simulink model "simulator_prototype_remade_v1"  (R2021b)
(part 6 of 14)

C_dq = ft_8({dq1,dq2,dq3,dq4,dq5,dq6,t1004,t1006,t1008,t1009,t101,t1010,t1012,t1013,t1016,t102,t1023,t1024,t1025,t1026,t1027,t1028,t1030,t1032,t1033,t1034,t1038,t1039,t1040,t1041,t1042,t1043,t1044,t1045,t1046,t1047,t1048,t1049,t1050,t1051,t1054,t1055,t1056,t1057,t1059,t1061,t1064,t1065,t1066,t1068,t1069,t1070,t1071,t1073,t1076,t1081,t1083,t1084,t1085,t1091,t1092,t1093,t1094,t1095,t1097,t1098,t1099,t110,t1101,t1102,t1105,t1106,t1107,t1108,t1109,t111,t1113,t1115,t1116,t1119,t112,t1120,t1122,t1123,t1125,t1126,t1127,t1128,t113,t1130,t1131,t1132,t1133,t1134,t1138,t1139,t114,t1140,t1141,t1144,t1146,t1148,t115,t1150,t1151,t1152,t1153,t1155,t1158,t1159,t116,t1161,t1162,t1163,t1166,t1167,t1169,t1170,t1171,t1173,t1174,t1175,t1176,t1177,t1178,t1179,t1180,t1181,t1182,t1183,t1184,t1185,t1186,t1187,t1188,t1189,t1190,t1191,t1192,t1193,t1195,t1196,t1197,t1198,t1199,t120,t1203,t1204,t1205,t1206,t1207,t1208,t121,t1210,t1215,t1219,t1221,t1222,t1223,t1224,t1225,t1226,t1227,t1228,t1229,t1230,t1232,t1233,t1236,t124,t1240,t1242,t1244,t1245,t125,t1250,t1251,t1253,t1254,t1256,t1257,t1258,t1259,t126,t1260,t1261,t1262,t1263,t1264,t1265,t1266,t1267,t1268,t1269,t1271,t1272,t1273,t1274,t1276,t1277,t1278,t1279,t128,t1280,t1282,t1285,t1286,t1287,t1288,t129,t1290,t1293,t1294,t1295,t1296,t1297,t1298,t130,t1300,t1301,t1302,t1306,t1307,t1308,t1309,t131,t1312,t1313,t1315,t1316,t1319,t132,t1320,t1321,t1322,t1323,t1324,t1325,t1326,t1328,t1329,t133,t1330,t1331,t1332,t1333,t1334,t1337,t1338,t1339,t134,t1340,t1341,t1342,t1343,t1344,t1345,t1346,t1347,t1348,t1351,t1352,t1353,t1354,t1355,t1356,t1358,t136,t1360,t1362,t1365,t1366,t1367,t1368,t1369,t1370,t1371,t1372,t1373,t1374,t1375,t1377,t1378,t1379,t1380,t1383,t1384,t1385,t1386,t1387,t1388,t1389,t139,t1391,t1392,t1393,t1394,t1397,t1398,t140,t1401,t1402,t1403,t1404,t1405,t1406,t1407,t1408,t1409,t141,t1410,t1411,t1413,t1414,t1415,t1416,t1417,t1418,t1419,t142,t1421,t1422,t1423,t1424,t1426,t1427,t1428,t1429,t143,t1430,t1431,t1432,t1433,t1434,t1436,t1439,t144,t1440,t1442,t1443,t1444,t1445,t1447,t1448,t1449,t145,t1451,t1452,t1453,t1454,t1455,t1456,t1457,t1458,t1459,t1460,t1463,t1464,t1467,t1468,t1469,t147,t1470,t1471,t1474,t1476,t1478,t1479,t148,t1480,t1481,t1482,t1483,t1485,t1486,t1487,t1488,t1489,t1492,t1494,t1496,t1498,t1499,t15,t150,t1501,t1503,t1505,t1506,t1508,t151,t1511,t1513,t1515,t1517,t1520,t1521,t1522,t1523,t1524,t1527,t1529,t153,t1530,t1531,t1532,t1533,t1534,t1535,t1536,t1537,t1538,t1539,t154,t1541,t1542,t1548,t1549,t1550,t1551,t1553,t1557,t1558,t156,t1560,t1561,t1562,t1566,t1567,t1568,t157,t1570,t1571,t1572,t1574,t1575,t1578,t158,t1580,t1581,t1587,t1589,t1590,t1591,t1592,t1593,t1594,t1595,t1596,t1597,t1598,t1599,t16,t1605,t1606,t1607,t1609,t161,t1610,t1611,t1612,t1613,t1614,t1615,t1617,t1618,t1619,t1620,t1621,t1622,t1624,t1625,t1627,t163,t1630,t1631,t1632,t1633,t1635,t1636,t1637,t1638,t1639,t1641,t1642,t1643,t1644,t1645,t1646,t1649,t165,t1651,t1652,t1653,t1657,t1658,t1659,t166,t1660,t1661,t1662,t1663,t1665,t1666,t1669,t1670,t1671,t1672,t1673,t1674,t1676,t1681,t1682,t1683,t1687,t1689,t1692,t1695,t1696,t1697,t1698,t17,t170,t1702,t1703,t1704,t1705,t1706,t1709,t171,t1711,t1712,t1713,t1716,t1719,t1720,t1722,t1724,t1726,t1728,t1729,t173,t1731,t1733,t1734,t1735,t1736,t1737,t1738,t1739,t1740,t1743,t1744,t1745,t1746,t1748,t1749,t175,t1752,t1755,t1756,t1757,t1758,t1759,t1760,t1761,t1763,t1764,t1767,t1769,t177,t1770,t1771,t1772,t1773,t1774,t1775,t1776,t1779,t1780,t1782,t1783,t1784,t1785,t1786,t1787,t1788,t1789,t1791,t1792,t1793,t1795,t1797,t1798,t1799,t18,t1800,t1801,t1802,t1804,t1806,t1807,t1808,t1809,t1810,t1811,t1812,t1813,t1814,t1816,t1817,t1820,t1822,t1823,t1824,t1825,t1826,t1827,t1828,t1829,t183,t1830,t1831,t1832,t1833,t1834,t1835,t1836,t1837,t1838,t1839,t1844,t1847,t1849,t185,t1850,t1851,t1854,t1855,t1857,t1858,t1859,t186,t1862,t1864,t1865,t1866,t1867,t1871,t1872,t1873,t1877,t1879,t1880,t1881,t1882,t1884,t1887,t1889,t1892,t1893,t1896,t19,t190,t1903,t1904,t1906,t1907,t1908,t1909,t191,t1910,t1911,t1912,t1913,t1914,t1915,t1916,t1919,t1920,t1921,t1925,t1926,t193,t1930,t1935,t1936,t1937,t1938,t1939,t1943,t1944,t1946,t1950,t1955,t196,t1961,t1966,t1967,t1968,t1969,t197,t1970,t1971,t1973,t1976,t1977,t1978,t1979,t1980,t1981,t1984,t1988,t199,t1992,t1993,t1994,t1995,t1996,t1997,t1998,t1999,t2,t20,t200,t2000,t2001,t2002,t2003,t2004,t2005,t2006,t2008,t201,t2014,t2016,t2017,t2019,t202,t2020,t2021,t2023,t2024,t2028,t2029,t2033,t2036,t2037,t2038,t204,t2040,t2041,t2042,t2044,t2047,t205,t2051,t2052,t2053,t2054,t2055,t2056,t2057,t2058,t2059,t206,t2060,t2061,t2062,t2065,t2066,t2067,t2068,t2069,t207,t2070,t2071,t2072,t2073,t2074,t2076,t2077,t2078,t2079,t2080,t2081,t2082,t2083,t2084,t2085,t2086,t2087,t2088,t2089,t2091,t2092,t2093,t2094,t2095,t2096,t2097,t2098,t2099,t21,t2100,t2101,t2103,t2104,t2105,t2106,t2107,t2108,t2109,t2110,t2111,t2113,t2114,t2115,t2116,t2117,t2118,t2119,t2121,t2125,t2128,t2129,t2130,t2131,t2132,t2133,t2135,t2136,t2139,t2140,t2141,t2142,t2144,t2147,t2148,t2149,t215,t2150,t2151,t2154,t2155,t2156,t2157,t2158,t2159,t2162,t2163,t2166,t2167,t2168,t2169,t2170,t2171,t2172,t2174,t2175,t2176,t2177,t2178,t2179,t2180,t2182,t2184,t2185,t2186,t2187,t2189,t2190,t2191,t2192,t2194,t2195,t2196,t22,t2200,t2201,t2203,t2204,t2208,t2209,t2210,t2212,t2214,t2217,t2218,t2219,t2220,t2221,t2223,t2225,t2227,t2228,t2229,t2231,t2232,t2236,t2237,t2239,t224,t2240,t2243,t2246,t2249,t225,t2250,t2251,t2252,t2254,t2255,t2256,t2257,t2264,t2265,t2266,t2267,t2269,t227,t2270,t2271,t2272,t2273,t2274,t2276,t2277,t2278,t2279,t228,t2280,t2281,t2282,t2283,t2284,t2285,t2286,t2287,t2291,t2292,t2294,t2295,t23,t230,t2302,t2304,t2305,t2306,t2307,t2308,t2309,t231,t2310,t2311,t2312,t2314,t2316,t2317,t2318,t2321,t2322,t2323,t2324,t233,t2331,t2333,t2334,t2335,t2336,t2337,t2338,t2339,t234,t2340,t2341,t2342,t2344,t2347,t2348,t235,t2350,t2351,t2355,t2357,t2358,t2359,t236,t2361,t2362,t2363,t2364,t2365,t2366,t2368,t2369,t2370,t2371,t2372,t2373,t2374,t2375,t2376,t2377,t2378,t2379,t2381,t2382,t2384,t2385,t2387,t2388,t2389,t239,t2390,t2391,t2392,t2394,t2395,t2396,t2397,t24,t240,t2400,t2401,t2402,t2403,t2405,t2406,t2407,t2410,t2417,t2421,t2422,t2423,t2425,t2427,t2428,t2429,t243,t2430,t2431,t2434,t2435,t2437,t2438,t2439,t244,t2440,t2441,t2442,t2443,t2444,t2445,t2446,t2449,t2450,t2452,t2453,t2454,t2455,t2456,t2457,t2458,t2459,t2460,t2461,t2463,t2464,t2466,t2467,t2469,t2470,t2471,t2472,t2474,t2477,t2478,t2480,t2481,t2482,t2483,t2484,t2485,t2486,t2487,t2489,t249,t2495,t2497,t25,t2500,t2502,t2503,t2505,t2506,t2507,t2508,t2509,t2510,t2511,t2512,t2513,t2517,t2518,t2519,t2520,t2521,t2522,t2523,t2524,t2525,t2526,t2527,t2530,t2531,t2532,t2533,t2535,t2536,t2537,t2539,t2540,t2541,t2543,t2544,t2545,t2546,t2548,t2549,t2550,t2552,t2553,t2554,t2555,t2556,t2560,t2562,t2563,t2564,t2565,t2566,t2567,t2568,t2569,t257,t2570,t2571,t2574,t2575,t2576,t2577,t2578,t2579,t258,t2580,t2581,t2582,t2585,t2586,t2587,t2588,t2589,t2590,t2595,t2597,t2598,t2599,t26,t2600,t2601,t2602,t2603,t2604,t2606,t2607,t2608,t2611,t2612,t2615,t2616,t2617,t2627,t263,t2633,t2634,t2636,t2639,t2640,t2641,t2654,t2655,t2656,t2659,t266,t2666,t2668,t2669,t2671,t2673,t2675,t2676,t2677,t2678,t2680,t2681,t2682,t2684,t2685,t2686,t2688,t2692,t2693,t2694,t2695,t2699,t270,t2702,t2703,t2705,t2706,t2707,t2708,t2719,t2720,t2721,t2722,t2723,t2724,t2725,t2726,t273,t2733,t2734,t2739,t274,t2741,t2742,t2743,t2744,t2748,t2749,t275,t2752,t2759,t276,t2760,t2761,t2762,t2764,t2768,t2769,t277,t2770,t2771,t2773,t2774,t2775,t2776,t278,t2781,t2782,t2783,t2784,t2786,t2787,t2788,t2789,t2791,t2792,t280,t2806,t2808,t2815,t2820,t2821,t2829,t2830,t2831,t284,t2840,t2842,t2844,t2845,t2847,t2848,t2849,t2853,t2854,t2861,t2862,t2863,t2864,t2866,t2868,t2869,t287,t2879,t2884,t2886,t2888,t2892,t2898,t2899,t29,t290,t2900,t2901,t2902,t2903,t2908,t291,t292,t2920,t2923,t2925,t2926,t2928,t2929,t2930,t2937,t294,t2940,t2943,t2945,t2948,t2949,t2950,t2951,t2952,t2960,t2961,t2962,t2963,t2964,t2966,t2967,t2968,t2969,t297,t2970,t2971,t2975,t2976,t2980,t2982,t2983,t2984,t2985,t2986,t2988,t2989,t299,t2991,t2992,t2993,t2996,t2997,t3,t30,t300,t3003,t3004,t3007,t3010,t3011,t3013,t3014,t3019,t302,t3020,t3021,t3023,t3024,t3025,t3027,t3028,t3029,t303,t3030,t3031,t3032,t3033,t3034,t3035,t3036,t3038,t3039,t304,t3043,t3045,t3046,t3047,t305,t3051,t3052,t3053,t3055,t3056,t3057,t306,t3060,t3061,t3062,t3063,t3065,t3066,t3069,t3070,t3071,t3072,t3073,t3075,t3077,t3078,t3079,t3080,t3082,t3083,t3085,t3087,t309,t3090,t3091,t3092,t3093,t3094,t3095,t3098,t3099,t310,t3103,t3104,t3105,t3108,t3109,t311,t3112,t3113,t3119,t3120,t3123,t3124,t3126,t3127,t313,t3130,t3131,t3132,t3133,t3139,t314,t3140,t3142,t3143,t3145,t3146,t3148,t3149,t315,t3150,t3151,t3152,t3156,t3157,t3158,t316,t3160,t3163,t3165,t3167,t3170,t3171,t3172,t3173,t3174,t3177,t3178,t318,t3180,t3182,t3183,t3184,t3186,t3187,t319,t3190,t3191,t3194,t3197,t3199,t320,t3206,t3207,t3208,t3218,t3219,t322,t3228,t3230,t3231,t3234,t3236,t324,t3240,t3241,t3242,t3243,t3244,t3245,t325,t3250,t3251,t3252,t3253,t3254,t3256,t3257,t3260,t3265,t3272,t3273,t3274,t3275,t3276,t3277,t3278,t3279,t328,t3280,t3282,t3283,t3284,t3285,t3286,t3287,t3288,t3289,t3290,t3291,t3292,t3293,t3295,t3296,t3297,t3298,t3299,t3301,t3302,t3303,t3304,t3306,t3307,t3308,t3309,t3310,t3312,t3313,t3314,t3315,t3317,t3318,t3320,t3321,t3324,t3325,t3326,t3327,t3328,t3329,t333,t3331,t3333,t3334,t3335,t3338,t3339,t3342,t3343,t3346,t3347,t3350,t336,t3362,t3363,t3364,t3365,t3366,t3367,t3368,t3369,t337,t3371,t3372,t3373,t3374,t3375,t3376,t3377,t3378,t3380,t3381,t3382,t3383,t3384,t3387,t3390,t3391,t3392,t3393,t3394,t3395,t3396,t3397,t3398,t3399,t34,t340,t3400,t3402,t3403,t3404,t3405,t3406,t3407,t3408,t3409,t3410,t3411,t3412,t3413,t3416,t3417,t3418,t3420,t3421,t3422,t3423,t3424,t3425,t3426,t3427,t3430,t3431,t3432,t3433,t3434,t3435,t3436,t3437,t3439,t344,t3440,t3441,t3442,t3443,t3444,t3445,t3446,t3447,t3449,t3450,t3453,t3454,t3455,t3456,t3457,t3458,t346,t3462,t3463,t3464,t3465,t3466,t3467,t3468,t3469,t347,t3470,t3471,t3472,t3473,t3474,t3475,t3476,t3479,t348,t3480,t3481,t3483,t3485,t3487,t3488,t3489,t349,t3490,t3491,t3492,t3493,t3494,t3496,t3497,t3498,t3499,t350,t3500,t3501,t3502,t3503,t3504,t3505,t3506,t3507,t3509,t3510,t3511,t3513,t3514,t3515,t3516,t3517,t3518,t352,t3521,t3522,t3523,t3527,t3528,t3529,t353,t3530,t3531,t3532,t3533,t3535,t3536,t3538,t3539,t3542,t3543,t3544,t3545,t3546,t3547,t3549,t3550,t3551,t3552,t3554,t3556,t3557,t3559,t356,t3560,t3562,t3563,t3564,t3567,t3568,t3569,t357,t3571,t3572,t3573,t3574,t3577,t3578,t358,t3582,t3583,t3584,t3585,t3586,t3587,t3589,t359,t3590,t3592,t3593,t3596,t3597,t3599,t3602,t3603,t3604,t3605,t3606,t3607,t3608,t3609,t361,t3610,t3611,t3612,t3614,t3615,t3616,t3617,t3618,t3619,t362,t3620,t3625,t3630,t3631,t3633,t3634,t3635,t3636,t3637,t3638,t3642,t3644,t3648,t365,t3652,t3653,t3654,t3655,t3656,t3657,t3658,t3659,t3660,t3662,t3663,t3666,t3667,t3668,t3676,t368,t3681,t3682,t3687,t3688,t369,t3690,t3691,t3693,t3694,t3695,t3696,t3697,t3699,t3700,t3701,t3702,t3704,t3705,t3706,t3707,t3708,t3709,t371,t3713,t3715,t3716,t3717,t372,t3720,t3721,t3723,t3724,t3725,t3726,t3728,t3729,t373,t3730,t3732,t3733,t3734,t3735,t3736,t3737,t3738,t374,t3743,t3744,t3745,t3746,t3747,t3750,t3752,t3756,t3757,t3758,t3766,t3768,t3769,t377,t3774,t3776,t3778,t378,t3780,t3783,t3784,t3785,t3786,t3787,t3789,t379,t3792,t3795,t3798,t380,t3800,t3803,t3804,t3805,t3806,t3810,t3811,t3813,t3814,t3815,t3816,t3817,t3819,t382,t3820,t3821,t3822,t3823,t3824,t3825,t3826,t3827,t3831,t3834,t3835,t3839,t384,t3843,t3849,t3850,t3851,t3852,t3853,t3855,t3857,t3858,t386,t3866,t3867,t3869,t387,t3870,t3877,t388,t3885,t3889,t3890,t3891,t3892,t3899,t391,t3912,t3913,t3915,t3917,t392,t3929,t3930,t3941,t3946,t3949,t395,t3950,t3951,t3952,t3953,t3958,t3959,t396,t3966,t3970,t3980,t3981,t3982,t3984,t3990,t4,t400,t4004,t4005,t4006,t401,t4010,t4011,t4014,t4015,t4016,t4017,t4018,t4019,t402,t4020,t4021,t4022,t4023,t4024,t4025,t4026,t4027,t4028,t4029,t403,t4036,t4039,t4040,t4041,t4042,t4045,t4046,t4047,t4048,t4051,t4053,t4054,t406,t4062,t4063,t4064,t4065,t4068,t4069,t4070,t4071,t4073,t4074,t4075,t4089,t4099,t410,t4103,t4105,t411,t4113,t4114,t4116,t4118,t4119,t412,t4123,t4124,t4125,t413,t4132,t414,t4140,t4142,t4143,t4144,t4145,t415,t4150,t4152,t4153,t416,t4162,t4164,t4165,t4166,t4169,t417,t4171,t4173,t4174,t4177,t4178,t4179,t418,t4180,t4181,t4183,t4184,t4185,t4186,t4188,t4190,t4195,t4196,t4197,t420,t4201,t4202,t4205,t4206,t4207,t4208,t4209,t4210,t4211,t4215,t4217,t4218,t4219,t422,t4220,t4221,t4223,t4224,t4225,t4226,t4228,t4229,t423,t4230,t4231,t4232,t4233,t4234,t4235,t424,t4241,t4242,t4243,t4244,t4245,t4246,t4247,t4248,t4249,t425,t4250,t4251,t4253,t4254,t4255,t4256,t4257,t4258,t4259,t4260,t4261,t4262,t4263,t427,t4273,t4274,t4275,t4276,t4278,t4279,t428,t4280,t4281,t4282,t4283,t4284,t4285,t4286,t4287,t4289,t429,t4290,t4291,t4292,t4293,t4295,t4296,t4297,t4298,t4299,t4300,t4301,t4302,t4303,t4304,t4305,t4306,t4308,t431,t4310,t4315,t4316,t4317,t4318,t432,t4321,t4323,t4324,t4325,t4326,t4327,t4328,t4329,t433,t4330,t4331,t4332,t4333,t4334,t4335,t4336,t4337,t4338,t4339,t434,t4340,t4342,t4344,t4345,t4346,t4347,t4348,t4349,t435,t4350,t4354,t4356,t4357,t436,t4362,t4363,t4365,t4366,t4368,t4369,t437,t4370,t4371,t4372,t4373,t4374,t4375,t4376,t4377,t4379,t438,t4380,t4382,t4383,t4384,t4385,t4386,t4387,t4388,t4389,t439,t4391,t4392,t4394,t4395,t4396,t4397,t4398,t4399,t44,t440,t4400,t4401,t4402,t4403,t4404,t4405,t4406,t4407,t4408,t4409,t441,t4410,t4411,t4412,t4413,t4414,t4415,t4416,t4417,t4418,t4419,t442,t4420,t4421,t4422,t4423,t4424,t4425,t4426,t4427,t4428,t4429,t4430,t4431,t4432,t4433,t4434,t4435,t4436,t4437,t4438,t4439,t444,t4440,t4442,t4443,t4444,t4445,t4446,t4447,t4448,t4449,t445,t4450,t4451,t4452,t4453,t4454,t4455,t4457,t4459,t4460,t4461,t4462,t4463,t4464,t4465,t4466,t4467,t4468,t4469,t4470,t4471,t4473,t4474,t4475,t4476,t4477,t4478,t4479,t448,t4480,t4481,t4482,t4483,t4484,t4485,t4486,t4487,t4488,t4489,t449,t4490,t4491,t4492,t4493,t4495,t4498,t45,t450,t4501,t4502,t4504,t4506,t4508,t4509,t4513,t4516,t4517,t4519,t452,t4520,t4522,t4524,t4525,t453,t4530,t4532,t4533,t454,t4540,t4542,t4543,t4547,t4548,t4549,t4551,t4554,t4555,t4557,t4558,t4559,t4561,t4562,t4563,t4566,t4567,t4568,t4569,t457,t4570,t4571,t4572,t4574,t4575,t4577,t4579,t458,t4581,t4582,t4583,t4584,t4588,t4589,t459,t4590,t4591,t4595,t4596,t46,t460,t4600,t4601,t4605,t4606,t4607,t461,t4611,t4614,t4616,t4617,t462,t4621,t4622,t4625,t4626,t4628,t4629,t463,t4630,t4632,t4633,t4634,t4636,t4637,t4638,t4639,t464,t4640,t4641,t4642,t4643,t4644,t4645,t4646,t4647,t4649,t465,t4650,t4651,t4652,t4653,t4656,t4657,t4658,t466,t4660,t4661,t4662,t4663,t4666,t4667,t4669,t4672,t4673,t4674,t4675,t468,t4688,t469,t4691,t4692,t4693,t4694,t4695,t4696,t4697,t47,t470,t4707,t4708,t4709,t471,t4711,t4713,t4716,t472,t4722,t4723,t4724,t4725,t4726,t4727,t4728,t4731,t4732,t4733,t4734,t4737,t4740,t4741,t4742,t4745,t4747,t4748,t4749,t475,t4752,t4753,t4754,t4755,t4756,t4758,t4759,t4760,t4761,t4763,t4766,t4769,t477,t4770,t4777,t4778,t4782,t4783,t4785,t4786,t4788,t4789,t479,t4790,t4794,t4795,t4796,t4797,t4798,t4799,t480,t4800,t4801,t4803,t4804,t4805,t4807,t4808,t481,t4811,t4813,t4814,t4815,t4818,t482,t4820,t4824,t4825,t4827,t4828,t483,t4830,t4832,t4833,t4834,t4835,t4837,t4839,t484,t4841,t4842,t4845,t4846,t4849,t485,t4852,t486,t4861,t4862,t4864,t4865,t4866,t4867,t4871,t4872,t4873,t4876,t4877,t4878,t4879,t488,t4882,t4883,t4884,t4886,t4887,t489,t4895,t4897,t4899,t4900,t4908,t4909,t491,t4910,t4911,t4913,t4915,t4916,t4919,t492,t4920,t4923,t4924,t4925,t4927,t4928,t493,t4930,t4933,t4934,t4937,t4938,t494,t4941,t4942,t4943,t4944,t4945,t4946,t4948,t4951,t4955,t4956,t4957,t496,t4962,t4964,t4969,t497,t4970,t4973,t4974,t4976,t498,t4980,t4981,t4982,t4983,t4986,t4987,t4988,t499,t4991,t4993,t4996,t4998,t4999,t5,t50,t500,t5000,t5001,t5004,t5006,t5008,t501,t5019,t502,t5021,t5022,t5023,t5026,t5027,t5029,t503,t5034,t5035,t5036,t5038,t504,t5045,t5046,t505,t5051,t5052,t5053,t506,t5060,t5062,t5063,t5064,t5065,t5066,t5069,t507,t5071,t5072,t5073,t5078,t508,t5080,t5082,t5083,t5084,t5085,t509,t5091,t5093,t5095,t5096,t5097,t5098,t5099,t510,t5100,t5102,t5107,t511,t5111,t5112,t5113,t5114,t5116,t5119,t512,t5120,t5122,t5127,t513,t5130,t5139,t514,t5142,t5147,t5149,t5150,t5151,t5154,t5158,t516,t5165,t517,t5171,t5172,t5176,t5179,t518,t5180,t5181,t5183,t5184,t5185,t5186,t5187,t5192,t5193,t5199,t520,t5200,t5203,t5204,t5205,t5208,t521,t5215,t5216,t5217,t522,t5222,t5223,t5224,t5227,t523,t5236,t5237,t5238,t5239,t524,t5240,t5244,t5245,t525,t5250,t5252,t5258,t526,t5267,t527,t5270,t5271,t5279,t528,t5280,t5281,t5285,t529,t5293,t5294,t53,t530,t5305,t531,t5318,t5319,t532,t5321,t5324,t5325,t5327,t5328,t533,t5331,t5332,t534,t535,t5353,t5355,t5356,t5358,t536,t5361,t5362,t5364,t5368,t537,t5372,t5373,t5376,t5378,t538,t5387,t5389,t539,t5390,t5391,t5392,t5393,t5394,t540,t5402,t5404,t5409,t5416,t5420,t5424,t5429,t543,t5430,t5434,t5435,t5436,t5439,t544,t5440,t5441,t5445,t5449,t545,t5450,t5451,t5452,t5453,t5455,t5456,t5457,t546,t5467,t5468,t5469,t547,t5470,t5471,t5472,t5473,t5474,t5475,t5476,t5477,t5478,t548,t5489,t549,t5490,t5493,t5494,t5497,t5499,t5501,t5508,t551,t5510,t5512,t5516,t5517,t552,t5521,t553,t5532,t5535,t554,t5540,t5547,t555,t5557,t5558,t556,t557,t5574,t5578,t5579,t558,t5582,t5586,t559,t5590,t5593,t5596,t560,t5604,t5607,t561,t5612,t562,t5629,t563,t5634,t5635,t564,t567,t568,t5688,t569,t57,t570,t571,t572,t573,t574,t5741,t5743,t576,t577,t5777,t5779,t578,t5780,t5782,t579,t58,t580,t581,t582,t5826,t583,t584,t586,t587,t5886,t5887,t589,t5894,t59,t590,t591,t592,t593,t594,t595,t596,t597,t6,t60,t600,t602,t603,t604,t605,t609,t610,t611,t612,t613,t614,t615,t616,t618,t619,t622,t623,t624,t625,t626,t627,t628,t629,t63,t630,t631,t633,t634,t635,t636,t637,t638,t639,t640,t641,t642,t643,t648,t649,t650,t653,t654,t655,t656,t657,t658,t660,t662,t663,t664,t665,t667,t668,t673,t674,t675,t676,t678,t679,t681,t682,t683,t684,t685,t686,t687,t688,t689,t693,t694,t695,t696,t697,t698,t7,t700,t702,t703,t704,t705,t706,t71,t710,t711,t712,t713,t715,t716,t72,t724,t728,t73,t731,t733,t734,t735,t736,t74,t741,t742,t743,t744,t746,t747,t748,t749,t75,t750,t751,t752,t754,t755,t756,t757,t758,t759,t76,t760,t762,t763,t764,t765,t766,t767,t768,t769,t77,t772,t773,t774,t775,t776,t777,t778,t779,t780,t781,t782,t784,t785,t786,t790,t792,t794,t795,t796,t798,t8,t80,t801,t804,t805,t806,t808,t81,t814,t815,t817,t82,t820,t822,t825,t827,t83,t831,t832,t833,t834,t835,t836,t837,t838,t84,t840,t841,t842,t843,t846,t86,t863,t868,t869,t870,t874,t878,t880,t881,t882,t884,t885,t888,t889,t891,t892,t895,t899,t9,t90,t900,t903,t906,t91,t911,t921,t922,t923,t925,t926,t927,t929,t934,t935,t936,t937,t940,t941,t942,t946,t949,t95,t950,t954,t955,t957,t958,t961,t962,t964,t965,t968,t97,t970,t971,t972,t973,t975,t977,t982,t983,t984,t986,t987,t988,t989,t99,t993,t994,t995,t999});
end
function C_dq = ft_8(ct)
dq1 = ct{1};
dq2 = ct{2};
dq3 = ct{3};
dq4 = ct{4};
dq5 = ct{5};
dq6 = ct{6};
t1004 = ct{7};
t1006 = ct{8};
t1008 = ct{9};
t1009 = ct{10};
t101 = ct{11};
t1010 = ct{12};
t1012 = ct{13};
t1013 = ct{14};
t1016 = ct{15};
t102 = ct{16};
t1023 = ct{17};
t1024 = ct{18};
t1025 = ct{19};
t1026 = ct{20};
t1027 = ct{21};
t1028 = ct{22};
t1030 = ct{23};
t1032 = ct{24};
t1033 = ct{25};
t1034 = ct{26};
t1038 = ct{27};
t1039 = ct{28};
t1040 = ct{29};
t1041 = ct{30};
t1042 = ct{31};
t1043 = ct{32};
t1044 = ct{33};
t1045 = ct{34};
t1046 = ct{35};
t1047 = ct{36};
t1048 = ct{37};
t1049 = ct{38};
t1050 = ct{39};
t1051 = ct{40};
t1054 = ct{41};
t1055 = ct{42};
t1056 = ct{43};
t1057 = ct{44};
t1059 = ct{45};
t1061 = ct{46};
t1064 = ct{47};
t1065 = ct{48};
t1066 = ct{49};
t1068 = ct{50};
t1069 = ct{51};
t1070 = ct{52};
t1071 = ct{53};
t1073 = ct{54};
t1076 = ct{55};
t1081 = ct{56};
t1083 = ct{57};
t1084 = ct{58};
t1085 = ct{59};
t1091 = ct{60};
t1092 = ct{61};
t1093 = ct{62};
t1094 = ct{63};
t1095 = ct{64};
t1097 = ct{65};
t1098 = ct{66};
t1099 = ct{67};
t110 = ct{68};
t1101 = ct{69};
t1102 = ct{70};
t1105 = ct{71};
t1106 = ct{72};
t1107 = ct{73};
t1108 = ct{74};
t1109 = ct{75};
t111 = ct{76};
t1113 = ct{77};
t1115 = ct{78};
t1116 = ct{79};
t1119 = ct{80};
t112 = ct{81};
t1120 = ct{82};
t1122 = ct{83};
t1123 = ct{84};
t1125 = ct{85};
t1126 = ct{86};
t1127 = ct{87};
t1128 = ct{88};
t113 = ct{89};
t1130 = ct{90};
t1131 = ct{91};
t1132 = ct{92};
t1133 = ct{93};
t1134 = ct{94};
t1138 = ct{95};
t1139 = ct{96};
t114 = ct{97};
t1140 = ct{98};
t1141 = ct{99};
t1144 = ct{100};
t1146 = ct{101};
t1148 = ct{102};
t115 = ct{103};
t1150 = ct{104};
t1151 = ct{105};
t1152 = ct{106};
t1153 = ct{107};
t1155 = ct{108};
t1158 = ct{109};
t1159 = ct{110};
t116 = ct{111};
t1161 = ct{112};
t1162 = ct{113};
t1163 = ct{114};
t1166 = ct{115};
t1167 = ct{116};
t1169 = ct{117};
t1170 = ct{118};
t1171 = ct{119};
t1173 = ct{120};
t1174 = ct{121};
t1175 = ct{122};
t1176 = ct{123};
t1177 = ct{124};
t1178 = ct{125};
t1179 = ct{126};
t1180 = ct{127};
t1181 = ct{128};
t1182 = ct{129};
t1183 = ct{130};
t1184 = ct{131};
t1185 = ct{132};
t1186 = ct{133};
t1187 = ct{134};
t1188 = ct{135};
t1189 = ct{136};
t1190 = ct{137};
t1191 = ct{138};
t1192 = ct{139};
t1193 = ct{140};
t1195 = ct{141};
t1196 = ct{142};
t1197 = ct{143};
t1198 = ct{144};
t1199 = ct{145};
t120 = ct{146};
t1203 = ct{147};
t1204 = ct{148};
t1205 = ct{149};
t1206 = ct{150};
t1207 = ct{151};
t1208 = ct{152};
t121 = ct{153};
t1210 = ct{154};
t1215 = ct{155};
t1219 = ct{156};
t1221 = ct{157};
t1222 = ct{158};
t1223 = ct{159};
t1224 = ct{160};
t1225 = ct{161};
t1226 = ct{162};
t1227 = ct{163};
t1228 = ct{164};
t1229 = ct{165};
t1230 = ct{166};
t1232 = ct{167};
t1233 = ct{168};
t1236 = ct{169};
t124 = ct{170};
t1240 = ct{171};
t1242 = ct{172};
t1244 = ct{173};
t1245 = ct{174};
t125 = ct{175};
t1250 = ct{176};
t1251 = ct{177};
t1253 = ct{178};
t1254 = ct{179};
t1256 = ct{180};
t1257 = ct{181};
t1258 = ct{182};
t1259 = ct{183};
t126 = ct{184};
t1260 = ct{185};
t1261 = ct{186};
t1262 = ct{187};
t1263 = ct{188};
t1264 = ct{189};
t1265 = ct{190};
t1266 = ct{191};
t1267 = ct{192};
t1268 = ct{193};
t1269 = ct{194};
t1271 = ct{195};
t1272 = ct{196};
t1273 = ct{197};
t1274 = ct{198};
t1276 = ct{199};
t1277 = ct{200};
t1278 = ct{201};
t1279 = ct{202};
t128 = ct{203};
t1280 = ct{204};
t1282 = ct{205};
t1285 = ct{206};
t1286 = ct{207};
t1287 = ct{208};
t1288 = ct{209};
t129 = ct{210};
t1290 = ct{211};
t1293 = ct{212};
t1294 = ct{213};
t1295 = ct{214};
t1296 = ct{215};
t1297 = ct{216};
t1298 = ct{217};
t130 = ct{218};
t1300 = ct{219};
t1301 = ct{220};
t1302 = ct{221};
t1306 = ct{222};
t1307 = ct{223};
t1308 = ct{224};
t1309 = ct{225};
t131 = ct{226};
t1312 = ct{227};
t1313 = ct{228};
t1315 = ct{229};
t1316 = ct{230};
t1319 = ct{231};
t132 = ct{232};
t1320 = ct{233};
t1321 = ct{234};
t1322 = ct{235};
t1323 = ct{236};
t1324 = ct{237};
t1325 = ct{238};
t1326 = ct{239};
t1328 = ct{240};
t1329 = ct{241};
t133 = ct{242};
t1330 = ct{243};
t1331 = ct{244};
t1332 = ct{245};
t1333 = ct{246};
t1334 = ct{247};
t1337 = ct{248};
t1338 = ct{249};
t1339 = ct{250};
t134 = ct{251};
t1340 = ct{252};
t1341 = ct{253};
t1342 = ct{254};
t1343 = ct{255};
t1344 = ct{256};
t1345 = ct{257};
t1346 = ct{258};
t1347 = ct{259};
t1348 = ct{260};
t1351 = ct{261};
t1352 = ct{262};
t1353 = ct{263};
t1354 = ct{264};
t1355 = ct{265};
t1356 = ct{266};
t1358 = ct{267};
t136 = ct{268};
t1360 = ct{269};
t1362 = ct{270};
t1365 = ct{271};
t1366 = ct{272};
t1367 = ct{273};
t1368 = ct{274};
t1369 = ct{275};
t1370 = ct{276};
t1371 = ct{277};
t1372 = ct{278};
t1373 = ct{279};
t1374 = ct{280};
t1375 = ct{281};
t1377 = ct{282};
t1378 = ct{283};
t1379 = ct{284};
t1380 = ct{285};
t1383 = ct{286};
t1384 = ct{287};
t1385 = ct{288};
t1386 = ct{289};
t1387 = ct{290};
t1388 = ct{291};
t1389 = ct{292};
t139 = ct{293};
t1391 = ct{294};
t1392 = ct{295};
t1393 = ct{296};
t1394 = ct{297};
t1397 = ct{298};
t1398 = ct{299};
t140 = ct{300};
t1401 = ct{301};
t1402 = ct{302};
t1403 = ct{303};
t1404 = ct{304};
t1405 = ct{305};
t1406 = ct{306};
t1407 = ct{307};
t1408 = ct{308};
t1409 = ct{309};
t141 = ct{310};
t1410 = ct{311};
t1411 = ct{312};
t1413 = ct{313};
t1414 = ct{314};
t1415 = ct{315};
t1416 = ct{316};
t1417 = ct{317};
t1418 = ct{318};
t1419 = ct{319};
t142 = ct{320};
t1421 = ct{321};
t1422 = ct{322};
t1423 = ct{323};
t1424 = ct{324};
t1426 = ct{325};
t1427 = ct{326};
t1428 = ct{327};
t1429 = ct{328};
t143 = ct{329};
t1430 = ct{330};
t1431 = ct{331};
t1432 = ct{332};
t1433 = ct{333};
t1434 = ct{334};
t1436 = ct{335};
t1439 = ct{336};
t144 = ct{337};
t1440 = ct{338};
t1442 = ct{339};
t1443 = ct{340};
t1444 = ct{341};
t1445 = ct{342};
t1447 = ct{343};
t1448 = ct{344};
t1449 = ct{345};
t145 = ct{346};
t1451 = ct{347};
t1452 = ct{348};
t1453 = ct{349};
t1454 = ct{350};
t1455 = ct{351};
t1456 = ct{352};
t1457 = ct{353};
t1458 = ct{354};
t1459 = ct{355};
t1460 = ct{356};
t1463 = ct{357};
t1464 = ct{358};
t1467 = ct{359};
t1468 = ct{360};
t1469 = ct{361};
t147 = ct{362};
t1470 = ct{363};
t1471 = ct{364};
t1474 = ct{365};
t1476 = ct{366};
t1478 = ct{367};
t1479 = ct{368};
t148 = ct{369};
t1480 = ct{370};
t1481 = ct{371};
t1482 = ct{372};
t1483 = ct{373};
t1485 = ct{374};
t1486 = ct{375};
t1487 = ct{376};
t1488 = ct{377};
t1489 = ct{378};
t1492 = ct{379};
t1494 = ct{380};
t1496 = ct{381};
t1498 = ct{382};
t1499 = ct{383};
t15 = ct{384};
t150 = ct{385};
t1501 = ct{386};
t1503 = ct{387};
t1505 = ct{388};
t1506 = ct{389};
t1508 = ct{390};
t151 = ct{391};
t1511 = ct{392};
t1513 = ct{393};
t1515 = ct{394};
t1517 = ct{395};
t1520 = ct{396};
t1521 = ct{397};
t1522 = ct{398};
t1523 = ct{399};
t1524 = ct{400};
t1527 = ct{401};
t1529 = ct{402};
t153 = ct{403};
t1530 = ct{404};
t1531 = ct{405};
t1532 = ct{406};
t1533 = ct{407};
t1534 = ct{408};
t1535 = ct{409};
t1536 = ct{410};
t1537 = ct{411};
t1538 = ct{412};
t1539 = ct{413};
t154 = ct{414};
t1541 = ct{415};
t1542 = ct{416};
t1548 = ct{417};
t1549 = ct{418};
t1550 = ct{419};
t1551 = ct{420};
t1553 = ct{421};
t1557 = ct{422};
t1558 = ct{423};
t156 = ct{424};
t1560 = ct{425};
t1561 = ct{426};
t1562 = ct{427};
t1566 = ct{428};
t1567 = ct{429};
t1568 = ct{430};
t157 = ct{431};
t1570 = ct{432};
t1571 = ct{433};
t1572 = ct{434};
t1574 = ct{435};
t1575 = ct{436};
t1578 = ct{437};
t158 = ct{438};
t1580 = ct{439};
t1581 = ct{440};
t1587 = ct{441};
t1589 = ct{442};
t1590 = ct{443};
t1591 = ct{444};
t1592 = ct{445};
t1593 = ct{446};
t1594 = ct{447};
t1595 = ct{448};
t1596 = ct{449};
t1597 = ct{450};
t1598 = ct{451};
t1599 = ct{452};
t16 = ct{453};
t1605 = ct{454};
t1606 = ct{455};
t1607 = ct{456};
t1609 = ct{457};
t161 = ct{458};
t1610 = ct{459};
t1611 = ct{460};
t1612 = ct{461};
t1613 = ct{462};
t1614 = ct{463};
t1615 = ct{464};
t1617 = ct{465};
t1618 = ct{466};
t1619 = ct{467};
t1620 = ct{468};
t1621 = ct{469};
t1622 = ct{470};
t1624 = ct{471};
t1625 = ct{472};
t1627 = ct{473};
t163 = ct{474};
t1630 = ct{475};
t1631 = ct{476};
t1632 = ct{477};
t1633 = ct{478};
t1635 = ct{479};
t1636 = ct{480};
t1637 = ct{481};
t1638 = ct{482};
t1639 = ct{483};
t1641 = ct{484};
t1642 = ct{485};
t1643 = ct{486};
t1644 = ct{487};
t1645 = ct{488};
t1646 = ct{489};
t1649 = ct{490};
t165 = ct{491};
t1651 = ct{492};
t1652 = ct{493};
t1653 = ct{494};
t1657 = ct{495};
t1658 = ct{496};
t1659 = ct{497};
t166 = ct{498};
t1660 = ct{499};
t1661 = ct{500};
t1662 = ct{501};
t1663 = ct{502};
t1665 = ct{503};
t1666 = ct{504};
t1669 = ct{505};
t1670 = ct{506};
t1671 = ct{507};
t1672 = ct{508};
t1673 = ct{509};
t1674 = ct{510};
t1676 = ct{511};
t1681 = ct{512};
t1682 = ct{513};
t1683 = ct{514};
t1687 = ct{515};
t1689 = ct{516};
t1692 = ct{517};
t1695 = ct{518};
t1696 = ct{519};
t1697 = ct{520};
t1698 = ct{521};
t17 = ct{522};
t170 = ct{523};
t1702 = ct{524};
t1703 = ct{525};
t1704 = ct{526};
t1705 = ct{527};
t1706 = ct{528};
t1709 = ct{529};
t171 = ct{530};
t1711 = ct{531};
t1712 = ct{532};
t1713 = ct{533};
t1716 = ct{534};
t1719 = ct{535};
t1720 = ct{536};
t1722 = ct{537};
t1724 = ct{538};
t1726 = ct{539};
t1728 = ct{540};
t1729 = ct{541};
t173 = ct{542};
t1731 = ct{543};
t1733 = ct{544};
t1734 = ct{545};
t1735 = ct{546};
t1736 = ct{547};
t1737 = ct{548};
t1738 = ct{549};
t1739 = ct{550};
t1740 = ct{551};
t1743 = ct{552};
t1744 = ct{553};
t1745 = ct{554};
t1746 = ct{555};
t1748 = ct{556};
t1749 = ct{557};
t175 = ct{558};
t1752 = ct{559};
t1755 = ct{560};
t1756 = ct{561};
t1757 = ct{562};
t1758 = ct{563};
t1759 = ct{564};
t1760 = ct{565};
t1761 = ct{566};
t1763 = ct{567};
t1764 = ct{568};
t1767 = ct{569};
t1769 = ct{570};
t177 = ct{571};
t1770 = ct{572};
t1771 = ct{573};
t1772 = ct{574};
t1773 = ct{575};
t1774 = ct{576};
t1775 = ct{577};
t1776 = ct{578};
t1779 = ct{579};
t1780 = ct{580};
t1782 = ct{581};
t1783 = ct{582};
t1784 = ct{583};
t1785 = ct{584};
t1786 = ct{585};
t1787 = ct{586};
t1788 = ct{587};
t1789 = ct{588};
t1791 = ct{589};
t1792 = ct{590};
t1793 = ct{591};
t1795 = ct{592};
t1797 = ct{593};
t1798 = ct{594};
t1799 = ct{595};
t18 = ct{596};
t1800 = ct{597};
t1801 = ct{598};
t1802 = ct{599};
t1804 = ct{600};
t1806 = ct{601};
t1807 = ct{602};
t1808 = ct{603};
t1809 = ct{604};
t1810 = ct{605};
t1811 = ct{606};
t1812 = ct{607};
t1813 = ct{608};
t1814 = ct{609};
t1816 = ct{610};
t1817 = ct{611};
t1820 = ct{612};
t1822 = ct{613};
t1823 = ct{614};
t1824 = ct{615};
t1825 = ct{616};
t1826 = ct{617};
t1827 = ct{618};
t1828 = ct{619};
t1829 = ct{620};
t183 = ct{621};
t1830 = ct{622};
t1831 = ct{623};
t1832 = ct{624};
t1833 = ct{625};
t1834 = ct{626};
t1835 = ct{627};
t1836 = ct{628};
t1837 = ct{629};
t1838 = ct{630};
t1839 = ct{631};
t1844 = ct{632};
t1847 = ct{633};
t1849 = ct{634};
t185 = ct{635};
t1850 = ct{636};
t1851 = ct{637};
t1854 = ct{638};
t1855 = ct{639};
t1857 = ct{640};
t1858 = ct{641};
t1859 = ct{642};
t186 = ct{643};
t1862 = ct{644};
t1864 = ct{645};
t1865 = ct{646};
t1866 = ct{647};
t1867 = ct{648};
t1871 = ct{649};
t1872 = ct{650};
t1873 = ct{651};
t1877 = ct{652};
t1879 = ct{653};
t1880 = ct{654};
t1881 = ct{655};
t1882 = ct{656};
t1884 = ct{657};
t1887 = ct{658};
t1889 = ct{659};
t1892 = ct{660};
t1893 = ct{661};
t1896 = ct{662};
t19 = ct{663};
t190 = ct{664};
t1903 = ct{665};
t1904 = ct{666};
t1906 = ct{667};
t1907 = ct{668};
t1908 = ct{669};
t1909 = ct{670};
t191 = ct{671};
t1910 = ct{672};
t1911 = ct{673};
t1912 = ct{674};
t1913 = ct{675};
t1914 = ct{676};
t1915 = ct{677};
t1916 = ct{678};
t1919 = ct{679};
t1920 = ct{680};
t1921 = ct{681};
t1925 = ct{682};
t1926 = ct{683};
t193 = ct{684};
t1930 = ct{685};
t1935 = ct{686};
t1936 = ct{687};
t1937 = ct{688};
t1938 = ct{689};
t1939 = ct{690};
t1943 = ct{691};
t1944 = ct{692};
t1946 = ct{693};
t1950 = ct{694};
t1955 = ct{695};
t196 = ct{696};
t1961 = ct{697};
t1966 = ct{698};
t1967 = ct{699};
t1968 = ct{700};
t1969 = ct{701};
t197 = ct{702};
t1970 = ct{703};
t1971 = ct{704};
t1973 = ct{705};
t1976 = ct{706};
t1977 = ct{707};
t1978 = ct{708};
t1979 = ct{709};
t1980 = ct{710};
t1981 = ct{711};
t1984 = ct{712};
t1988 = ct{713};
t199 = ct{714};
t1992 = ct{715};
t1993 = ct{716};
t1994 = ct{717};
t1995 = ct{718};
t1996 = ct{719};
t1997 = ct{720};
t1998 = ct{721};
t1999 = ct{722};
t2 = ct{723};
t20 = ct{724};
t200 = ct{725};
t2000 = ct{726};
t2001 = ct{727};
t2002 = ct{728};
t2003 = ct{729};
t2004 = ct{730};
t2005 = ct{731};
t2006 = ct{732};
t2008 = ct{733};
t201 = ct{734};
t2014 = ct{735};
t2016 = ct{736};
t2017 = ct{737};
t2019 = ct{738};
t202 = ct{739};
t2020 = ct{740};
t2021 = ct{741};
t2023 = ct{742};
t2024 = ct{743};
t2028 = ct{744};
t2029 = ct{745};
t2033 = ct{746};
t2036 = ct{747};
t2037 = ct{748};
t2038 = ct{749};
t204 = ct{750};
t2040 = ct{751};
t2041 = ct{752};
t2042 = ct{753};
t2044 = ct{754};
t2047 = ct{755};
t205 = ct{756};
t2051 = ct{757};
t2052 = ct{758};
t2053 = ct{759};
t2054 = ct{760};
t2055 = ct{761};
t2056 = ct{762};
t2057 = ct{763};
t2058 = ct{764};
t2059 = ct{765};
t206 = ct{766};
t2060 = ct{767};
t2061 = ct{768};
t2062 = ct{769};
t2065 = ct{770};
t2066 = ct{771};
t2067 = ct{772};
t2068 = ct{773};
t2069 = ct{774};
t207 = ct{775};
t2070 = ct{776};
t2071 = ct{777};
t2072 = ct{778};
t2073 = ct{779};
t2074 = ct{780};
t2076 = ct{781};
t2077 = ct{782};
t2078 = ct{783};
t2079 = ct{784};
t2080 = ct{785};
t2081 = ct{786};
t2082 = ct{787};
t2083 = ct{788};
t2084 = ct{789};
t2085 = ct{790};
t2086 = ct{791};
t2087 = ct{792};
t2088 = ct{793};
t2089 = ct{794};
t2091 = ct{795};
t2092 = ct{796};
t2093 = ct{797};
t2094 = ct{798};
t2095 = ct{799};
t2096 = ct{800};
t2097 = ct{801};
t2098 = ct{802};
t2099 = ct{803};
t21 = ct{804};
t2100 = ct{805};
t2101 = ct{806};
t2103 = ct{807};
t2104 = ct{808};
t2105 = ct{809};
t2106 = ct{810};
t2107 = ct{811};
t2108 = ct{812};
t2109 = ct{813};
t2110 = ct{814};
t2111 = ct{815};
t2113 = ct{816};
t2114 = ct{817};
t2115 = ct{818};
t2116 = ct{819};
t2117 = ct{820};
t2118 = ct{821};
t2119 = ct{822};
t2121 = ct{823};
t2125 = ct{824};
t2128 = ct{825};
t2129 = ct{826};
t2130 = ct{827};
t2131 = ct{828};
t2132 = ct{829};
t2133 = ct{830};
t2135 = ct{831};
t2136 = ct{832};
t2139 = ct{833};
t2140 = ct{834};
t2141 = ct{835};
t2142 = ct{836};
t2144 = ct{837};
t2147 = ct{838};
t2148 = ct{839};
t2149 = ct{840};
t215 = ct{841};
t2150 = ct{842};
t2151 = ct{843};
t2154 = ct{844};
t2155 = ct{845};
t2156 = ct{846};
t2157 = ct{847};
t2158 = ct{848};
t2159 = ct{849};
t2162 = ct{850};
t2163 = ct{851};
t2166 = ct{852};
t2167 = ct{853};
t2168 = ct{854};
t2169 = ct{855};
t2170 = ct{856};
t2171 = ct{857};
t2172 = ct{858};
t2174 = ct{859};
t2175 = ct{860};
t2176 = ct{861};
t2177 = ct{862};
t2178 = ct{863};
t2179 = ct{864};
t2180 = ct{865};
t2182 = ct{866};
t2184 = ct{867};
t2185 = ct{868};
t2186 = ct{869};
t2187 = ct{870};
t2189 = ct{871};
t2190 = ct{872};
t2191 = ct{873};
t2192 = ct{874};
t2194 = ct{875};
t2195 = ct{876};
t2196 = ct{877};
t22 = ct{878};
t2200 = ct{879};
t2201 = ct{880};
t2203 = ct{881};
t2204 = ct{882};
t2208 = ct{883};
t2209 = ct{884};
t2210 = ct{885};
t2212 = ct{886};
t2214 = ct{887};
t2217 = ct{888};
t2218 = ct{889};
t2219 = ct{890};
t2220 = ct{891};
t2221 = ct{892};
t2223 = ct{893};
t2225 = ct{894};
t2227 = ct{895};
t2228 = ct{896};
t2229 = ct{897};
t2231 = ct{898};
t2232 = ct{899};
t2236 = ct{900};
t2237 = ct{901};
t2239 = ct{902};
t224 = ct{903};
t2240 = ct{904};
t2243 = ct{905};
t2246 = ct{906};
t2249 = ct{907};
t225 = ct{908};
t2250 = ct{909};
t2251 = ct{910};
t2252 = ct{911};
t2254 = ct{912};
t2255 = ct{913};
t2256 = ct{914};
t2257 = ct{915};
t2264 = ct{916};
t2265 = ct{917};
t2266 = ct{918};
t2267 = ct{919};
t2269 = ct{920};
t227 = ct{921};
t2270 = ct{922};
t2271 = ct{923};
t2272 = ct{924};
t2273 = ct{925};
t2274 = ct{926};
t2276 = ct{927};
t2277 = ct{928};
t2278 = ct{929};
t2279 = ct{930};
t228 = ct{931};
t2280 = ct{932};
t2281 = ct{933};
t2282 = ct{934};
t2283 = ct{935};
t2284 = ct{936};
t2285 = ct{937};
t2286 = ct{938};
t2287 = ct{939};
t2291 = ct{940};
t2292 = ct{941};
t2294 = ct{942};
t2295 = ct{943};
t23 = ct{944};
t230 = ct{945};
t2302 = ct{946};
t2304 = ct{947};
t2305 = ct{948};
t2306 = ct{949};
t2307 = ct{950};
t2308 = ct{951};
t2309 = ct{952};
t231 = ct{953};
t2310 = ct{954};
t2311 = ct{955};
t2312 = ct{956};
t2314 = ct{957};
t2316 = ct{958};
t2317 = ct{959};
t2318 = ct{960};
t2321 = ct{961};
t2322 = ct{962};
t2323 = ct{963};
t2324 = ct{964};
t233 = ct{965};
t2331 = ct{966};
t2333 = ct{967};
t2334 = ct{968};
t2335 = ct{969};
t2336 = ct{970};
t2337 = ct{971};
t2338 = ct{972};
t2339 = ct{973};
t234 = ct{974};
t2340 = ct{975};
t2341 = ct{976};
t2342 = ct{977};
t2344 = ct{978};
t2347 = ct{979};
t2348 = ct{980};
t235 = ct{981};
t2350 = ct{982};
t2351 = ct{983};
t2355 = ct{984};
t2357 = ct{985};
t2358 = ct{986};
t2359 = ct{987};
t236 = ct{988};
t2361 = ct{989};
t2362 = ct{990};
t2363 = ct{991};
t2364 = ct{992};
t2365 = ct{993};
t2366 = ct{994};
t2368 = ct{995};
t2369 = ct{996};
t2370 = ct{997};
t2371 = ct{998};
t2372 = ct{999};
t2373 = ct{1000};
t2374 = ct{1001};
t2375 = ct{1002};
t2376 = ct{1003};
t2377 = ct{1004};
t2378 = ct{1005};
t2379 = ct{1006};
t2381 = ct{1007};
t2382 = ct{1008};
t2384 = ct{1009};
t2385 = ct{1010};
t2387 = ct{1011};
t2388 = ct{1012};
t2389 = ct{1013};
t239 = ct{1014};
t2390 = ct{1015};
t2391 = ct{1016};
t2392 = ct{1017};
t2394 = ct{1018};
t2395 = ct{1019};
t2396 = ct{1020};
t2397 = ct{1021};
t24 = ct{1022};
t240 = ct{1023};
t2400 = ct{1024};
t2401 = ct{1025};
t2402 = ct{1026};
t2403 = ct{1027};
t2405 = ct{1028};
t2406 = ct{1029};
t2407 = ct{1030};
t2410 = ct{1031};
t2417 = ct{1032};
t2421 = ct{1033};
t2422 = ct{1034};
t2423 = ct{1035};
t2425 = ct{1036};
t2427 = ct{1037};
t2428 = ct{1038};
t2429 = ct{1039};
t243 = ct{1040};
t2430 = ct{1041};
t2431 = ct{1042};
t2434 = ct{1043};
t2435 = ct{1044};
t2437 = ct{1045};
t2438 = ct{1046};
t2439 = ct{1047};
t244 = ct{1048};
t2440 = ct{1049};
t2441 = ct{1050};
t2442 = ct{1051};
t2443 = ct{1052};
t2444 = ct{1053};
t2445 = ct{1054};
t2446 = ct{1055};
t2449 = ct{1056};
t2450 = ct{1057};
t2452 = ct{1058};
t2453 = ct{1059};
t2454 = ct{1060};
t2455 = ct{1061};
t2456 = ct{1062};
t2457 = ct{1063};
t2458 = ct{1064};
t2459 = ct{1065};
t2460 = ct{1066};
t2461 = ct{1067};
t2463 = ct{1068};
t2464 = ct{1069};
t2466 = ct{1070};
t2467 = ct{1071};
t2469 = ct{1072};
t2470 = ct{1073};
t2471 = ct{1074};
t2472 = ct{1075};
t2474 = ct{1076};
t2477 = ct{1077};
t2478 = ct{1078};
t2480 = ct{1079};
t2481 = ct{1080};
t2482 = ct{1081};
t2483 = ct{1082};
t2484 = ct{1083};
t2485 = ct{1084};
t2486 = ct{1085};
t2487 = ct{1086};
t2489 = ct{1087};
t249 = ct{1088};
t2495 = ct{1089};
t2497 = ct{1090};
t25 = ct{1091};
t2500 = ct{1092};
t2502 = ct{1093};
t2503 = ct{1094};
t2505 = ct{1095};
t2506 = ct{1096};
t2507 = ct{1097};
t2508 = ct{1098};
t2509 = ct{1099};
t2510 = ct{1100};
t2511 = ct{1101};
t2512 = ct{1102};
t2513 = ct{1103};
t2517 = ct{1104};
t2518 = ct{1105};
t2519 = ct{1106};
t2520 = ct{1107};
t2521 = ct{1108};
t2522 = ct{1109};
t2523 = ct{1110};
t2524 = ct{1111};
t2525 = ct{1112};
t2526 = ct{1113};
t2527 = ct{1114};
t2530 = ct{1115};
t2531 = ct{1116};
t2532 = ct{1117};
t2533 = ct{1118};
t2535 = ct{1119};
t2536 = ct{1120};
t2537 = ct{1121};
t2539 = ct{1122};
t2540 = ct{1123};
t2541 = ct{1124};
t2543 = ct{1125};
t2544 = ct{1126};
t2545 = ct{1127};
t2546 = ct{1128};
t2548 = ct{1129};
t2549 = ct{1130};
t2550 = ct{1131};
t2552 = ct{1132};
t2553 = ct{1133};
t2554 = ct{1134};
t2555 = ct{1135};
t2556 = ct{1136};
t2560 = ct{1137};
t2562 = ct{1138};
t2563 = ct{1139};
t2564 = ct{1140};
t2565 = ct{1141};
t2566 = ct{1142};
t2567 = ct{1143};
t2568 = ct{1144};
t2569 = ct{1145};
t257 = ct{1146};
t2570 = ct{1147};
t2571 = ct{1148};
t2574 = ct{1149};
t2575 = ct{1150};
t2576 = ct{1151};
t2577 = ct{1152};
t2578 = ct{1153};
t2579 = ct{1154};
t258 = ct{1155};
t2580 = ct{1156};
t2581 = ct{1157};
t2582 = ct{1158};
t2585 = ct{1159};
t2586 = ct{1160};
t2587 = ct{1161};
t2588 = ct{1162};
t2589 = ct{1163};
t2590 = ct{1164};
t2595 = ct{1165};
t2597 = ct{1166};
t2598 = ct{1167};
t2599 = ct{1168};
t26 = ct{1169};
t2600 = ct{1170};
t2601 = ct{1171};
t2602 = ct{1172};
t2603 = ct{1173};
t2604 = ct{1174};
t2606 = ct{1175};
t2607 = ct{1176};
t2608 = ct{1177};
t2611 = ct{1178};
t2612 = ct{1179};
t2615 = ct{1180};
t2616 = ct{1181};
t2617 = ct{1182};
t2627 = ct{1183};
t263 = ct{1184};
t2633 = ct{1185};
t2634 = ct{1186};
t2636 = ct{1187};
t2639 = ct{1188};
t2640 = ct{1189};
t2641 = ct{1190};
t2654 = ct{1191};
t2655 = ct{1192};
t2656 = ct{1193};
t2659 = ct{1194};
t266 = ct{1195};
t2666 = ct{1196};
t2668 = ct{1197};
t2669 = ct{1198};
t2671 = ct{1199};
t2673 = ct{1200};
t2675 = ct{1201};
t2676 = ct{1202};
t2677 = ct{1203};
t2678 = ct{1204};
t2680 = ct{1205};
t2681 = ct{1206};
t2682 = ct{1207};
t2684 = ct{1208};
t2685 = ct{1209};
t2686 = ct{1210};
t2688 = ct{1211};
t2692 = ct{1212};
t2693 = ct{1213};
t2694 = ct{1214};
t2695 = ct{1215};
t2699 = ct{1216};
t270 = ct{1217};
t2702 = ct{1218};
t2703 = ct{1219};
t2705 = ct{1220};
t2706 = ct{1221};
t2707 = ct{1222};
t2708 = ct{1223};
t2719 = ct{1224};
t2720 = ct{1225};
t2721 = ct{1226};
t2722 = ct{1227};
t2723 = ct{1228};
t2724 = ct{1229};
t2725 = ct{1230};
t2726 = ct{1231};
t273 = ct{1232};
t2733 = ct{1233};
t2734 = ct{1234};
t2739 = ct{1235};
t274 = ct{1236};
t2741 = ct{1237};
t2742 = ct{1238};
t2743 = ct{1239};
t2744 = ct{1240};
t2748 = ct{1241};
t2749 = ct{1242};
t275 = ct{1243};
t2752 = ct{1244};
t2759 = ct{1245};
t276 = ct{1246};
t2760 = ct{1247};
t2761 = ct{1248};
t2762 = ct{1249};
t2764 = ct{1250};
t2768 = ct{1251};
t2769 = ct{1252};
t277 = ct{1253};
t2770 = ct{1254};
t2771 = ct{1255};
t2773 = ct{1256};
t2774 = ct{1257};
t2775 = ct{1258};
t2776 = ct{1259};
t278 = ct{1260};
t2781 = ct{1261};
t2782 = ct{1262};
t2783 = ct{1263};
t2784 = ct{1264};
t2786 = ct{1265};
t2787 = ct{1266};
t2788 = ct{1267};
t2789 = ct{1268};
t2791 = ct{1269};
t2792 = ct{1270};
t280 = ct{1271};
t2806 = ct{1272};
t2808 = ct{1273};
t2815 = ct{1274};
t2820 = ct{1275};
t2821 = ct{1276};
t2829 = ct{1277};
t2830 = ct{1278};
t2831 = ct{1279};
t284 = ct{1280};
t2840 = ct{1281};
t2842 = ct{1282};
t2844 = ct{1283};
t2845 = ct{1284};
t2847 = ct{1285};
t2848 = ct{1286};
t2849 = ct{1287};
t2853 = ct{1288};
t2854 = ct{1289};
t2861 = ct{1290};
t2862 = ct{1291};
t2863 = ct{1292};
t2864 = ct{1293};
t2866 = ct{1294};
t2868 = ct{1295};
t2869 = ct{1296};
t287 = ct{1297};
t2879 = ct{1298};
t2884 = ct{1299};
t2886 = ct{1300};
t2888 = ct{1301};
t2892 = ct{1302};
t2898 = ct{1303};
t2899 = ct{1304};
t29 = ct{1305};
t290 = ct{1306};
t2900 = ct{1307};
t2901 = ct{1308};
t2902 = ct{1309};
t2903 = ct{1310};
t2908 = ct{1311};
t291 = ct{1312};
t292 = ct{1313};
t2920 = ct{1314};
t2923 = ct{1315};
t2925 = ct{1316};
t2926 = ct{1317};
t2928 = ct{1318};
t2929 = ct{1319};
t2930 = ct{1320};
t2937 = ct{1321};
t294 = ct{1322};
t2940 = ct{1323};
t2943 = ct{1324};
t2945 = ct{1325};
t2948 = ct{1326};
t2949 = ct{1327};
t2950 = ct{1328};
t2951 = ct{1329};
t2952 = ct{1330};
t2960 = ct{1331};
t2961 = ct{1332};
t2962 = ct{1333};
t2963 = ct{1334};
t2964 = ct{1335};
t2966 = ct{1336};
t2967 = ct{1337};
t2968 = ct{1338};
t2969 = ct{1339};
t297 = ct{1340};
t2970 = ct{1341};
t2971 = ct{1342};
t2975 = ct{1343};
t2976 = ct{1344};
t2980 = ct{1345};
t2982 = ct{1346};
t2983 = ct{1347};
t2984 = ct{1348};
t2985 = ct{1349};
t2986 = ct{1350};
t2988 = ct{1351};
t2989 = ct{1352};
t299 = ct{1353};
t2991 = ct{1354};
t2992 = ct{1355};
t2993 = ct{1356};
t2996 = ct{1357};
t2997 = ct{1358};
t3 = ct{1359};
t30 = ct{1360};
t300 = ct{1361};
t3003 = ct{1362};
t3004 = ct{1363};
t3007 = ct{1364};
t3010 = ct{1365};
t3011 = ct{1366};
t3013 = ct{1367};
t3014 = ct{1368};
t3019 = ct{1369};
t302 = ct{1370};
t3020 = ct{1371};
t3021 = ct{1372};
t3023 = ct{1373};
t3024 = ct{1374};
t3025 = ct{1375};
t3027 = ct{1376};
t3028 = ct{1377};
t3029 = ct{1378};
t303 = ct{1379};
t3030 = ct{1380};
t3031 = ct{1381};
t3032 = ct{1382};
t3033 = ct{1383};
t3034 = ct{1384};
t3035 = ct{1385};
t3036 = ct{1386};
t3038 = ct{1387};
t3039 = ct{1388};
t304 = ct{1389};
t3043 = ct{1390};
t3045 = ct{1391};
t3046 = ct{1392};
t3047 = ct{1393};
t305 = ct{1394};
t3051 = ct{1395};
t3052 = ct{1396};
t3053 = ct{1397};
t3055 = ct{1398};
t3056 = ct{1399};
t3057 = ct{1400};
t306 = ct{1401};
t3060 = ct{1402};
t3061 = ct{1403};
t3062 = ct{1404};
t3063 = ct{1405};
t3065 = ct{1406};
t3066 = ct{1407};
t3069 = ct{1408};
t3070 = ct{1409};
t3071 = ct{1410};
t3072 = ct{1411};
t3073 = ct{1412};
t3075 = ct{1413};
t3077 = ct{1414};
t3078 = ct{1415};
t3079 = ct{1416};
t3080 = ct{1417};
t3082 = ct{1418};
t3083 = ct{1419};
t3085 = ct{1420};
t3087 = ct{1421};
t309 = ct{1422};
t3090 = ct{1423};
t3091 = ct{1424};
t3092 = ct{1425};
t3093 = ct{1426};
t3094 = ct{1427};
t3095 = ct{1428};
t3098 = ct{1429};
t3099 = ct{1430};
t310 = ct{1431};
t3103 = ct{1432};
t3104 = ct{1433};
t3105 = ct{1434};
t3108 = ct{1435};
t3109 = ct{1436};
t311 = ct{1437};
t3112 = ct{1438};
t3113 = ct{1439};
t3119 = ct{1440};
t3120 = ct{1441};
t3123 = ct{1442};
t3124 = ct{1443};
t3126 = ct{1444};
t3127 = ct{1445};
t313 = ct{1446};
t3130 = ct{1447};
t3131 = ct{1448};
t3132 = ct{1449};
t3133 = ct{1450};
t3139 = ct{1451};
t314 = ct{1452};
t3140 = ct{1453};
t3142 = ct{1454};
t3143 = ct{1455};
t3145 = ct{1456};
t3146 = ct{1457};
t3148 = ct{1458};
t3149 = ct{1459};
t315 = ct{1460};
t3150 = ct{1461};
t3151 = ct{1462};
t3152 = ct{1463};
t3156 = ct{1464};
t3157 = ct{1465};
t3158 = ct{1466};
t316 = ct{1467};
t3160 = ct{1468};
t3163 = ct{1469};
t3165 = ct{1470};
t3167 = ct{1471};
t3170 = ct{1472};
t3171 = ct{1473};
t3172 = ct{1474};
t3173 = ct{1475};
t3174 = ct{1476};
t3177 = ct{1477};
t3178 = ct{1478};
t318 = ct{1479};
t3180 = ct{1480};
t3182 = ct{1481};
t3183 = ct{1482};
t3184 = ct{1483};
t3186 = ct{1484};
t3187 = ct{1485};
t319 = ct{1486};
t3190 = ct{1487};
t3191 = ct{1488};
t3194 = ct{1489};
t3197 = ct{1490};
t3199 = ct{1491};
t320 = ct{1492};
t3206 = ct{1493};
t3207 = ct{1494};
t3208 = ct{1495};
t3218 = ct{1496};
t3219 = ct{1497};
t322 = ct{1498};
t3228 = ct{1499};
t3230 = ct{1500};
t3231 = ct{1501};
t3234 = ct{1502};
t3236 = ct{1503};
t324 = ct{1504};
t3240 = ct{1505};
t3241 = ct{1506};
t3242 = ct{1507};
t3243 = ct{1508};
t3244 = ct{1509};
t3245 = ct{1510};
t325 = ct{1511};
t3250 = ct{1512};
t3251 = ct{1513};
t3252 = ct{1514};
t3253 = ct{1515};
t3254 = ct{1516};
t3256 = ct{1517};
t3257 = ct{1518};
t3260 = ct{1519};
t3265 = ct{1520};
t3272 = ct{1521};
t3273 = ct{1522};
t3274 = ct{1523};
t3275 = ct{1524};
t3276 = ct{1525};
t3277 = ct{1526};
t3278 = ct{1527};
t3279 = ct{1528};
t328 = ct{1529};
t3280 = ct{1530};
t3282 = ct{1531};
t3283 = ct{1532};
t3284 = ct{1533};
t3285 = ct{1534};
t3286 = ct{1535};
t3287 = ct{1536};
t3288 = ct{1537};
t3289 = ct{1538};
t3290 = ct{1539};
t3291 = ct{1540};
t3292 = ct{1541};
t3293 = ct{1542};
t3295 = ct{1543};
t3296 = ct{1544};
t3297 = ct{1545};
t3298 = ct{1546};
t3299 = ct{1547};
t3301 = ct{1548};
t3302 = ct{1549};
t3303 = ct{1550};
t3304 = ct{1551};
t3306 = ct{1552};
t3307 = ct{1553};
t3308 = ct{1554};
t3309 = ct{1555};
t3310 = ct{1556};
t3312 = ct{1557};
t3313 = ct{1558};
t3314 = ct{1559};
t3315 = ct{1560};
t3317 = ct{1561};
t3318 = ct{1562};
t3320 = ct{1563};
t3321 = ct{1564};
t3324 = ct{1565};
t3325 = ct{1566};
t3326 = ct{1567};
t3327 = ct{1568};
t3328 = ct{1569};
t3329 = ct{1570};
t333 = ct{1571};
t3331 = ct{1572};
t3333 = ct{1573};
t3334 = ct{1574};
t3335 = ct{1575};
t3338 = ct{1576};
t3339 = ct{1577};
t3342 = ct{1578};
t3343 = ct{1579};
t3346 = ct{1580};
t3347 = ct{1581};
t3350 = ct{1582};
t336 = ct{1583};
t3362 = ct{1584};
t3363 = ct{1585};
t3364 = ct{1586};
t3365 = ct{1587};
t3366 = ct{1588};
t3367 = ct{1589};
t3368 = ct{1590};
t3369 = ct{1591};
t337 = ct{1592};
t3371 = ct{1593};
t3372 = ct{1594};
t3373 = ct{1595};
t3374 = ct{1596};
t3375 = ct{1597};
t3376 = ct{1598};
t3377 = ct{1599};
t3378 = ct{1600};
t3380 = ct{1601};
t3381 = ct{1602};
t3382 = ct{1603};
t3383 = ct{1604};
t3384 = ct{1605};
t3387 = ct{1606};
t3390 = ct{1607};
t3391 = ct{1608};
t3392 = ct{1609};
t3393 = ct{1610};
t3394 = ct{1611};
t3395 = ct{1612};
t3396 = ct{1613};
t3397 = ct{1614};
t3398 = ct{1615};
t3399 = ct{1616};
t34 = ct{1617};
t340 = ct{1618};
t3400 = ct{1619};
t3402 = ct{1620};
t3403 = ct{1621};
t3404 = ct{1622};
t3405 = ct{1623};
t3406 = ct{1624};
t3407 = ct{1625};
t3408 = ct{1626};
t3409 = ct{1627};
t3410 = ct{1628};
t3411 = ct{1629};
t3412 = ct{1630};
t3413 = ct{1631};
t3416 = ct{1632};
t3417 = ct{1633};
t3418 = ct{1634};
t3420 = ct{1635};
t3421 = ct{1636};
t3422 = ct{1637};
t3423 = ct{1638};
t3424 = ct{1639};
t3425 = ct{1640};
t3426 = ct{1641};
t3427 = ct{1642};
t3430 = ct{1643};
t3431 = ct{1644};
t3432 = ct{1645};
t3433 = ct{1646};
t3434 = ct{1647};
t3435 = ct{1648};
t3436 = ct{1649};
t3437 = ct{1650};
t3439 = ct{1651};
t344 = ct{1652};
t3440 = ct{1653};
t3441 = ct{1654};
t3442 = ct{1655};
t3443 = ct{1656};
t3444 = ct{1657};
t3445 = ct{1658};
t3446 = ct{1659};
t3447 = ct{1660};
t3449 = ct{1661};
t3450 = ct{1662};
t3453 = ct{1663};
t3454 = ct{1664};
t3455 = ct{1665};
t3456 = ct{1666};
t3457 = ct{1667};
t3458 = ct{1668};
t346 = ct{1669};
t3462 = ct{1670};
t3463 = ct{1671};
t3464 = ct{1672};
t3465 = ct{1673};
t3466 = ct{1674};
t3467 = ct{1675};
t3468 = ct{1676};
t3469 = ct{1677};
t347 = ct{1678};
t3470 = ct{1679};
t3471 = ct{1680};
t3472 = ct{1681};
t3473 = ct{1682};
t3474 = ct{1683};
t3475 = ct{1684};
t3476 = ct{1685};
t3479 = ct{1686};
t348 = ct{1687};
t3480 = ct{1688};
t3481 = ct{1689};
t3483 = ct{1690};
t3485 = ct{1691};
t3487 = ct{1692};
t3488 = ct{1693};
t3489 = ct{1694};
t349 = ct{1695};
t3490 = ct{1696};
t3491 = ct{1697};
t3492 = ct{1698};
t3493 = ct{1699};
t3494 = ct{1700};
t3496 = ct{1701};
t3497 = ct{1702};
t3498 = ct{1703};
t3499 = ct{1704};
t350 = ct{1705};
t3500 = ct{1706};
t3501 = ct{1707};
t3502 = ct{1708};
t3503 = ct{1709};
t3504 = ct{1710};
t3505 = ct{1711};
t3506 = ct{1712};
t3507 = ct{1713};
t3509 = ct{1714};
t3510 = ct{1715};
t3511 = ct{1716};
t3513 = ct{1717};
t3514 = ct{1718};
t3515 = ct{1719};
t3516 = ct{1720};
t3517 = ct{1721};
t3518 = ct{1722};
t352 = ct{1723};
t3521 = ct{1724};
t3522 = ct{1725};
t3523 = ct{1726};
t3527 = ct{1727};
t3528 = ct{1728};
t3529 = ct{1729};
t353 = ct{1730};
t3530 = ct{1731};
t3531 = ct{1732};
t3532 = ct{1733};
t3533 = ct{1734};
t3535 = ct{1735};
t3536 = ct{1736};
t3538 = ct{1737};
t3539 = ct{1738};
t3542 = ct{1739};
t3543 = ct{1740};
t3544 = ct{1741};
t3545 = ct{1742};
t3546 = ct{1743};
t3547 = ct{1744};
t3549 = ct{1745};
t3550 = ct{1746};
t3551 = ct{1747};
t3552 = ct{1748};
t3554 = ct{1749};
t3556 = ct{1750};
t3557 = ct{1751};
t3559 = ct{1752};
t356 = ct{1753};
t3560 = ct{1754};
t3562 = ct{1755};
t3563 = ct{1756};
t3564 = ct{1757};
t3567 = ct{1758};
t3568 = ct{1759};
t3569 = ct{1760};
t357 = ct{1761};
t3571 = ct{1762};
t3572 = ct{1763};
t3573 = ct{1764};
t3574 = ct{1765};
t3577 = ct{1766};
t3578 = ct{1767};
t358 = ct{1768};
t3582 = ct{1769};
t3583 = ct{1770};
t3584 = ct{1771};
t3585 = ct{1772};
t3586 = ct{1773};
t3587 = ct{1774};
t3589 = ct{1775};
t359 = ct{1776};
t3590 = ct{1777};
t3592 = ct{1778};
t3593 = ct{1779};
t3596 = ct{1780};
t3597 = ct{1781};
t3599 = ct{1782};
t3602 = ct{1783};
t3603 = ct{1784};
t3604 = ct{1785};
t3605 = ct{1786};
t3606 = ct{1787};
t3607 = ct{1788};
t3608 = ct{1789};
t3609 = ct{1790};
t361 = ct{1791};
t3610 = ct{1792};
t3611 = ct{1793};
t3612 = ct{1794};
t3614 = ct{1795};
t3615 = ct{1796};
t3616 = ct{1797};
t3617 = ct{1798};
t3618 = ct{1799};
t3619 = ct{1800};
t362 = ct{1801};
t3620 = ct{1802};
t3625 = ct{1803};
t3630 = ct{1804};
t3631 = ct{1805};
t3633 = ct{1806};
t3634 = ct{1807};
t3635 = ct{1808};
t3636 = ct{1809};
t3637 = ct{1810};
t3638 = ct{1811};
t3642 = ct{1812};
t3644 = ct{1813};
t3648 = ct{1814};
t365 = ct{1815};
t3652 = ct{1816};
t3653 = ct{1817};
t3654 = ct{1818};
t3655 = ct{1819};
t3656 = ct{1820};
t3657 = ct{1821};
t3658 = ct{1822};
t3659 = ct{1823};
t3660 = ct{1824};
t3662 = ct{1825};
t3663 = ct{1826};
t3666 = ct{1827};
t3667 = ct{1828};
t3668 = ct{1829};
t3676 = ct{1830};
t368 = ct{1831};
t3681 = ct{1832};
t3682 = ct{1833};
t3687 = ct{1834};
t3688 = ct{1835};
t369 = ct{1836};
t3690 = ct{1837};
t3691 = ct{1838};
t3693 = ct{1839};
t3694 = ct{1840};
t3695 = ct{1841};
t3696 = ct{1842};
t3697 = ct{1843};
t3699 = ct{1844};
t3700 = ct{1845};
t3701 = ct{1846};
t3702 = ct{1847};
t3704 = ct{1848};
t3705 = ct{1849};
t3706 = ct{1850};
t3707 = ct{1851};
t3708 = ct{1852};
t3709 = ct{1853};
t371 = ct{1854};
t3713 = ct{1855};
t3715 = ct{1856};
t3716 = ct{1857};
t3717 = ct{1858};
t372 = ct{1859};
t3720 = ct{1860};
t3721 = ct{1861};
t3723 = ct{1862};
t3724 = ct{1863};
t3725 = ct{1864};
t3726 = ct{1865};
t3728 = ct{1866};
t3729 = ct{1867};
t373 = ct{1868};
t3730 = ct{1869};
t3732 = ct{1870};
t3733 = ct{1871};
t3734 = ct{1872};
t3735 = ct{1873};
t3736 = ct{1874};
t3737 = ct{1875};
t3738 = ct{1876};
t374 = ct{1877};
t3743 = ct{1878};
t3744 = ct{1879};
t3745 = ct{1880};
t3746 = ct{1881};
t3747 = ct{1882};
t3750 = ct{1883};
t3752 = ct{1884};
t3756 = ct{1885};
t3757 = ct{1886};
t3758 = ct{1887};
t3766 = ct{1888};
t3768 = ct{1889};
t3769 = ct{1890};
t377 = ct{1891};
t3774 = ct{1892};
t3776 = ct{1893};
t3778 = ct{1894};
t378 = ct{1895};
t3780 = ct{1896};
t3783 = ct{1897};
t3784 = ct{1898};
t3785 = ct{1899};
t3786 = ct{1900};
t3787 = ct{1901};
t3789 = ct{1902};
t379 = ct{1903};
t3792 = ct{1904};
t3795 = ct{1905};
t3798 = ct{1906};
t380 = ct{1907};
t3800 = ct{1908};
t3803 = ct{1909};
t3804 = ct{1910};
t3805 = ct{1911};
t3806 = ct{1912};
t3810 = ct{1913};
t3811 = ct{1914};
t3813 = ct{1915};
t3814 = ct{1916};
t3815 = ct{1917};
t3816 = ct{1918};
t3817 = ct{1919};
t3819 = ct{1920};
t382 = ct{1921};
t3820 = ct{1922};
t3821 = ct{1923};
t3822 = ct{1924};
t3823 = ct{1925};
t3824 = ct{1926};
t3825 = ct{1927};
t3826 = ct{1928};
t3827 = ct{1929};
t3831 = ct{1930};
t3834 = ct{1931};
t3835 = ct{1932};
t3839 = ct{1933};
t384 = ct{1934};
t3843 = ct{1935};
t3849 = ct{1936};
t3850 = ct{1937};
t3851 = ct{1938};
t3852 = ct{1939};
t3853 = ct{1940};
t3855 = ct{1941};
t3857 = ct{1942};
t3858 = ct{1943};
t386 = ct{1944};
t3866 = ct{1945};
t3867 = ct{1946};
t3869 = ct{1947};
t387 = ct{1948};
t3870 = ct{1949};
t3877 = ct{1950};
t388 = ct{1951};
t3885 = ct{1952};
t3889 = ct{1953};
t3890 = ct{1954};
t3891 = ct{1955};
t3892 = ct{1956};
t3899 = ct{1957};
t391 = ct{1958};
t3912 = ct{1959};
t3913 = ct{1960};
t3915 = ct{1961};
t3917 = ct{1962};
t392 = ct{1963};
t3929 = ct{1964};
t3930 = ct{1965};
t3941 = ct{1966};
t3946 = ct{1967};
t3949 = ct{1968};
t395 = ct{1969};
t3950 = ct{1970};
t3951 = ct{1971};
t3952 = ct{1972};
t3953 = ct{1973};
t3958 = ct{1974};
t3959 = ct{1975};
t396 = ct{1976};
t3966 = ct{1977};
t3970 = ct{1978};
t3980 = ct{1979};
t3981 = ct{1980};
t3982 = ct{1981};
t3984 = ct{1982};
t3990 = ct{1983};
t4 = ct{1984};
t400 = ct{1985};
t4004 = ct{1986};
t4005 = ct{1987};
t4006 = ct{1988};
t401 = ct{1989};
t4010 = ct{1990};
t4011 = ct{1991};
t4014 = ct{1992};
t4015 = ct{1993};
t4016 = ct{1994};
t4017 = ct{1995};
t4018 = ct{1996};
t4019 = ct{1997};
t402 = ct{1998};
t4020 = ct{1999};
t4021 = ct{2000};
t4022 = ct{2001};
t4023 = ct{2002};
t4024 = ct{2003};
t4025 = ct{2004};
t4026 = ct{2005};
t4027 = ct{2006};
t4028 = ct{2007};
t4029 = ct{2008};
t403 = ct{2009};
t4036 = ct{2010};
t4039 = ct{2011};
t4040 = ct{2012};
t4041 = ct{2013};
t4042 = ct{2014};
t4045 = ct{2015};
t4046 = ct{2016};
t4047 = ct{2017};
t4048 = ct{2018};
t4051 = ct{2019};
t4053 = ct{2020};
t4054 = ct{2021};
t406 = ct{2022};
t4062 = ct{2023};
t4063 = ct{2024};
t4064 = ct{2025};
t4065 = ct{2026};
t4068 = ct{2027};
t4069 = ct{2028};
t4070 = ct{2029};
t4071 = ct{2030};
t4073 = ct{2031};
t4074 = ct{2032};
t4075 = ct{2033};
t4089 = ct{2034};
t4099 = ct{2035};
t410 = ct{2036};
t4103 = ct{2037};
t4105 = ct{2038};
t411 = ct{2039};
t4113 = ct{2040};
t4114 = ct{2041};
t4116 = ct{2042};
t4118 = ct{2043};
t4119 = ct{2044};
t412 = ct{2045};
t4123 = ct{2046};
t4124 = ct{2047};
t4125 = ct{2048};
t413 = ct{2049};
t4132 = ct{2050};
t414 = ct{2051};
t4140 = ct{2052};
t4142 = ct{2053};
t4143 = ct{2054};
t4144 = ct{2055};
t4145 = ct{2056};
t415 = ct{2057};
t4150 = ct{2058};
t4152 = ct{2059};
t4153 = ct{2060};
t416 = ct{2061};
t4162 = ct{2062};
t4164 = ct{2063};
t4165 = ct{2064};
t4166 = ct{2065};
t4169 = ct{2066};
t417 = ct{2067};
t4171 = ct{2068};
t4173 = ct{2069};
t4174 = ct{2070};
t4177 = ct{2071};
t4178 = ct{2072};
t4179 = ct{2073};
t418 = ct{2074};
t4180 = ct{2075};
t4181 = ct{2076};
t4183 = ct{2077};
t4184 = ct{2078};
t4185 = ct{2079};
t4186 = ct{2080};
t4188 = ct{2081};
t4190 = ct{2082};
t4195 = ct{2083};
t4196 = ct{2084};
t4197 = ct{2085};
t420 = ct{2086};
t4201 = ct{2087};
t4202 = ct{2088};
t4205 = ct{2089};
t4206 = ct{2090};
t4207 = ct{2091};
t4208 = ct{2092};
t4209 = ct{2093};
t4210 = ct{2094};
t4211 = ct{2095};
t4215 = ct{2096};
t4217 = ct{2097};
t4218 = ct{2098};
t4219 = ct{2099};
t422 = ct{2100};
t4220 = ct{2101};
t4221 = ct{2102};
t4223 = ct{2103};
t4224 = ct{2104};
t4225 = ct{2105};
t4226 = ct{2106};
t4228 = ct{2107};
t4229 = ct{2108};
t423 = ct{2109};
t4230 = ct{2110};
t4231 = ct{2111};
t4232 = ct{2112};
t4233 = ct{2113};
t4234 = ct{2114};
t4235 = ct{2115};
t424 = ct{2116};
t4241 = ct{2117};
t4242 = ct{2118};
t4243 = ct{2119};
t4244 = ct{2120};
t4245 = ct{2121};
t4246 = ct{2122};
t4247 = ct{2123};
t4248 = ct{2124};
t4249 = ct{2125};
t425 = ct{2126};
t4250 = ct{2127};
t4251 = ct{2128};
t4253 = ct{2129};
t4254 = ct{2130};
t4255 = ct{2131};
t4256 = ct{2132};
t4257 = ct{2133};
t4258 = ct{2134};
t4259 = ct{2135};
t4260 = ct{2136};
t4261 = ct{2137};
t4262 = ct{2138};
t4263 = ct{2139};
t427 = ct{2140};
t4273 = ct{2141};
t4274 = ct{2142};
t4275 = ct{2143};
t4276 = ct{2144};
t4278 = ct{2145};
t4279 = ct{2146};
t428 = ct{2147};
t4280 = ct{2148};
t4281 = ct{2149};
t4282 = ct{2150};
t4283 = ct{2151};
t4284 = ct{2152};
t4285 = ct{2153};
t4286 = ct{2154};
t4287 = ct{2155};
t4289 = ct{2156};
t429 = ct{2157};
t4290 = ct{2158};
t4291 = ct{2159};
t4292 = ct{2160};
t4293 = ct{2161};
t4295 = ct{2162};
t4296 = ct{2163};
t4297 = ct{2164};
t4298 = ct{2165};
t4299 = ct{2166};
t4300 = ct{2167};
t4301 = ct{2168};
t4302 = ct{2169};
t4303 = ct{2170};
t4304 = ct{2171};
t4305 = ct{2172};
t4306 = ct{2173};
t4308 = ct{2174};
t431 = ct{2175};
t4310 = ct{2176};
t4315 = ct{2177};
t4316 = ct{2178};
t4317 = ct{2179};
t4318 = ct{2180};
t432 = ct{2181};
t4321 = ct{2182};
t4323 = ct{2183};
t4324 = ct{2184};
t4325 = ct{2185};
t4326 = ct{2186};
t4327 = ct{2187};
t4328 = ct{2188};
t4329 = ct{2189};
t433 = ct{2190};
t4330 = ct{2191};
t4331 = ct{2192};
t4332 = ct{2193};
t4333 = ct{2194};
t4334 = ct{2195};
t4335 = ct{2196};
t4336 = ct{2197};
t4337 = ct{2198};
t4338 = ct{2199};
t4339 = ct{2200};
t434 = ct{2201};
t4340 = ct{2202};
t4342 = ct{2203};
t4344 = ct{2204};
t4345 = ct{2205};
t4346 = ct{2206};
t4347 = ct{2207};
t4348 = ct{2208};
t4349 = ct{2209};
t435 = ct{2210};
t4350 = ct{2211};
t4354 = ct{2212};
t4356 = ct{2213};
t4357 = ct{2214};
t436 = ct{2215};
t4362 = ct{2216};
t4363 = ct{2217};
t4365 = ct{2218};
t4366 = ct{2219};
t4368 = ct{2220};
t4369 = ct{2221};
t437 = ct{2222};
t4370 = ct{2223};
t4371 = ct{2224};
t4372 = ct{2225};
t4373 = ct{2226};
t4374 = ct{2227};
t4375 = ct{2228};
t4376 = ct{2229};
t4377 = ct{2230};
t4379 = ct{2231};
t438 = ct{2232};
t4380 = ct{2233};
t4382 = ct{2234};
t4383 = ct{2235};
t4384 = ct{2236};
t4385 = ct{2237};
t4386 = ct{2238};
t4387 = ct{2239};
t4388 = ct{2240};
t4389 = ct{2241};
t439 = ct{2242};
t4391 = ct{2243};
t4392 = ct{2244};
t4394 = ct{2245};
t4395 = ct{2246};
t4396 = ct{2247};
t4397 = ct{2248};
t4398 = ct{2249};
t4399 = ct{2250};
t44 = ct{2251};
t440 = ct{2252};
t4400 = ct{2253};
t4401 = ct{2254};
t4402 = ct{2255};
t4403 = ct{2256};
t4404 = ct{2257};
t4405 = ct{2258};
t4406 = ct{2259};
t4407 = ct{2260};
t4408 = ct{2261};
t4409 = ct{2262};
t441 = ct{2263};
t4410 = ct{2264};
t4411 = ct{2265};
t4412 = ct{2266};
t4413 = ct{2267};
t4414 = ct{2268};
t4415 = ct{2269};
t4416 = ct{2270};
t4417 = ct{2271};
t4418 = ct{2272};
t4419 = ct{2273};
t442 = ct{2274};
t4420 = ct{2275};
t4421 = ct{2276};
t4422 = ct{2277};
t4423 = ct{2278};
t4424 = ct{2279};
t4425 = ct{2280};
t4426 = ct{2281};
t4427 = ct{2282};
t4428 = ct{2283};
t4429 = ct{2284};
t4430 = ct{2285};
t4431 = ct{2286};
t4432 = ct{2287};
t4433 = ct{2288};
t4434 = ct{2289};
t4435 = ct{2290};
t4436 = ct{2291};
t4437 = ct{2292};
t4438 = ct{2293};
t4439 = ct{2294};
t444 = ct{2295};
t4440 = ct{2296};
t4442 = ct{2297};
t4443 = ct{2298};
t4444 = ct{2299};
t4445 = ct{2300};
t4446 = ct{2301};
t4447 = ct{2302};
t4448 = ct{2303};
t4449 = ct{2304};
t445 = ct{2305};
t4450 = ct{2306};
t4451 = ct{2307};
t4452 = ct{2308};
t4453 = ct{2309};
t4454 = ct{2310};
t4455 = ct{2311};
t4457 = ct{2312};
t4459 = ct{2313};
t4460 = ct{2314};
t4461 = ct{2315};
t4462 = ct{2316};
t4463 = ct{2317};
t4464 = ct{2318};
t4465 = ct{2319};
t4466 = ct{2320};
t4467 = ct{2321};
t4468 = ct{2322};
t4469 = ct{2323};
t4470 = ct{2324};
t4471 = ct{2325};
t4473 = ct{2326};
t4474 = ct{2327};
t4475 = ct{2328};
t4476 = ct{2329};
t4477 = ct{2330};
t4478 = ct{2331};
t4479 = ct{2332};
t448 = ct{2333};
t4480 = ct{2334};
t4481 = ct{2335};
t4482 = ct{2336};
t4483 = ct{2337};
t4484 = ct{2338};
t4485 = ct{2339};
t4486 = ct{2340};
t4487 = ct{2341};
t4488 = ct{2342};
t4489 = ct{2343};
t449 = ct{2344};
t4490 = ct{2345};
t4491 = ct{2346};
t4492 = ct{2347};
t4493 = ct{2348};
t4495 = ct{2349};
t4498 = ct{2350};
t45 = ct{2351};
t450 = ct{2352};
t4501 = ct{2353};
t4502 = ct{2354};
t4504 = ct{2355};
t4506 = ct{2356};
t4508 = ct{2357};
t4509 = ct{2358};
t4513 = ct{2359};
t4516 = ct{2360};
t4517 = ct{2361};
t4519 = ct{2362};
t452 = ct{2363};
t4520 = ct{2364};
t4522 = ct{2365};
t4524 = ct{2366};
t4525 = ct{2367};
t453 = ct{2368};
t4530 = ct{2369};
t4532 = ct{2370};
t4533 = ct{2371};
t454 = ct{2372};
t4540 = ct{2373};
t4542 = ct{2374};
t4543 = ct{2375};
t4547 = ct{2376};
t4548 = ct{2377};
t4549 = ct{2378};
t4551 = ct{2379};
t4554 = ct{2380};
t4555 = ct{2381};
t4557 = ct{2382};
t4558 = ct{2383};
t4559 = ct{2384};
t4561 = ct{2385};
t4562 = ct{2386};
t4563 = ct{2387};
t4566 = ct{2388};
t4567 = ct{2389};
t4568 = ct{2390};
t4569 = ct{2391};
t457 = ct{2392};
t4570 = ct{2393};
t4571 = ct{2394};
t4572 = ct{2395};
t4574 = ct{2396};
t4575 = ct{2397};
t4577 = ct{2398};
t4579 = ct{2399};
t458 = ct{2400};
t4581 = ct{2401};
t4582 = ct{2402};
t4583 = ct{2403};
t4584 = ct{2404};
t4588 = ct{2405};
t4589 = ct{2406};
t459 = ct{2407};
t4590 = ct{2408};
t4591 = ct{2409};
t4595 = ct{2410};
t4596 = ct{2411};
t46 = ct{2412};
t460 = ct{2413};
t4600 = ct{2414};
t4601 = ct{2415};
t4605 = ct{2416};
t4606 = ct{2417};
t4607 = ct{2418};
t461 = ct{2419};
t4611 = ct{2420};
t4614 = ct{2421};
t4616 = ct{2422};
t4617 = ct{2423};
t462 = ct{2424};
t4621 = ct{2425};
t4622 = ct{2426};
t4625 = ct{2427};
t4626 = ct{2428};
t4628 = ct{2429};
t4629 = ct{2430};
t463 = ct{2431};
t4630 = ct{2432};
t4632 = ct{2433};
t4633 = ct{2434};
t4634 = ct{2435};
t4636 = ct{2436};
t4637 = ct{2437};
t4638 = ct{2438};
t4639 = ct{2439};
t464 = ct{2440};
t4640 = ct{2441};
t4641 = ct{2442};
t4642 = ct{2443};
t4643 = ct{2444};
t4644 = ct{2445};
t4645 = ct{2446};
t4646 = ct{2447};
t4647 = ct{2448};
t4649 = ct{2449};
t465 = ct{2450};
t4650 = ct{2451};
t4651 = ct{2452};
t4652 = ct{2453};
t4653 = ct{2454};
t4656 = ct{2455};
t4657 = ct{2456};
t4658 = ct{2457};
t466 = ct{2458};
t4660 = ct{2459};
t4661 = ct{2460};
t4662 = ct{2461};
t4663 = ct{2462};
t4666 = ct{2463};
t4667 = ct{2464};
t4669 = ct{2465};
t4672 = ct{2466};
t4673 = ct{2467};
t4674 = ct{2468};
t4675 = ct{2469};
t468 = ct{2470};
t4688 = ct{2471};
t469 = ct{2472};
t4691 = ct{2473};
t4692 = ct{2474};
t4693 = ct{2475};
t4694 = ct{2476};
t4695 = ct{2477};
t4696 = ct{2478};
t4697 = ct{2479};
t47 = ct{2480};
t470 = ct{2481};
t4707 = ct{2482};
t4708 = ct{2483};
t4709 = ct{2484};
t471 = ct{2485};
t4711 = ct{2486};
t4713 = ct{2487};
t4716 = ct{2488};
t472 = ct{2489};
t4722 = ct{2490};
t4723 = ct{2491};
t4724 = ct{2492};
t4725 = ct{2493};
t4726 = ct{2494};
t4727 = ct{2495};
t4728 = ct{2496};
t4731 = ct{2497};
t4732 = ct{2498};
t4733 = ct{2499};
t4734 = ct{2500};
t4737 = ct{2501};
t4740 = ct{2502};
t4741 = ct{2503};
t4742 = ct{2504};
t4745 = ct{2505};
t4747 = ct{2506};
t4748 = ct{2507};
t4749 = ct{2508};
t475 = ct{2509};
t4752 = ct{2510};
t4753 = ct{2511};
t4754 = ct{2512};
t4755 = ct{2513};
t4756 = ct{2514};
t4758 = ct{2515};
t4759 = ct{2516};
t4760 = ct{2517};
t4761 = ct{2518};
t4763 = ct{2519};
t4766 = ct{2520};
t4769 = ct{2521};
t477 = ct{2522};
t4770 = ct{2523};
t4777 = ct{2524};
t4778 = ct{2525};
t4782 = ct{2526};
t4783 = ct{2527};
t4785 = ct{2528};
t4786 = ct{2529};
t4788 = ct{2530};
t4789 = ct{2531};
t479 = ct{2532};
t4790 = ct{2533};
t4794 = ct{2534};
t4795 = ct{2535};
t4796 = ct{2536};
t4797 = ct{2537};
t4798 = ct{2538};
t4799 = ct{2539};
t480 = ct{2540};
t4800 = ct{2541};
t4801 = ct{2542};
t4803 = ct{2543};
t4804 = ct{2544};
t4805 = ct{2545};
t4807 = ct{2546};
t4808 = ct{2547};
t481 = ct{2548};
t4811 = ct{2549};
t4813 = ct{2550};
t4814 = ct{2551};
t4815 = ct{2552};
t4818 = ct{2553};
t482 = ct{2554};
t4820 = ct{2555};
t4824 = ct{2556};
t4825 = ct{2557};
t4827 = ct{2558};
t4828 = ct{2559};
t483 = ct{2560};
t4830 = ct{2561};
t4832 = ct{2562};
t4833 = ct{2563};
t4834 = ct{2564};
t4835 = ct{2565};
t4837 = ct{2566};
t4839 = ct{2567};
t484 = ct{2568};
t4841 = ct{2569};
t4842 = ct{2570};
t4845 = ct{2571};
t4846 = ct{2572};
t4849 = ct{2573};
t485 = ct{2574};
t4852 = ct{2575};
t486 = ct{2576};
t4861 = ct{2577};
t4862 = ct{2578};
t4864 = ct{2579};
t4865 = ct{2580};
t4866 = ct{2581};
t4867 = ct{2582};
t4871 = ct{2583};
t4872 = ct{2584};
t4873 = ct{2585};
t4876 = ct{2586};
t4877 = ct{2587};
t4878 = ct{2588};
t4879 = ct{2589};
t488 = ct{2590};
t4882 = ct{2591};
t4883 = ct{2592};
t4884 = ct{2593};
t4886 = ct{2594};
t4887 = ct{2595};
t489 = ct{2596};
t4895 = ct{2597};
t4897 = ct{2598};
t4899 = ct{2599};
t4900 = ct{2600};
t4908 = ct{2601};
t4909 = ct{2602};
t491 = ct{2603};
t4910 = ct{2604};
t4911 = ct{2605};
t4913 = ct{2606};
t4915 = ct{2607};
t4916 = ct{2608};
t4919 = ct{2609};
t492 = ct{2610};
t4920 = ct{2611};
t4923 = ct{2612};
t4924 = ct{2613};
t4925 = ct{2614};
t4927 = ct{2615};
t4928 = ct{2616};
t493 = ct{2617};
t4930 = ct{2618};
t4933 = ct{2619};
t4934 = ct{2620};
t4937 = ct{2621};
t4938 = ct{2622};
t494 = ct{2623};
t4941 = ct{2624};
t4942 = ct{2625};
t4943 = ct{2626};
t4944 = ct{2627};
t4945 = ct{2628};
t4946 = ct{2629};
t4948 = ct{2630};
t4951 = ct{2631};
t4955 = ct{2632};
t4956 = ct{2633};
t4957 = ct{2634};
t496 = ct{2635};
t4962 = ct{2636};
t4964 = ct{2637};
t4969 = ct{2638};
t497 = ct{2639};
t4970 = ct{2640};
t4973 = ct{2641};
t4974 = ct{2642};
t4976 = ct{2643};
t498 = ct{2644};
t4980 = ct{2645};
t4981 = ct{2646};
t4982 = ct{2647};
t4983 = ct{2648};
t4986 = ct{2649};
t4987 = ct{2650};
t4988 = ct{2651};
t499 = ct{2652};
t4991 = ct{2653};
t4993 = ct{2654};
t4996 = ct{2655};
t4998 = ct{2656};
t4999 = ct{2657};
t5 = ct{2658};
t50 = ct{2659};
t500 = ct{2660};
t5000 = ct{2661};
t5001 = ct{2662};
t5004 = ct{2663};
t5006 = ct{2664};
t5008 = ct{2665};
t501 = ct{2666};
t5019 = ct{2667};
t502 = ct{2668};
t5021 = ct{2669};
t5022 = ct{2670};
t5023 = ct{2671};
t5026 = ct{2672};
t5027 = ct{2673};
t5029 = ct{2674};
t503 = ct{2675};
t5034 = ct{2676};
t5035 = ct{2677};
t5036 = ct{2678};
t5038 = ct{2679};
t504 = ct{2680};
t5045 = ct{2681};
t5046 = ct{2682};
t505 = ct{2683};
t5051 = ct{2684};
t5052 = ct{2685};
t5053 = ct{2686};
t506 = ct{2687};
t5060 = ct{2688};
t5062 = ct{2689};
t5063 = ct{2690};
t5064 = ct{2691};
t5065 = ct{2692};
t5066 = ct{2693};
t5069 = ct{2694};
t507 = ct{2695};
t5071 = ct{2696};
t5072 = ct{2697};
t5073 = ct{2698};
t5078 = ct{2699};
t508 = ct{2700};
t5080 = ct{2701};
t5082 = ct{2702};
t5083 = ct{2703};
t5084 = ct{2704};
t5085 = ct{2705};
t509 = ct{2706};
t5091 = ct{2707};
t5093 = ct{2708};
t5095 = ct{2709};
t5096 = ct{2710};
t5097 = ct{2711};
t5098 = ct{2712};
t5099 = ct{2713};
t510 = ct{2714};
t5100 = ct{2715};
t5102 = ct{2716};
t5107 = ct{2717};
t511 = ct{2718};
t5111 = ct{2719};
t5112 = ct{2720};
t5113 = ct{2721};
t5114 = ct{2722};
t5116 = ct{2723};
t5119 = ct{2724};
t512 = ct{2725};
t5120 = ct{2726};
t5122 = ct{2727};
t5127 = ct{2728};
t513 = ct{2729};
t5130 = ct{2730};
t5139 = ct{2731};
t514 = ct{2732};
t5142 = ct{2733};
t5147 = ct{2734};
t5149 = ct{2735};
t5150 = ct{2736};
t5151 = ct{2737};
t5154 = ct{2738};
t5158 = ct{2739};
t516 = ct{2740};
t5165 = ct{2741};
t517 = ct{2742};
t5171 = ct{2743};
t5172 = ct{2744};
t5176 = ct{2745};
t5179 = ct{2746};
t518 = ct{2747};
t5180 = ct{2748};
t5181 = ct{2749};
t5183 = ct{2750};
t5184 = ct{2751};
t5185 = ct{2752};
t5186 = ct{2753};
t5187 = ct{2754};
t5192 = ct{2755};
t5193 = ct{2756};
t5199 = ct{2757};
t520 = ct{2758};
t5200 = ct{2759};
t5203 = ct{2760};
t5204 = ct{2761};
t5205 = ct{2762};
t5208 = ct{2763};
t521 = ct{2764};
t5215 = ct{2765};
t5216 = ct{2766};
t5217 = ct{2767};
t522 = ct{2768};
t5222 = ct{2769};
t5223 = ct{2770};
t5224 = ct{2771};
t5227 = ct{2772};
t523 = ct{2773};
t5236 = ct{2774};
t5237 = ct{2775};
t5238 = ct{2776};
t5239 = ct{2777};
t524 = ct{2778};
t5240 = ct{2779};
t5244 = ct{2780};
t5245 = ct{2781};
t525 = ct{2782};
t5250 = ct{2783};
t5252 = ct{2784};
t5258 = ct{2785};
t526 = ct{2786};
t5267 = ct{2787};
t527 = ct{2788};
t5270 = ct{2789};
t5271 = ct{2790};
t5279 = ct{2791};
t528 = ct{2792};
t5280 = ct{2793};
t5281 = ct{2794};
t5285 = ct{2795};
t529 = ct{2796};
t5293 = ct{2797};
t5294 = ct{2798};
t53 = ct{2799};
t530 = ct{2800};
t5305 = ct{2801};
t531 = ct{2802};
t5318 = ct{2803};
t5319 = ct{2804};
t532 = ct{2805};
t5321 = ct{2806};
t5324 = ct{2807};
t5325 = ct{2808};
t5327 = ct{2809};
t5328 = ct{2810};
t533 = ct{2811};
t5331 = ct{2812};
t5332 = ct{2813};
t534 = ct{2814};
t535 = ct{2815};
t5353 = ct{2816};
t5355 = ct{2817};
t5356 = ct{2818};
t5358 = ct{2819};
t536 = ct{2820};
t5361 = ct{2821};
t5362 = ct{2822};
t5364 = ct{2823};
t5368 = ct{2824};
t537 = ct{2825};
t5372 = ct{2826};
t5373 = ct{2827};
t5376 = ct{2828};
t5378 = ct{2829};
t538 = ct{2830};
t5387 = ct{2831};
t5389 = ct{2832};
t539 = ct{2833};
t5390 = ct{2834};
t5391 = ct{2835};
t5392 = ct{2836};
t5393 = ct{2837};
t5394 = ct{2838};
t540 = ct{2839};
t5402 = ct{2840};
t5404 = ct{2841};
t5409 = ct{2842};
t5416 = ct{2843};
t5420 = ct{2844};
t5424 = ct{2845};
t5429 = ct{2846};
t543 = ct{2847};
t5430 = ct{2848};
t5434 = ct{2849};
t5435 = ct{2850};
t5436 = ct{2851};
t5439 = ct{2852};
t544 = ct{2853};
t5440 = ct{2854};
t5441 = ct{2855};
t5445 = ct{2856};
t5449 = ct{2857};
t545 = ct{2858};
t5450 = ct{2859};
t5451 = ct{2860};
t5452 = ct{2861};
t5453 = ct{2862};
t5455 = ct{2863};
t5456 = ct{2864};
t5457 = ct{2865};
t546 = ct{2866};
t5467 = ct{2867};
t5468 = ct{2868};
t5469 = ct{2869};
t547 = ct{2870};
t5470 = ct{2871};
t5471 = ct{2872};
t5472 = ct{2873};
t5473 = ct{2874};
t5474 = ct{2875};
t5475 = ct{2876};
t5476 = ct{2877};
t5477 = ct{2878};
t5478 = ct{2879};
t548 = ct{2880};
t5489 = ct{2881};
t549 = ct{2882};
t5490 = ct{2883};
t5493 = ct{2884};
t5494 = ct{2885};
t5497 = ct{2886};
t5499 = ct{2887};
t5501 = ct{2888};
t5508 = ct{2889};
t551 = ct{2890};
t5510 = ct{2891};
t5512 = ct{2892};
t5516 = ct{2893};
t5517 = ct{2894};
t552 = ct{2895};
t5521 = ct{2896};
t553 = ct{2897};
t5532 = ct{2898};
t5535 = ct{2899};
t554 = ct{2900};
t5540 = ct{2901};
t5547 = ct{2902};
t555 = ct{2903};
t5557 = ct{2904};
t5558 = ct{2905};
t556 = ct{2906};
t557 = ct{2907};
t5574 = ct{2908};
t5578 = ct{2909};
t5579 = ct{2910};
t558 = ct{2911};
t5582 = ct{2912};
t5586 = ct{2913};
t559 = ct{2914};
t5590 = ct{2915};
t5593 = ct{2916};
t5596 = ct{2917};
t560 = ct{2918};
t5604 = ct{2919};
t5607 = ct{2920};
t561 = ct{2921};
t5612 = ct{2922};
t562 = ct{2923};
t5629 = ct{2924};
t563 = ct{2925};
t5634 = ct{2926};
t5635 = ct{2927};
t564 = ct{2928};
t567 = ct{2929};
t568 = ct{2930};
t5688 = ct{2931};
t569 = ct{2932};
t57 = ct{2933};
t570 = ct{2934};
t571 = ct{2935};
t572 = ct{2936};
t573 = ct{2937};
t574 = ct{2938};
t5741 = ct{2939};
t5743 = ct{2940};
t576 = ct{2941};
t577 = ct{2942};
t5777 = ct{2943};
t5779 = ct{2944};
t578 = ct{2945};
t5780 = ct{2946};
t5782 = ct{2947};
t579 = ct{2948};
t58 = ct{2949};
t580 = ct{2950};
t581 = ct{2951};
t582 = ct{2952};
t5826 = ct{2953};
t583 = ct{2954};
t584 = ct{2955};
t586 = ct{2956};
t587 = ct{2957};
t5886 = ct{2958};
t5887 = ct{2959};
t589 = ct{2960};
t5894 = ct{2961};
t59 = ct{2962};
t590 = ct{2963};
t591 = ct{2964};
t592 = ct{2965};
t593 = ct{2966};
t594 = ct{2967};
t595 = ct{2968};
t596 = ct{2969};
t597 = ct{2970};
t6 = ct{2971};
t60 = ct{2972};
t600 = ct{2973};
t602 = ct{2974};
t603 = ct{2975};
t604 = ct{2976};
t605 = ct{2977};
t609 = ct{2978};
t610 = ct{2979};
t611 = ct{2980};
t612 = ct{2981};
t613 = ct{2982};
t614 = ct{2983};
t615 = ct{2984};
t616 = ct{2985};
t618 = ct{2986};
t619 = ct{2987};
t622 = ct{2988};
t623 = ct{2989};
t624 = ct{2990};
t625 = ct{2991};
t626 = ct{2992};
t627 = ct{2993};
t628 = ct{2994};
t629 = ct{2995};
t63 = ct{2996};
t630 = ct{2997};
t631 = ct{2998};
t633 = ct{2999};
t634 = ct{3000};
t635 = ct{3001};
t636 = ct{3002};
t637 = ct{3003};
t638 = ct{3004};
t639 = ct{3005};
t640 = ct{3006};
t641 = ct{3007};
t642 = ct{3008};
t643 = ct{3009};
t648 = ct{3010};
t649 = ct{3011};
t650 = ct{3012};
t653 = ct{3013};
t654 = ct{3014};
t655 = ct{3015};
t656 = ct{3016};
t657 = ct{3017};
t658 = ct{3018};
t660 = ct{3019};
t662 = ct{3020};
t663 = ct{3021};
t664 = ct{3022};
t665 = ct{3023};
t667 = ct{3024};
t668 = ct{3025};
t673 = ct{3026};
t674 = ct{3027};
t675 = ct{3028};
t676 = ct{3029};
t678 = ct{3030};
t679 = ct{3031};
t681 = ct{3032};
t682 = ct{3033};
t683 = ct{3034};
t684 = ct{3035};
t685 = ct{3036};
t686 = ct{3037};
t687 = ct{3038};
t688 = ct{3039};
t689 = ct{3040};
t693 = ct{3041};
t694 = ct{3042};
t695 = ct{3043};
t696 = ct{3044};
t697 = ct{3045};
t698 = ct{3046};
t7 = ct{3047};
t700 = ct{3048};
t702 = ct{3049};
t703 = ct{3050};
t704 = ct{3051};
t705 = ct{3052};
t706 = ct{3053};
t71 = ct{3054};
t710 = ct{3055};
t711 = ct{3056};
t712 = ct{3057};
t713 = ct{3058};
t715 = ct{3059};
t716 = ct{3060};
t72 = ct{3061};
t724 = ct{3062};
t728 = ct{3063};
t73 = ct{3064};
t731 = ct{3065};
t733 = ct{3066};
t734 = ct{3067};
t735 = ct{3068};
t736 = ct{3069};
t74 = ct{3070};
t741 = ct{3071};
t742 = ct{3072};
t743 = ct{3073};
t744 = ct{3074};
t746 = ct{3075};
t747 = ct{3076};
t748 = ct{3077};
t749 = ct{3078};
t75 = ct{3079};
t750 = ct{3080};
t751 = ct{3081};
t752 = ct{3082};
t754 = ct{3083};
t755 = ct{3084};
t756 = ct{3085};
t757 = ct{3086};
t758 = ct{3087};
t759 = ct{3088};
t76 = ct{3089};
t760 = ct{3090};
t762 = ct{3091};
t763 = ct{3092};
t764 = ct{3093};
t765 = ct{3094};
t766 = ct{3095};
t767 = ct{3096};
t768 = ct{3097};
t769 = ct{3098};
t77 = ct{3099};
t772 = ct{3100};
t773 = ct{3101};
t774 = ct{3102};
t775 = ct{3103};
t776 = ct{3104};
t777 = ct{3105};
t778 = ct{3106};
t779 = ct{3107};
t780 = ct{3108};
t781 = ct{3109};
t782 = ct{3110};
t784 = ct{3111};
t785 = ct{3112};
t786 = ct{3113};
t790 = ct{3114};
t792 = ct{3115};
t794 = ct{3116};
t795 = ct{3117};
t796 = ct{3118};
t798 = ct{3119};
t8 = ct{3120};
t80 = ct{3121};
t801 = ct{3122};
t804 = ct{3123};
t805 = ct{3124};
t806 = ct{3125};
t808 = ct{3126};
t81 = ct{3127};
t814 = ct{3128};
t815 = ct{3129};
t817 = ct{3130};
t82 = ct{3131};
t820 = ct{3132};
t822 = ct{3133};
t825 = ct{3134};
t827 = ct{3135};
t83 = ct{3136};
t831 = ct{3137};
t832 = ct{3138};
t833 = ct{3139};
t834 = ct{3140};
t835 = ct{3141};
t836 = ct{3142};
t837 = ct{3143};
t838 = ct{3144};
t84 = ct{3145};
t840 = ct{3146};
t841 = ct{3147};
t842 = ct{3148};
t843 = ct{3149};
t846 = ct{3150};
t86 = ct{3151};
t863 = ct{3152};
t868 = ct{3153};
t869 = ct{3154};
t870 = ct{3155};
t874 = ct{3156};
t878 = ct{3157};
t880 = ct{3158};
t881 = ct{3159};
t882 = ct{3160};
t884 = ct{3161};
t885 = ct{3162};
t888 = ct{3163};
t889 = ct{3164};
t891 = ct{3165};
t892 = ct{3166};
t895 = ct{3167};
t899 = ct{3168};
t9 = ct{3169};
t90 = ct{3170};
t900 = ct{3171};
t903 = ct{3172};
t906 = ct{3173};
t91 = ct{3174};
t911 = ct{3175};
t921 = ct{3176};
t922 = ct{3177};
t923 = ct{3178};
t925 = ct{3179};
t926 = ct{3180};
t927 = ct{3181};
t929 = ct{3182};
t934 = ct{3183};
t935 = ct{3184};
t936 = ct{3185};
t937 = ct{3186};
t940 = ct{3187};
t941 = ct{3188};
t942 = ct{3189};
t946 = ct{3190};
t949 = ct{3191};
t95 = ct{3192};
t950 = ct{3193};
t954 = ct{3194};
t955 = ct{3195};
t957 = ct{3196};
t958 = ct{3197};
t961 = ct{3198};
t962 = ct{3199};
t964 = ct{3200};
t965 = ct{3201};
t968 = ct{3202};
t97 = ct{3203};
t970 = ct{3204};
t971 = ct{3205};
t972 = ct{3206};
t973 = ct{3207};
t975 = ct{3208};
t977 = ct{3209};
t982 = ct{3210};
t983 = ct{3211};
t984 = ct{3212};
t986 = ct{3213};
t987 = ct{3214};
t988 = ct{3215};
t989 = ct{3216};
t99 = ct{3217};
t993 = ct{3218};
t994 = ct{3219};
t995 = ct{3220};
t999 = ct{3221};
t4494 = -t4417;
t4496 = -t4425;
t4497 = -t4426;
t4499 = -t4428;
t4500 = -t4429;
t4503 = t5.*t4365;
t4505 = t17.*t4230;
t4507 = t5.*t4295;
t4510 = t9.*t4295;
t4511 = t9.*t4296;
t4512 = t8.*t4298;
t4514 = -t4443;
t4515 = -t4444;
t4518 = -t4446;
t4521 = -t4452;
t4523 = t8.*t17.*t4179;
t4526 = -t4457;
t4527 = -t4459;
t4529 = -t4462;
t4531 = t8.*t22.*t4179;
t4534 = -t4478;
t4535 = -t4480;
t4537 = t8.*t4419;
t4538 = -t4488;
t4539 = -t4491;
t4541 = t8.*t4425;
t4544 = -t4492;
t4545 = t3.*t4.*t7.*t4179;
t4546 = -t4501;
t4550 = t18.*t4278;
t4552 = -t4509;
t4553 = t8.*t4369;
t4556 = t8.*t4370;
t4560 = -t4517;
t4564 = t3.*t4.*t7.*t4230;
t4565 = -t4522;
t4573 = -t4533;
t4576 = -t4540;
t4578 = -t4542;
t4580 = -t4543;
t4586 = t8.*t22.*t4230;
t4587 = -t4548;
t4592 = -t4555;
t4593 = -t4557;
t4594 = -t4558;
t4597 = -t4561;
t4598 = -t4562;
t4599 = -t4563;
t4602 = -t4568;
t4603 = -t4571;
t4604 = -t4572;
t4608 = t17.*t18.*t4179;
t4609 = -t4574;
t4610 = -t4575;
t4612 = -t4579;
t4613 = t18.*t4405;
t4615 = -t4583;
t4618 = -t4588;
t4619 = t17.*t18.*t4185;
t4620 = -t4589;
t4623 = t17.*t18.*t4190;
t4624 = -t4596;
t4627 = -t4600;
t4631 = -t4611;
t4635 = -t4616;
t4654 = -t4625;
t4655 = -t4626;
t4659 = -t4628;
t4664 = -t4630;
t4665 = -t4636;
t4668 = -t4640;
t4670 = -t4641;
t4671 = -t4642;
t4676 = -t4651;
t4677 = -t4653;
t4678 = -t4656;
t4679 = -t4658;
t4680 = -t4662;
t4681 = -t4663;
t4682 = t8.*t4633;
t4683 = t4.*t4637;
t4684 = t4.*t4639;
t4685 = t8.*t4637;
t4686 = t8.*t4639;
t4687 = t8.*t4640;
t4689 = -t4666;
t4690 = t8.*t4641;
t4698 = -t4674;
t4699 = t4.*t4661;
t4700 = t8.*t4657;
t4701 = t8.*t4658;
t4702 = -t4675;
t4703 = t8.*t4661;
t4704 = t8.*t4662;
t4705 = t8.*t4663;
t4710 = -t4688;
t4712 = -t4691;
t4714 = t4.*t4650;
t4715 = -t4695;
t4717 = t4.*t4652;
t4718 = t8.*t4650;
t4719 = t4.*t4657;
t4720 = t8.*t4652;
t4721 = t8.*t4653;
t4729 = -t4707;
t4730 = -t4708;
t4736 = -t4728;
t4738 = -t4733;
t4739 = t8.*t4728;
t4746 = -t4737;
t4750 = -t4740;
t4751 = -t4741;
t4757 = -t4747;
t4762 = -t4749;
t4765 = -t4752;
t4768 = -t4756;
t4771 = -t4758;
t4772 = -t4759;
t4773 = -t4760;
t4774 = -t4761;
t4775 = -t4766;
t4776 = -t4769;
t4779 = -t4770;
t4780 = -t4777;
t4781 = -t4778;
t4784 = -t4782;
t4787 = -t4785;
t4791 = -t4788;
t4792 = -t4790;
t4793 = t7.*t9.*t34.*t191.*t196.*9.098517085411002e-23;
t4802 = -t4794;
t4806 = -t4796;
t4809 = -t4798;
t4810 = (t1427.*t1460)./2.0;
t4812 = -t4800;
t4819 = t7.*t24.*t34.*t191.*t196.*2.829693476925513e-22;
t4821 = t7.*t34.*t191.*t196.*3.841105500485731e-25;
t4826 = -t4804;
t4829 = -t4807;
t4831 = -t4808;
t4836 = t8.*t4798;
t4840 = t5.*t7.*t9.*t34.*t191.*t196.*3.719939515191737e-22;
t4847 = t5.*t7.*t34.*t191.*t196.*4.945250784909262e-23;
t4848 = -t4813;
t4851 = t7.*t19.*t34.*t191.*t196.*2.829693476925513e-22;
t4853 = -t4815;
t4856 = t8.*t4803;
t4857 = t5.*t4804;
t4860 = t8.*t4807;
t4863 = -t4827;
t4868 = -t4828;
t4869 = -t4830;
t4870 = -t4832;
t4874 = t5.*t18.*t34.*t191.*t196.*1.530369361342075e-22;
t4875 = -t4835;
t4880 = t5.*t23.*t34.*t191.*t196.*1.530369361342075e-22;
t4885 = t5.*t4811;
t4888 = -t4839;
t4893 = -t4845;
t4903 = -t4849;
t4904 = (t1429.*t1471)./2.0;
t4907 = -t4852;
t4912 = t5.*t4825;
t4914 = t8.*t4824;
t4918 = t8.*t4828;
t4921 = t8.*t4830;
t4922 = -t4861;
t4929 = -t4871;
t4931 = -t4873;
t4935 = -t4879;
t4936 = -t4878;
t4940 = t8.*t4839;
t4949 = -t4883;
t4950 = -t4882;
t4952 = -t4887;
t4953 = -t4886;
t4963 = t18.*t4798;
t4968 = t18.*t4799;
t4975 = -t4897;
t4978 = -t4899;
t4979 = -t4900;
t4989 = -t4910;
t4990 = -t4909;
t4992 = -t4913;
t4994 = -t4915;
t4995 = -t4916;
t4997 = t9.*t4862;
t5002 = t8.*t4866;
t5003 = t8.*t4867;
t5005 = t5.*t4871;
t5007 = -t4919;
t5009 = -t4923;
t5010 = t7.*t9.*t18.*t34.*t191.*t196.*(-9.098517085411002e-23);
t5011 = t8.*t4878;
t5012 = t8.*t4879;
t5014 = -t4928;
t5015 = -t4930;
t5016 = -t4937;
t5017 = -t4938;
t5018 = t5.*t34.*t191.*t196.*3.002769355787804e-29;
t5020 = -t4941;
t5024 = -t4945;
t5030 = t9.*t34.*t191.*t197.*3.002769355787804e-29;
t5031 = -t4956;
t5032 = -t4955;
t5039 = -t4962;
t5041 = t5.*t9.*t18.*t34.*t191.*t196.*2.379770328738529e-22;
t5048 = t5.*t9.*t23.*t34.*t191.*t196.*2.379770328738529e-22;
t5054 = t18.*t19.*t34.*t191.*t196.*1.564233326885588e-22;
t5055 = -t4976;
t5056 = -t4980;
t5058 = -t4983;
t5059 = t19.*t23.*t34.*t191.*t196.*1.564233326885588e-22;
t5061 = -t4986;
t5067 = t9.*t23.*t34.*t191.*t196.*8.317905230417136e-23;
t5074 = -t4999;
t5075 = -t4998;
t5076 = -t5004;
t5077 = t7.*t18.*t19.*t34.*t191.*t196.*1.414846738462756e-22;
t5081 = t7.*t18.*t24.*t34.*t191.*t196.*1.414846738462756e-22;
t5088 = t8.*t4942;
t5089 = t9.*t4941;
t5090 = t8.*t4943;
t5101 = t18.*t4828;
t5106 = t18.*t4833;
t5108 = t9.*t4964;
t5109 = -t5034;
t5110 = -t5038;
t5121 = t8.*t4973;
t5123 = -t5046;
t5125 = t5.*t7.*t9.*t18.*t34.*t191.*t196.*1.859969757595868e-22;
t5129 = t8.*t4986;
t5131 = -t5053;
t5132 = -t5052;
t5136 = -t5060;
t5138 = t9.*t18.*t34.*t191.*t196.*8.317905230417136e-23;
t5140 = -t5062;
t5143 = -t5069;
t5146 = -t5071;
t5148 = -t5072;
t5152 = t9.*t34.*t191.*t196.*3.937746659416635e-29;
t5153 = t5.*t34.*t191.*t197.*3.937746659416635e-29;
t5157 = -t5082;
t5164 = t8.*t5021;
t5166 = t8.*t5022;
t5174 = -t5095;
t5175 = -t5096;
t5189 = -t5111;
t5191 = -t5116;
t5195 = -t5122;
t5201 = -t5127;
t5202 = -t5130;
t5206 = t8.*t5063;
t5207 = t8.*t5064;
t5209 = t9.*t5062;
t5210 = t8.*t5065;
t5211 = t8.*t5066;
t5218 = -t5142;
t5219 = -t5149;
t5229 = -t5158;
t5233 = -t5165;
t5242 = -t5176;
t5247 = -t5179;
t5248 = -t5180;
t5249 = t8.*t5112;
t5251 = t8.*t5114;
t5255 = -t5186;
t5257 = t5.*t18.*t34.*t191.*t196.*6.005538711575609e-29;
t5261 = -t5193;
t5262 = -t5192;
t5265 = t9.*t18.*t34.*t191.*t197.*6.005538711575609e-29;
t5268 = t18.*t34.*t191.*t196.*5.632647031707275e-23;
t5269 = -t5208;
t5272 = t23.*t34.*t191.*t196.*5.632647031707275e-23;
t5288 = t7.*t9.*t18.*t34.*t191.*t196.*3.570477686932346e-29;
t5289 = t8.*t5179;
t5292 = t7.*t9.*t23.*t34.*t191.*t196.*3.570477686932346e-29;
t5295 = -t5245;
t5297 = -t5250;
t5302 = -t5267;
t5306 = -t5271;
t5320 = -t5281;
t5339 = -t5305;
t5344 = -t5319;
t5346 = t9.*t18.*t34.*t191.*t196.*7.875493318833269e-29;
t5347 = t5.*t18.*t34.*t191.*t197.*7.875493318833269e-29;
t5348 = -t5325;
t5349 = -t5328;
t5351 = -t5332;
t5365 = t5.*t7.*t18.*t34.*t191.*t196.*4.682223280699094e-29;
t5366 = t8.*t5325;
t5367 = t5.*t7.*t23.*t34.*t191.*t196.*4.682223280699094e-29;
t5375 = -t5353;
t5383 = -t5362;
t5395 = -t5376;
t5433 = -t5424;
t5442 = -t5430;
t5443 = -t5429;
t5444 = t7.*t18.*t34.*t191.*t196.*8.273795699471084e-23;
t5446 = t18.*t34.*t191.*t197.*1.391651334125335e-22;
t5448 = t7.*t23.*t34.*t191.*t196.*8.273795699471084e-23;
t5454 = -t5434;
t5459 = -t5439;
t5463 = -t5449;
t5464 = -t5452;
t5465 = -t5455;
t5466 = -t5456;
t5479 = -t5468;
t5480 = -t5467;
t5481 = -t5470;
t5482 = -t5469;
t5483 = -t5471;
t5484 = -t5472;
t5485 = -t5474;
t5486 = -t5476;
t5487 = -t5477;
t5488 = -t5478;
t5491 = t9.*t34.*t191.*t196.*7.316193564301157e-22;
t5492 = t5.*t34.*t191.*t197.*7.316193564301157e-22;
t5496 = t5.*t34.*t191.*t196.*3.976517450785667e-22;
t5498 = t9.*t34.*t191.*t197.*3.976517450785667e-22;
t5507 = -t5497;
t5519 = -t5508;
t5522 = t34.*t191.*t196.*3.090224797147319e-22;
t5526 = -t5510;
t5527 = t7.*t34.*t191.*t196.*4.739633201158597e-25;
t5534 = t9.*t34.*t191.*t197.*3.069039723904487e-29;
t5546 = -t5532;
t5549 = -t5535;
t5552 = t18.*t5508;
t5555 = -t5547;
t5559 = t5.*t34.*t191.*t197.*4.024651742608185e-29;
t5561 = t34.*t191.*t197.*7.032484625216972e-23;
t5562 = t9.*t18.*t34.*t191.*t197.*6.138079447808974e-29;
t5563 = t17.*t18.*t5494;
t5565 = -t5557;
t5566 = -t5558;
t5569 = t17.*t18.*t5493;
t5573 = t18.*t5547;
t5580 = -t5574;
t5581 = t5.*t18.*t34.*t191.*t197.*8.04930348521637e-29;
t5583 = -t5579;
t5584 = -t5582;
t5589 = -t5586;
t5594 = t18.*t34.*t191.*t197.*1.42236473075195e-22;
t5597 = t2442+t2450;
t5600 = -t3.*(t2444-t2449);
t5603 = t9.*t34.*t191.*t196.*7.477660125089319e-22;
t5606 = t5.*t34.*t191.*t196.*4.064278195638759e-22;
t5611 = t34.*t191.*t196.*3.158425284965513e-22;
t5618 = t34.*t191.*t197.*7.187689800729284e-23;
t5633 = t215+t5358;
t5656 = t3218+t3231;
t5660 = t3230+t3244;
t5667 = -t3.*(t3219-t3230);
t5668 = -t7.*(t3219-t3230);
t5673 = -t4.*(t3231-t3243);
t5674 = -t8.*(t3231-t3243);
t5678 = t8.*(t3231-t3243);
t5818 = -t5.*((t197.*(t29-t30))./9.007199254740992e+15+t3.*(t3219-t3230));
t5819 = -t9.*((t197.*(t29-t30))./9.007199254740992e+15+t3.*(t3219-t3230));
t5823 = t136+t143+t145+t147+t166+t173+t175+t183+t186+t193;
t7148 = t892+t936+t1012+t1027+t1033+t1041+t1064+t1071+t1094+t1097+t1123+t1132+t1140+t1151+t1161+t1166+t1176+t1187+t1195+t1208+t1223+t1226+t1229+t1230+t1232+t1242+t1260+t1276+t1279+t1287+t1297+t1320+t1321+t1332+t1339+t1347+t1358+t1368+t1373+t1387+t1405+t1418+t1421+t1424+t1434+t1444+t1469+t1485+t1695+t1744+t1826+t1872+t2103+t2179+t2294+t2506;
t203 = -t200;
t208 = t5.*t199.*(3.0./5.0e+2);
t209 = t9.*t199.*(3.0./5.0e+2);
t210 = t5.*t200.*(3.0./5.0e+2);
t211 = t5.*t201.*(3.0./5.0e+2);
t212 = t9.*t200.*(3.0./5.0e+2);
t213 = t9.*t201.*(3.0./5.0e+2);
t620 = -t616;
t621 = -t619;
t632 = -t624;
t645 = t200.*3.06620924912759e-3;
t646 = t201.*3.06620924912759e-3;
t647 = t202.*3.06620924912759e-3;
t669 = -t654;
t680 = t5.*t653;
t691 = t200.*2.10046025307537e-6;
t692 = t201.*2.10046025307537e-6;
t708 = -t678;
t738 = t72.*t199;
t739 = t73.*t199;
t740 = t5.*t200.*4.00912737776847e-7;
t753 = t72.*t202;
t797 = t201.*8.79383415291399e-9;
t799 = t9.*t678;
t802 = t5.*t200.*(-8.01825475553694e-7);
t823 = t5.*t199.*(-4.36041e-5);
t824 = t9.*t200.*(-4.36041e-5);
t826 = -t790;
t829 = -t794;
t830 = t200.*(-1.758766830582798e-8);
t844 = t5.*t9.*t200.*2.493725402181286e-6;
t845 = t5.*t9.*t201.*2.493725402181286e-6;
t847 = t5.*t9.*t199.*1.639136489385872e-6;
t852 = t5.*t9.*t202.*8.195682446929358e-7;
t853 = t5.*t9.*t202.*1.639136489385872e-6;
t856 = t19.*t199.*2.493725402181286e-6;
t858 = t19.*t202.*1.246862701090643e-6;
t859 = t19.*t202.*2.493725402181286e-6;
t860 = t112.*t199;
t861 = t113.*t199;
t865 = t19.*t200.*8.195682446929358e-7;
t866 = t19.*t201.*8.195682446929358e-7;
t867 = t9.*t200.*2.179051830709965e-7;
t871 = t112.*t202;
t875 = t24.*t200.*8.195682446929358e-7;
t876 = t24.*t201.*8.195682446929358e-7;
t877 = t121.*t199;
t902 = t23.*t710;
t909 = t5.*t199.*(-4.35810366141993e-7);
t910 = t5.*t199.*(-2.179051830709965e-7);
t914 = t9.*t200.*(-4.35810366141993e-7);
t916 = t5.*t202.*(-4.35810366141993e-7);
t917 = t5.*t202.*(-2.179051830709965e-7);
t920 = t130.*t199;
t928 = t18.*t794;
t930 = -t889;
t933 = t23.*t794;
t943 = t8.*t19.*t199.*1.246862701090643e-6;
t944 = t18.*t767;
t945 = t199.*1.244337995057065e-6;
t947 = t8.*t24.*t199.*1.246862701090643e-6;
t948 = t23.*t767;
t951 = t134.*t199;
t952 = t202.*6.221689975285323e-7;
t953 = t202.*1.244337995057065e-6;
t963 = t9.*t202.*1.573278338878372e-13;
t974 = t5.*t8.*t9.*t199.*(-1.639136489385872e-6);
t976 = t23.*t831;
t991 = t23.*t817;
t1017 = t9.*t199.*1.573278338878372e-13;
t1019 = t5.*t200.*1.573278338878372e-13;
t1020 = t140.*t200;
t1021 = t5.*t201.*1.573278338878372e-13;
t1036 = -t973;
t1072 = t8.*t9.*t199.*6.293113355513489e-13;
t1075 = -t1009;
t1077 = -t1010;
t1087 = t9.*t199.*(-3.146556677756745e-13);
t1089 = t5.*t201.*(-3.146556677756745e-13);
t1135 = t5.*t199.*2.063152639848858e-13;
t1145 = t9.*t200.*2.063152639848858e-13;
t1147 = t9.*t201.*2.063152639848858e-13;
t1149 = t5.*t202.*2.063152639848858e-13;
t1165 = t8.*t201.*(-5.902365793397849e-7);
t1194 = -t1120;
t1200 = t5.*t199.*(-4.126305279697715e-13);
t1202 = t202.*4.481269837999131e+48;
t1211 = t9.*t200.*(-4.126305279697715e-13);
t1235 = t199.*8.769009823985418e+48;
t1237 = t200.*8.769009823985418e+48;
t1239 = t202.*8.769009823985418e+48;
t1241 = t5.*t8.*t199.*8.252610559395431e-13;
t1311 = t5.*t199.*(-8.4155913e-14);
t1317 = t9.*t199.*(-8.4155913e-14);
t1318 = t9.*t200.*(-8.4155913e-14);
t1441 = t8.*t199.*1.458290424491263e-6;
t1446 = -t1439;
t1465 = -t1458;
t1490 = t25.*t1468;
t1491 = t26.*t1468;
t1493 = t2.*t199.*2.591581422298263e-2;
t1495 = t6.*t199.*1.069035573404174e-1;
t1500 = t200.*6.0e-3;
t1507 = t199.*8.851959439560906e-2;
t1509 = t200.*8.851959439560906e-2;
t1510 = t5.*t1492;
t1512 = t9.*t1492;
t1526 = t5.*t1499;
t1540 = t201.*1.07340844256743e-6;
t1564 = t200.*8.987911871652987e-9;
t1576 = t5.*t200.*(-8.851959439560906e-2);
t1577 = t9.*t1524;
t1579 = t5.*t201.*2.228321578664739e-5;
t1582 = t199.*t239;
t1583 = t199.*t240;
t1584 = t5.*t201.*2.048803907774054e-7;
t1585 = t5.*t201.*4.097607815548108e-7;
t1586 = t9.*t201.*2.228321578664739e-5;
t1588 = t202.*t239;
t1601 = t200.*4.493955935826494e-9;
t1602 = t201.*4.493955935826494e-9;
t1616 = t8.*t199.*7.452373505947646e-7;
t1626 = t5.*t8.*t201.*8.195215631096216e-7;
t1647 = t9.*t202.*(-2.048803907774054e-7);
t1648 = -t1590;
t1667 = -t1607;
t1675 = t5.*t9.*t199.*8.376559107229145e-7;
t1686 = t5.*t9.*t202.*4.188279553614573e-7;
t1690 = t199.*t277;
t1691 = t199.*t278;
t1699 = t9.*t201.*1.11357147960855e-7;
t1700 = t9.*t201.*2.227142959217101e-7;
t1701 = t202.*t277;
t1710 = -t1630;
t1715 = t19.*t201.*4.188279553614573e-7;
t1718 = -t1642;
t1721 = t24.*t201.*4.188279553614573e-7;
C_dq = ft_9({dq1,dq2,dq3,dq4,dq5,dq6,t1004,t1006,t1008,t101,t1013,t1016,t1017,t1019,t102,t1020,t1021,t1023,t1024,t1025,t1026,t1028,t1030,t1032,t1034,t1036,t1038,t1039,t1040,t1042,t1043,t1044,t1045,t1046,t1047,t1048,t1049,t1050,t1051,t1054,t1055,t1056,t1057,t1059,t1061,t1065,t1066,t1068,t1069,t1070,t1072,t1073,t1075,t1076,t1077,t1081,t1083,t1084,t1085,t1087,t1089,t1091,t1092,t1093,t1095,t1098,t1099,t110,t1101,t1102,t1105,t1106,t1107,t1108,t1109,t111,t1113,t1115,t1116,t1119,t112,t1122,t1125,t1126,t1127,t1128,t113,t1130,t1131,t1133,t1134,t1135,t1138,t1139,t114,t1141,t1144,t1145,t1146,t1147,t1148,t1149,t115,t1150,t1152,t1153,t1155,t1158,t1159,t116,t1162,t1163,t1165,t1167,t1169,t1170,t1171,t1173,t1174,t1175,t1177,t1178,t1179,t1180,t1181,t1182,t1183,t1184,t1185,t1186,t1188,t1189,t1190,t1191,t1192,t1193,t1194,t1196,t1197,t1198,t1199,t120,t1200,t1202,t1203,t1204,t1205,t1206,t1207,t121,t1210,t1211,t1215,t1219,t1221,t1222,t1224,t1225,t1227,t1228,t1233,t1235,t1236,t1237,t1239,t124,t1240,t1241,t1244,t1245,t125,t1250,t1251,t1253,t1254,t1256,t1257,t1258,t1259,t126,t1261,t1262,t1263,t1264,t1265,t1266,t1267,t1268,t1269,t1271,t1272,t1273,t1274,t1277,t1278,t128,t1280,t1282,t1285,t1286,t1288,t129,t1290,t1293,t1294,t1295,t1296,t1298,t1300,t1301,t1302,t1306,t1307,t1308,t1309,t131,t1311,t1312,t1313,t1315,t1316,t1317,t1318,t1319,t132,t1322,t1323,t1324,t1325,t1326,t1328,t1329,t133,t1330,t1331,t1333,t1334,t1337,t1338,t1340,t1341,t1342,t1343,t1344,t1345,t1346,t1348,t1351,t1352,t1353,t1354,t1355,t1356,t1360,t1362,t1365,t1366,t1367,t1369,t1370,t1371,t1372,t1374,t1375,t1377,t1378,t1379,t1380,t1383,t1384,t1385,t1386,t1388,t1389,t139,t1391,t1392,t1393,t1394,t1397,t1398,t140,t1401,t1402,t1403,t1404,t1406,t1407,t1408,t1409,t141,t1410,t1411,t1413,t1414,t1415,t1416,t1417,t1419,t142,t1422,t1423,t1426,t1427,t1428,t1429,t1430,t1431,t1432,t1433,t1436,t144,t1440,t1441,t1442,t1443,t1445,t1446,t1447,t1448,t1449,t1451,t1452,t1453,t1454,t1455,t1456,t1457,t1458,t1459,t1460,t1463,t1464,t1465,t1467,t1470,t1471,t1474,t1476,t1478,t1479,t148,t1480,t1481,t1482,t1483,t1486,t1487,t1488,t1489,t1490,t1491,t1492,t1493,t1494,t1495,t1496,t1498,t1499,t15,t150,t1500,t1501,t1503,t1505,t1506,t1507,t1508,t1509,t151,t1510,t1511,t1512,t1513,t1515,t1517,t1520,t1521,t1522,t1523,t1524,t1526,t1527,t1529,t153,t1530,t1531,t1532,t1533,t1534,t1535,t1536,t1537,t1538,t1539,t154,t1540,t1541,t1542,t1548,t1549,t1550,t1551,t1553,t1557,t1558,t156,t1560,t1561,t1562,t1564,t1566,t1567,t1568,t157,t1570,t1571,t1572,t1574,t1575,t1576,t1577,t1578,t1579,t158,t1580,t1581,t1582,t1583,t1584,t1585,t1586,t1587,t1589,t1590,t1591,t1592,t1593,t1594,t1595,t1596,t1597,t1598,t1599,t16,t1601,t1602,t1605,t1606,t1607,t1609,t161,t1610,t1611,t1612,t1613,t1614,t1615,t1616,t1617,t1618,t1619,t1620,t1621,t1622,t1624,t1625,t1626,t1627,t163,t1630,t1631,t1632,t1633,t1635,t1636,t1637,t1638,t1639,t1641,t1642,t1643,t1644,t1645,t1646,t1647,t1648,t1649,t165,t1651,t1652,t1653,t1657,t1658,t1659,t166,t1660,t1661,t1662,t1663,t1665,t1666,t1667,t1669,t1670,t1671,t1672,t1673,t1674,t1675,t1676,t1681,t1682,t1683,t1686,t1687,t1689,t1691,t1692,t1696,t1697,t1698,t1699,t17,t170,t1700,t1701,t1702,t1703,t1704,t1705,t1706,t1709,t171,t1710,t1711,t1712,t1713,t1715,t1716,t1718,t1719,t1720,t1721,t1722,t1724,t1726,t1728,t1729,t1731,t1733,t1734,t1735,t1736,t1737,t1738,t1739,t1740,t1743,t1745,t1746,t1748,t1749,t1752,t1755,t1756,t1757,t1758,t1759,t1760,t1761,t1763,t1764,t1767,t1769,t177,t1770,t1771,t1772,t1773,t1774,t1775,t1776,t1779,t1780,t1782,t1783,t1784,t1785,t1786,t1787,t1788,t1789,t1791,t1792,t1793,t1795,t1797,t1798,t1799,t18,t1800,t1801,t1802,t1804,t1806,t1807,t1808,t1809,t1810,t1811,t1812,t1813,t1814,t1816,t1817,t1820,t1822,t1823,t1824,t1825,t1827,t1828,t1829,t183,t1830,t1831,t1832,t1833,t1834,t1835,t1836,t1837,t1838,t1839,t1844,t1847,t1849,t185,t1850,t1851,t1854,t1855,t1857,t1858,t1859,t1862,t1864,t1865,t1866,t1867,t1871,t1873,t1877,t1879,t1880,t1881,t1882,t1884,t1887,t1889,t1892,t1893,t1896,t19,t190,t1903,t1904,t1906,t1907,t1908,t1909,t191,t1910,t1911,t1912,t1913,t1914,t1915,t1916,t1919,t1920,t1921,t1925,t1926,t1930,t1935,t1936,t1937,t1938,t1939,t1943,t1944,t1946,t1950,t1955,t196,t1961,t1966,t1967,t1968,t1969,t197,t1970,t1971,t1973,t1976,t1977,t1978,t1979,t1980,t1981,t1984,t1988,t199,t1992,t1993,t1994,t1995,t1996,t1997,t1998,t1999,t2,t20,t200,t2000,t2001,t2002,t2003,t2004,t2005,t2006,t2008,t201,t2014,t2016,t2017,t2019,t202,t2020,t2021,t2023,t2024,t2028,t2029,t203,t2033,t2036,t2037,t2038,t204,t2040,t2041,t2042,t2044,t2047,t205,t2051,t2052,t2053,t2054,t2055,t2056,t2057,t2058,t2059,t206,t2060,t2061,t2062,t2065,t2066,t2067,t2068,t2069,t207,t2070,t2071,t2072,t2073,t2074,t2076,t2077,t2078,t2079,t208,t2080,t2081,t2082,t2083,t2084,t2085,t2086,t2087,t2088,t2089,t209,t2091,t2092,t2093,t2094,t2095,t2096,t2097,t2098,t2099,t21,t210,t2100,t2101,t2104,t2105,t2106,t2107,t2108,t2109,t211,t2110,t2111,t2113,t2114,t2115,t2116,t2117,t2118,t2119,t212,t2121,t2125,t2128,t2129,t213,t2130,t2131,t2132,t2133,t2135,t2136,t2139,t2140,t2141,t2142,t2144,t2147,t2148,t2149,t2150,t2151,t2154,t2155,t2156,t2157,t2158,t2159,t2162,t2163,t2166,t2167,t2168,t2169,t2170,t2171,t2172,t2174,t2175,t2176,t2177,t2178,t2180,t2182,t2184,t2185,t2186,t2187,t2189,t2190,t2191,t2192,t2194,t2195,t2196,t22,t2200,t2201,t2203,t2204,t2208,t2209,t2210,t2212,t2214,t2217,t2218,t2219,t2220,t2221,t2223,t2225,t2227,t2228,t2229,t2231,t2232,t2236,t2237,t2239,t224,t2240,t2243,t2246,t2249,t225,t2250,t2251,t2252,t2254,t2255,t2256,t2257,t2264,t2265,t2266,t2267,t2269,t227,t2270,t2271,t2272,t2273,t2274,t2276,t2277,t2278,t2279,t228,t2280,t2281,t2282,t2283,t2284,t2285,t2286,t2287,t2291,t2292,t2295,t23,t230,t2302,t2304,t2305,t2306,t2307,t2308,t2309,t231,t2310,t2311,t2312,t2314,t2316,t2317,t2318,t2321,t2322,t2323,t2324,t233,t2331,t2333,t2334,t2335,t2336,t2337,t2338,t2339,t234,t2340,t2341,t2342,t2344,t2347,t2348,t235,t2350,t2351,t2355,t2357,t2358,t2359,t236,t2361,t2362,t2363,t2364,t2365,t2366,t2368,t2369,t2370,t2371,t2372,t2373,t2374,t2375,t2376,t2377,t2378,t2379,t2381,t2382,t2384,t2385,t2387,t2388,t2389,t2390,t2391,t2392,t2394,t2395,t2396,t2397,t24,t240,t2400,t2401,t2402,t2403,t2405,t2406,t2407,t2410,t2417,t2421,t2422,t2423,t2425,t2427,t2428,t2429,t243,t2430,t2431,t2434,t2435,t2437,t2438,t2439,t244,t2440,t2441,t2443,t2444,t2445,t2446,t2449,t2452,t2453,t2454,t2455,t2456,t2457,t2458,t2459,t2460,t2461,t2463,t2464,t2466,t2467,t2469,t2470,t2471,t2472,t2474,t2477,t2478,t2480,t2481,t2482,t2483,t2484,t2485,t2486,t2487,t2489,t249,t2495,t2497,t25,t2500,t2502,t2503,t2505,t2507,t2508,t2509,t2510,t2511,t2512,t2513,t2517,t2518,t2519,t2520,t2521,t2522,t2523,t2524,t2525,t2526,t2527,t2530,t2531,t2532,t2533,t2535,t2536,t2537,t2539,t2540,t2541,t2543,t2544,t2545,t2546,t2548,t2549,t2550,t2552,t2553,t2554,t2555,t2556,t2560,t2562,t2563,t2564,t2565,t2566,t2567,t2568,t2569,t257,t2570,t2571,t2574,t2575,t2576,t2577,t2578,t2579,t258,t2580,t2581,t2582,t2585,t2586,t2587,t2588,t2589,t2590,t2595,t2597,t2598,t2599,t26,t2600,t2601,t2602,t2603,t2604,t2606,t2607,t2608,t2611,t2612,t2615,t2616,t2617,t2627,t263,t2633,t2634,t2636,t2639,t2640,t2641,t2654,t2655,t2656,t2659,t266,t2666,t2668,t2669,t2671,t2673,t2675,t2676,t2677,t2678,t2680,t2681,t2682,t2684,t2685,t2686,t2688,t2692,t2693,t2694,t2695,t2699,t270,t2702,t2703,t2705,t2706,t2707,t2708,t2719,t2720,t2721,t2722,t2723,t2724,t2725,t2726,t273,t2733,t2734,t2739,t274,t2741,t2742,t2743,t2744,t2748,t2749,t275,t2752,t2759,t276,t2760,t2761,t2762,t2764,t2768,t2769,t277,t2770,t2771,t2773,t2774,t2775,t2776,t278,t2781,t2782,t2783,t2784,t2786,t2787,t2788,t2789,t2791,t2792,t280,t2806,t2808,t2815,t2820,t2821,t2829,t2830,t2831,t284,t2840,t2842,t2844,t2845,t2847,t2848,t2849,t2853,t2854,t2861,t2862,t2863,t2864,t2866,t2868,t2869,t287,t2879,t2884,t2886,t2888,t2892,t2898,t2899,t29,t290,t2900,t2901,t2902,t2903,t2908,t291,t292,t2920,t2923,t2925,t2926,t2928,t2929,t2930,t2937,t294,t2940,t2943,t2945,t2948,t2949,t2950,t2951,t2952,t2960,t2961,t2962,t2963,t2964,t2966,t2967,t2968,t2969,t297,t2970,t2971,t2975,t2976,t2980,t2982,t2983,t2984,t2985,t2986,t2988,t2989,t299,t2991,t2992,t2993,t2996,t2997,t3,t30,t300,t3003,t3004,t3007,t3010,t3011,t3013,t3014,t3019,t302,t3020,t3021,t3023,t3024,t3025,t3027,t3028,t3029,t303,t3030,t3031,t3032,t3033,t3034,t3035,t3036,t3038,t3039,t304,t3043,t3045,t3046,t3047,t305,t3051,t3052,t3053,t3055,t3056,t3057,t306,t3060,t3061,t3062,t3063,t3065,t3066,t3069,t3070,t3071,t3072,t3073,t3075,t3077,t3078,t3079,t3080,t3082,t3083,t3085,t3087,t309,t3090,t3091,t3092,t3093,t3094,t3095,t3098,t3099,t310,t3103,t3104,t3105,t3108,t3109,t311,t3112,t3113,t3119,t3120,t3123,t3124,t3126,t3127,t313,t3130,t3131,t3132,t3133,t3139,t314,t3140,t3142,t3143,t3145,t3146,t3148,t3149,t315,t3150,t3151,t3152,t3156,t3157,t3158,t316,t3160,t3163,t3165,t3167,t3170,t3171,t3172,t3173,t3174,t3177,t3178,t318,t3180,t3182,t3183,t3184,t3186,t3187,t319,t3190,t3191,t3194,t3197,t3199,t320,t3206,t3207,t3208,t3219,t322,t3228,t3230,t3234,t3236,t324,t3240,t3241,t3242,t3243,t3245,t325,t3250,t3251,t3252,t3253,t3254,t3256,t3257,t3260,t3265,t3272,t3273,t3274,t3275,t3276,t3277,t3278,t3279,t328,t3280,t3282,t3283,t3284,t3285,t3286,t3287,t3288,t3289,t3290,t3291,t3292,t3293,t3295,t3296,t3297,t3298,t3299,t3301,t3302,t3303,t3304,t3306,t3307,t3308,t3309,t3310,t3312,t3313,t3314,t3315,t3317,t3318,t3320,t3321,t3324,t3325,t3326,t3327,t3328,t3329,t333,t3331,t3333,t3334,t3335,t3338,t3339,t3342,t3343,t3346,t3347,t3350,t336,t3362,t3363,t3364,t3365,t3366,t3367,t3368,t3369,t337,t3371,t3372,t3373,t3374,t3375,t3376,t3377,t3378,t3380,t3381,t3382,t3383,t3384,t3387,t3390,t3391,t3392,t3393,t3394,t3395,t3396,t3397,t3398,t3399,t34,t340,t3400,t3402,t3403,t3404,t3405,t3406,t3407,t3408,t3409,t3410,t3411,t3412,t3413,t3416,t3417,t3418,t3420,t3421,t3422,t3423,t3424,t3425,t3426,t3427,t3430,t3431,t3432,t3433,t3434,t3435,t3436,t3437,t3439,t344,t3440,t3441,t3442,t3443,t3444,t3445,t3446,t3447,t3449,t3450,t3453,t3454,t3455,t3456,t3457,t3458,t346,t3462,t3463,t3464,t3465,t3466,t3467,t3468,t3469,t347,t3470,t3471,t3472,t3473,t3474,t3475,t3476,t3479,t348,t3480,t3481,t3483,t3485,t3487,t3488,t3489,t349,t3490,t3491,t3492,t3493,t3494,t3496,t3497,t3498,t3499,t350,t3500,t3501,t3502,t3503,t3504,t3505,t3506,t3507,t3509,t3510,t3511,t3513,t3514,t3515,t3516,t3517,t3518,t352,t3521,t3522,t3523,t3527,t3528,t3529,t353,t3530,t3531,t3532,t3533,t3535,t3536,t3538,t3539,t3542,t3543,t3544,t3545,t3546,t3547,t3549,t3550,t3551,t3552,t3554,t3556,t3557,t3559,t356,t3560,t3562,t3563,t3564,t3567,t3568,t3569,t357,t3571,t3572,t3573,t3574,t3577,t3578,t358,t3582,t3583,t3584,t3585,t3586,t3587,t3589,t359,t3590,t3592,t3593,t3596,t3597,t3599,t3602,t3603,t3604,t3605,t3606,t3607,t3608,t3609,t361,t3610,t3611,t3612,t3614,t3615,t3616,t3617,t3618,t3619,t362,t3620,t3625,t3630,t3631,t3633,t3634,t3635,t3636,t3637,t3638,t3642,t3644,t3648,t365,t3652,t3653,t3654,t3655,t3656,t3657,t3658,t3659,t3660,t3662,t3663,t3666,t3667,t3668,t3676,t368,t3681,t3682,t3687,t3688,t369,t3690,t3691,t3693,t3694,t3695,t3696,t3697,t3699,t3700,t3701,t3702,t3704,t3705,t3706,t3707,t3708,t3709,t371,t3713,t3715,t3716,t3717,t372,t3720,t3721,t3723,t3724,t3725,t3726,t3728,t3729,t373,t3730,t3732,t3733,t3734,t3735,t3736,t3737,t3738,t374,t3743,t3744,t3745,t3746,t3747,t3750,t3752,t3756,t3757,t3758,t3766,t3768,t3769,t377,t3774,t3776,t3778,t378,t3780,t3783,t3784,t3785,t3786,t3787,t3789,t379,t3792,t3795,t3798,t380,t3800,t3803,t3804,t3805,t3806,t3810,t3811,t3813,t3814,t3815,t3816,t3817,t3819,t382,t3820,t3821,t3822,t3823,t3824,t3825,t3826,t3827,t3831,t3834,t3835,t3839,t384,t3843,t3849,t3850,t3851,t3852,t3853,t3855,t3857,t3858,t386,t3866,t3867,t3869,t387,t3870,t3877,t388,t3885,t3889,t3890,t3891,t3892,t3899,t391,t3912,t3913,t3915,t3917,t392,t3929,t3930,t3941,t3946,t3949,t395,t3950,t3951,t3952,t3953,t3958,t3959,t396,t3966,t3970,t3980,t3981,t3982,t3984,t3990,t4,t400,t4004,t4005,t4006,t401,t4010,t4011,t4014,t4015,t4016,t4017,t4018,t4019,t402,t4020,t4021,t4022,t4023,t4024,t4025,t4026,t4027,t4028,t4029,t403,t4036,t4039,t4040,t4041,t4042,t4045,t4046,t4047,t4048,t4051,t4053,t4054,t406,t4062,t4063,t4064,t4065,t4068,t4069,t4070,t4071,t4073,t4074,t4075,t4089,t4099,t410,t4103,t4105,t411,t4113,t4114,t4116,t4118,t4119,t412,t4123,t4124,t4125,t413,t4132,t414,t4140,t4142,t4143,t4144,t4145,t415,t4150,t4152,t4153,t416,t4162,t4164,t4165,t4166,t4169,t417,t4171,t4173,t4174,t4177,t4178,t4179,t418,t4180,t4181,t4183,t4184,t4185,t4186,t4188,t4190,t4195,t4196,t4197,t420,t4201,t4202,t4205,t4206,t4207,t4208,t4209,t4210,t4211,t4215,t4217,t4218,t4219,t422,t4220,t4221,t4223,t4224,t4225,t4226,t4228,t4229,t423,t4230,t4231,t4232,t4233,t4234,t4235,t424,t4241,t4242,t4243,t4244,t4245,t4246,t4247,t4248,t4249,t425,t4250,t4251,t4253,t4254,t4255,t4256,t4257,t4258,t4259,t4260,t4261,t4262,t4263,t427,t4273,t4274,t4275,t4276,t4278,t4279,t428,t4280,t4281,t4282,t4283,t4284,t4285,t4286,t4287,t4289,t429,t4290,t4291,t4292,t4293,t4295,t4296,t4297,t4298,t4299,t4300,t4301,t4302,t4303,t4304,t4305,t4306,t4308,t431,t4310,t4315,t4316,t4317,t4318,t432,t4321,t4323,t4324,t4325,t4326,t4327,t4328,t4329,t433,t4330,t4331,t4332,t4333,t4334,t4335,t4336,t4337,t4338,t4339,t434,t4340,t4342,t4344,t4345,t4346,t4347,t4348,t4349,t435,t4350,t4354,t4356,t4357,t436,t4362,t4363,t4365,t4366,t4368,t4369,t437,t4370,t4371,t4372,t4373,t4374,t4375,t4376,t4377,t4379,t438,t4380,t4382,t4383,t4384,t4385,t4386,t4387,t4388,t4389,t439,t4391,t4392,t4394,t4395,t4396,t4397,t4398,t4399,t44,t440,t4400,t4401,t4402,t4403,t4404,t4405,t4406,t4407,t4408,t4409,t441,t4410,t4411,t4412,t4413,t4414,t4415,t4416,t4417,t4418,t4419,t442,t4420,t4421,t4422,t4423,t4424,t4425,t4426,t4427,t4428,t4429,t4430,t4431,t4432,t4433,t4434,t4435,t4436,t4437,t4438,t4439,t444,t4440,t4442,t4444,t4445,t4446,t4447,t4448,t4449,t445,t4450,t4451,t4453,t4454,t4455,t4460,t4461,t4462,t4463,t4464,t4465,t4466,t4467,t4468,t4469,t4470,t4471,t4473,t4474,t4475,t4476,t4477,t4478,t4479,t448,t4481,t4482,t4483,t4484,t4485,t4486,t4487,t4488,t4489,t449,t4490,t4493,t4494,t4495,t4496,t4497,t4498,t4499,t45,t450,t4500,t4501,t4502,t4503,t4504,t4505,t4506,t4507,t4508,t4509,t4510,t4512,t4513,t4514,t4515,t4516,t4518,t4519,t452,t4520,t4521,t4522,t4523,t4524,t4525,t4526,t4527,t4529,t453,t4530,t4531,t4532,t4534,t4535,t4537,t4538,t4539,t454,t4541,t4543,t4544,t4545,t4546,t4547,t4549,t4550,t4551,t4552,t4553,t4554,t4556,t4557,t4558,t4559,t4560,t4564,t4565,t4566,t4567,t4568,t4569,t457,t4570,t4572,t4573,t4575,t4576,t4577,t4578,t458,t4580,t4581,t4582,t4584,t4586,t4587,t4588,t4589,t459,t4590,t4591,t4592,t4593,t4594,t4595,t4596,t4597,t4598,t4599,t46,t460,t4600,t4601,t4602,t4603,t4604,t4605,t4606,t4607,t4608,t4609,t461,t4610,t4612,t4613,t4614,t4615,t4616,t4617,t4618,t4619,t462,t4620,t4621,t4622,t4623,t4624,t4625,t4626,t4627,t4629,t463,t4631,t4632,t4633,t4634,t4635,t4636,t4637,t4638,t4639,t464,t4640,t4643,t4644,t4645,t4646,t4647,t4649,t465,t4650,t4652,t4653,t4654,t4655,t4656,t4657,t4659,t466,t4660,t4661,t4662,t4663,t4664,t4665,t4666,t4667,t4668,t4669,t4670,t4671,t4672,t4673,t4674,t4675,t4676,t4677,t4678,t4679,t468,t4680,t4681,t4682,t4683,t4684,t4685,t4686,t4687,t4689,t469,t4692,t4693,t4694,t4695,t4696,t4697,t4698,t4699,t47,t470,t4700,t4702,t4703,t4704,t4707,t4708,t4709,t471,t4710,t4711,t4712,t4713,t4714,t4715,t4716,t4717,t4718,t4719,t472,t4720,t4721,t4722,t4723,t4724,t4725,t4726,t4727,t4728,t4729,t4730,t4731,t4732,t4733,t4734,t4736,t4737,t4738,t4739,t4740,t4742,t4745,t4746,t4747,t4748,t475,t4750,t4751,t4753,t4754,t4755,t4756,t4757,t4762,t4763,t4765,t4768,t477,t4771,t4772,t4773,t4774,t4775,t4776,t4779,t4780,t4781,t4782,t4783,t4784,t4785,t4786,t4787,t4788,t4789,t479,t4790,t4791,t4792,t4793,t4794,t4795,t4797,t4799,t480,t4800,t4801,t4802,t4803,t4805,t4806,t4809,t481,t4810,t4811,t4812,t4813,t4814,t4818,t4819,t482,t4820,t4821,t4824,t4825,t4826,t4827,t4829,t483,t4831,t4833,t4834,t4835,t4837,t484,t4840,t4841,t4842,t4845,t4846,t4847,t4848,t485,t4851,t4853,t4856,t4857,t486,t4862,t4863,t4864,t4865,t4866,t4867,t4868,t4869,t4870,t4872,t4873,t4874,t4875,t4876,t4877,t488,t4880,t4884,t4888,t489,t4893,t4895,t4903,t4904,t4907,t4908,t491,t4911,t4913,t4914,t4919,t492,t4920,t4922,t4924,t4925,t4927,t4928,t4929,t493,t4931,t4933,t4934,t4935,t4936,t494,t4942,t4943,t4944,t4946,t4948,t4949,t4950,t4951,t4952,t4953,t4957,t496,t4963,t4964,t4969,t497,t4970,t4973,t4974,t4975,t4976,t4978,t4979,t498,t4981,t4982,t4983,t4987,t4988,t4989,t499,t4990,t4991,t4992,t4993,t4994,t4995,t4996,t5,t50,t500,t5000,t5001,t5002,t5003,t5005,t5006,t5007,t5008,t5009,t501,t5010,t5014,t5015,t5016,t5017,t5018,t5019,t502,t5020,t5021,t5022,t5023,t5024,t5026,t5027,t5029,t503,t5030,t5031,t5032,t5035,t5036,t5039,t504,t5041,t5045,t5048,t505,t5051,t5054,t5055,t5056,t5058,t5059,t506,t5061,t5063,t5064,t5065,t5066,t5067,t507,t5073,t5074,t5075,t5076,t5077,t5078,t508,t5080,t5081,t5083,t5084,t5085,t5088,t5089,t509,t5090,t5091,t5093,t5095,t5097,t5098,t5099,t510,t5100,t5101,t5102,t5107,t5109,t511,t5110,t5112,t5113,t5114,t5119,t512,t5120,t5121,t5123,t5125,t513,t5131,t5132,t5136,t5138,t5139,t514,t5140,t5143,t5146,t5147,t5148,t5150,t5151,t5152,t5153,t5154,t5157,t5158,t516,t5164,t5166,t517,t5171,t5172,t5174,t5175,t518,t5180,t5181,t5183,t5184,t5185,t5187,t5189,t5191,t5195,t5199,t520,t5200,t5201,t5202,t5203,t5204,t5205,t5206,t5207,t5209,t521,t5210,t5211,t5215,t5216,t5217,t5218,t5219,t522,t5222,t5223,t5224,t5227,t5229,t523,t5233,t5236,t5237,t5238,t5239,t524,t5240,t5242,t5244,t5247,t5248,t5249,t525,t5251,t5252,t5255,t5257,t5258,t526,t5261,t5262,t5265,t5268,t5269,t527,t5270,t5272,t5279,t528,t5280,t5285,t5288,t529,t5292,t5293,t5294,t5295,t5297,t53,t530,t5302,t5306,t531,t5318,t532,t5320,t5321,t5324,t5327,t533,t5331,t5332,t5339,t534,t5344,t5346,t5347,t5348,t5349,t535,t5351,t5355,t5356,t5358,t536,t5361,t5364,t5365,t5367,t5368,t537,t5372,t5373,t5375,t5378,t538,t5383,t5387,t5389,t539,t5390,t5391,t5392,t5393,t5394,t5395,t540,t5402,t5404,t5409,t5416,t5420,t543,t5433,t5435,t5436,t544,t5440,t5441,t5442,t5443,t5444,t5445,t5446,t5448,t545,t5450,t5451,t5453,t5454,t5457,t5459,t546,t5463,t5464,t5465,t5466,t547,t5473,t5475,t5479,t548,t5480,t5481,t5482,t5483,t5484,t5485,t5486,t5487,t5488,t5489,t549,t5490,t5491,t5492,t5493,t5494,t5496,t5498,t5499,t5501,t5507,t551,t5512,t5516,t5517,t5519,t552,t5521,t5522,t5526,t5527,t553,t5534,t554,t5540,t5546,t5549,t555,t5552,t5555,t5559,t556,t5561,t5562,t5563,t5565,t5566,t5569,t557,t5573,t5578,t558,t5580,t5581,t5583,t5584,t5589,t559,t5590,t5593,t5594,t5596,t5597,t560,t5600,t5603,t5604,t5606,t5607,t561,t5611,t5612,t5618,t562,t5629,t563,t5633,t5634,t5635,t564,t5656,t5660,t5667,t5668,t567,t5673,t5678,t568,t5688,t569,t57,t570,t571,t572,t573,t574,t5741,t5743,t576,t577,t5777,t5779,t578,t5780,t5782,t579,t58,t580,t581,t5818,t5819,t582,t5823,t5826,t583,t584,t586,t587,t5886,t5887,t589,t5894,t59,t590,t591,t592,t593,t594,t595,t596,t597,t6,t60,t600,t602,t603,t604,t605,t609,t610,t611,t612,t613,t614,t615,t616,t618,t619,t620,t621,t622,t623,t624,t625,t626,t627,t628,t629,t63,t630,t631,t632,t633,t634,t635,t636,t637,t638,t639,t640,t641,t642,t643,t645,t646,t647,t648,t649,t650,t653,t654,t655,t656,t657,t658,t660,t662,t663,t664,t665,t667,t668,t669,t673,t674,t675,t676,t679,t680,t681,t682,t683,t684,t685,t686,t687,t688,t689,t691,t692,t693,t694,t695,t696,t697,t698,t7,t700,t702,t703,t704,t705,t706,t708,t71,t710,t711,t712,t713,t7148,t715,t716,t72,t724,t728,t73,t731,t733,t734,t735,t736,t738,t739,t74,t740,t741,t742,t743,t744,t746,t747,t748,t749,t75,t750,t751,t752,t753,t754,t755,t756,t757,t758,t759,t76,t760,t762,t763,t764,t765,t766,t767,t768,t769,t77,t772,t773,t774,t775,t776,t777,t778,t779,t780,t781,t782,t784,t785,t786,t792,t794,t795,t796,t797,t798,t799,t8,t80,t801,t802,t804,t805,t806,t808,t81,t814,t815,t817,t82,t820,t822,t823,t824,t825,t826,t827,t829,t83,t830,t831,t832,t833,t834,t835,t836,t837,t838,t84,t840,t841,t842,t843,t844,t845,t846,t847,t852,t853,t856,t858,t859,t86,t861,t863,t865,t866,t867,t868,t869,t870,t874,t875,t876,t877,t878,t880,t881,t882,t884,t885,t888,t891,t895,t899,t9,t90,t900,t902,t903,t906,t909,t91,t910,t911,t914,t916,t917,t920,t921,t922,t923,t925,t926,t927,t928,t929,t930,t934,t935,t937,t940,t941,t942,t943,t944,t945,t946,t947,t949,t95,t950,t951,t952,t953,t954,t955,t957,t958,t961,t962,t963,t964,t965,t968,t97,t970,t971,t972,t973,t974,t975,t976,t977,t982,t983,t984,t986,t987,t988,t989,t99,t991,t993,t994,t995,t999});
end
function C_dq = ft_9(ct)
dq1 = ct{1};
dq2 = ct{2};
dq3 = ct{3};
dq4 = ct{4};
dq5 = ct{5};
dq6 = ct{6};
t1004 = ct{7};
t1006 = ct{8};
t1008 = ct{9};
t101 = ct{10};
t1013 = ct{11};
t1016 = ct{12};
t1017 = ct{13};
t1019 = ct{14};
t102 = ct{15};
t1020 = ct{16};
t1021 = ct{17};
t1023 = ct{18};
t1024 = ct{19};
t1025 = ct{20};
t1026 = ct{21};
t1028 = ct{22};
t1030 = ct{23};
t1032 = ct{24};
t1034 = ct{25};
t1036 = ct{26};
t1038 = ct{27};
t1039 = ct{28};
t1040 = ct{29};
t1042 = ct{30};
t1043 = ct{31};
t1044 = ct{32};
t1045 = ct{33};
t1046 = ct{34};
t1047 = ct{35};
t1048 = ct{36};
t1049 = ct{37};
t1050 = ct{38};
t1051 = ct{39};
t1054 = ct{40};
t1055 = ct{41};
t1056 = ct{42};
t1057 = ct{43};
t1059 = ct{44};
t1061 = ct{45};
t1065 = ct{46};
t1066 = ct{47};
t1068 = ct{48};
t1069 = ct{49};
t1070 = ct{50};
t1072 = ct{51};
t1073 = ct{52};
t1075 = ct{53};
t1076 = ct{54};
t1077 = ct{55};
t1081 = ct{56};
t1083 = ct{57};
t1084 = ct{58};
t1085 = ct{59};
t1087 = ct{60};
t1089 = ct{61};
t1091 = ct{62};
t1092 = ct{63};
t1093 = ct{64};
t1095 = ct{65};
t1098 = ct{66};
t1099 = ct{67};
t110 = ct{68};
t1101 = ct{69};
t1102 = ct{70};
t1105 = ct{71};
t1106 = ct{72};
t1107 = ct{73};
t1108 = ct{74};
t1109 = ct{75};
t111 = ct{76};
t1113 = ct{77};
t1115 = ct{78};
t1116 = ct{79};
t1119 = ct{80};
t112 = ct{81};
t1122 = ct{82};
t1125 = ct{83};
t1126 = ct{84};
t1127 = ct{85};
t1128 = ct{86};
t113 = ct{87};
t1130 = ct{88};
t1131 = ct{89};
t1133 = ct{90};
t1134 = ct{91};
t1135 = ct{92};
t1138 = ct{93};
t1139 = ct{94};
t114 = ct{95};
t1141 = ct{96};
t1144 = ct{97};
t1145 = ct{98};
t1146 = ct{99};
t1147 = ct{100};
t1148 = ct{101};
t1149 = ct{102};
t115 = ct{103};
t1150 = ct{104};
t1152 = ct{105};
t1153 = ct{106};
t1155 = ct{107};
t1158 = ct{108};
t1159 = ct{109};
t116 = ct{110};
t1162 = ct{111};
t1163 = ct{112};
t1165 = ct{113};
t1167 = ct{114};
t1169 = ct{115};
t1170 = ct{116};
t1171 = ct{117};
t1173 = ct{118};
t1174 = ct{119};
t1175 = ct{120};
t1177 = ct{121};
t1178 = ct{122};
t1179 = ct{123};
t1180 = ct{124};
t1181 = ct{125};
t1182 = ct{126};
t1183 = ct{127};
t1184 = ct{128};
t1185 = ct{129};
t1186 = ct{130};
t1188 = ct{131};
t1189 = ct{132};
t1190 = ct{133};
t1191 = ct{134};
t1192 = ct{135};
t1193 = ct{136};
t1194 = ct{137};
t1196 = ct{138};
t1197 = ct{139};
t1198 = ct{140};
t1199 = ct{141};
t120 = ct{142};
t1200 = ct{143};
t1202 = ct{144};
t1203 = ct{145};
t1204 = ct{146};
t1205 = ct{147};
t1206 = ct{148};
t1207 = ct{149};
t121 = ct{150};
t1210 = ct{151};
t1211 = ct{152};
t1215 = ct{153};
t1219 = ct{154};
t1221 = ct{155};
t1222 = ct{156};
t1224 = ct{157};
t1225 = ct{158};
t1227 = ct{159};
t1228 = ct{160};
t1233 = ct{161};
t1235 = ct{162};
t1236 = ct{163};
t1237 = ct{164};
t1239 = ct{165};
t124 = ct{166};
t1240 = ct{167};
t1241 = ct{168};
t1244 = ct{169};
t1245 = ct{170};
t125 = ct{171};
t1250 = ct{172};
t1251 = ct{173};
t1253 = ct{174};
t1254 = ct{175};
t1256 = ct{176};
t1257 = ct{177};
t1258 = ct{178};
t1259 = ct{179};
t126 = ct{180};
t1261 = ct{181};
t1262 = ct{182};
t1263 = ct{183};
t1264 = ct{184};
t1265 = ct{185};
t1266 = ct{186};
t1267 = ct{187};
t1268 = ct{188};
t1269 = ct{189};
t1271 = ct{190};
t1272 = ct{191};
t1273 = ct{192};
t1274 = ct{193};
t1277 = ct{194};
t1278 = ct{195};
t128 = ct{196};
t1280 = ct{197};
t1282 = ct{198};
t1285 = ct{199};
t1286 = ct{200};
t1288 = ct{201};
t129 = ct{202};
t1290 = ct{203};
t1293 = ct{204};
t1294 = ct{205};
t1295 = ct{206};
t1296 = ct{207};
t1298 = ct{208};
t1300 = ct{209};
t1301 = ct{210};
t1302 = ct{211};
t1306 = ct{212};
t1307 = ct{213};
t1308 = ct{214};
t1309 = ct{215};
t131 = ct{216};
t1311 = ct{217};
t1312 = ct{218};
t1313 = ct{219};
t1315 = ct{220};
t1316 = ct{221};
t1317 = ct{222};
t1318 = ct{223};
t1319 = ct{224};
t132 = ct{225};
t1322 = ct{226};
t1323 = ct{227};
t1324 = ct{228};
t1325 = ct{229};
t1326 = ct{230};
t1328 = ct{231};
t1329 = ct{232};
t133 = ct{233};
t1330 = ct{234};
t1331 = ct{235};
t1333 = ct{236};
t1334 = ct{237};
t1337 = ct{238};
t1338 = ct{239};
t1340 = ct{240};
t1341 = ct{241};
t1342 = ct{242};
t1343 = ct{243};
t1344 = ct{244};
t1345 = ct{245};
t1346 = ct{246};
t1348 = ct{247};
t1351 = ct{248};
t1352 = ct{249};
t1353 = ct{250};
t1354 = ct{251};
t1355 = ct{252};
t1356 = ct{253};
t1360 = ct{254};
t1362 = ct{255};
t1365 = ct{256};
t1366 = ct{257};
t1367 = ct{258};
t1369 = ct{259};
t1370 = ct{260};
t1371 = ct{261};
t1372 = ct{262};
t1374 = ct{263};
t1375 = ct{264};
t1377 = ct{265};
t1378 = ct{266};
t1379 = ct{267};
t1380 = ct{268};
t1383 = ct{269};
t1384 = ct{270};
t1385 = ct{271};
t1386 = ct{272};
t1388 = ct{273};
t1389 = ct{274};
t139 = ct{275};
t1391 = ct{276};
t1392 = ct{277};
t1393 = ct{278};
t1394 = ct{279};
t1397 = ct{280};
t1398 = ct{281};
t140 = ct{282};
t1401 = ct{283};
t1402 = ct{284};
t1403 = ct{285};
t1404 = ct{286};
t1406 = ct{287};
t1407 = ct{288};
t1408 = ct{289};
t1409 = ct{290};
t141 = ct{291};
t1410 = ct{292};
t1411 = ct{293};
t1413 = ct{294};
t1414 = ct{295};
t1415 = ct{296};
t1416 = ct{297};
t1417 = ct{298};
t1419 = ct{299};
t142 = ct{300};
t1422 = ct{301};
t1423 = ct{302};
t1426 = ct{303};
t1427 = ct{304};
t1428 = ct{305};
t1429 = ct{306};
t1430 = ct{307};
t1431 = ct{308};
t1432 = ct{309};
t1433 = ct{310};
t1436 = ct{311};
t144 = ct{312};
t1440 = ct{313};
t1441 = ct{314};
t1442 = ct{315};
t1443 = ct{316};
t1445 = ct{317};
t1446 = ct{318};
t1447 = ct{319};
t1448 = ct{320};
t1449 = ct{321};
t1451 = ct{322};
t1452 = ct{323};
t1453 = ct{324};
t1454 = ct{325};
t1455 = ct{326};
t1456 = ct{327};
t1457 = ct{328};
t1458 = ct{329};
t1459 = ct{330};
t1460 = ct{331};
t1463 = ct{332};
t1464 = ct{333};
t1465 = ct{334};
t1467 = ct{335};
t1470 = ct{336};
t1471 = ct{337};
t1474 = ct{338};
t1476 = ct{339};
t1478 = ct{340};
t1479 = ct{341};
t148 = ct{342};
t1480 = ct{343};
t1481 = ct{344};
t1482 = ct{345};
t1483 = ct{346};
t1486 = ct{347};
t1487 = ct{348};
t1488 = ct{349};
t1489 = ct{350};
t1490 = ct{351};
t1491 = ct{352};
t1492 = ct{353};
t1493 = ct{354};
t1494 = ct{355};
t1495 = ct{356};
t1496 = ct{357};
t1498 = ct{358};
t1499 = ct{359};
t15 = ct{360};
t150 = ct{361};
t1500 = ct{362};
t1501 = ct{363};
t1503 = ct{364};
t1505 = ct{365};
t1506 = ct{366};
t1507 = ct{367};
t1508 = ct{368};
t1509 = ct{369};
t151 = ct{370};
t1510 = ct{371};
t1511 = ct{372};
t1512 = ct{373};
t1513 = ct{374};
t1515 = ct{375};
t1517 = ct{376};
t1520 = ct{377};
t1521 = ct{378};
t1522 = ct{379};
t1523 = ct{380};
t1524 = ct{381};
t1526 = ct{382};
t1527 = ct{383};
t1529 = ct{384};
t153 = ct{385};
t1530 = ct{386};
t1531 = ct{387};
t1532 = ct{388};
t1533 = ct{389};
t1534 = ct{390};
t1535 = ct{391};
t1536 = ct{392};
t1537 = ct{393};
t1538 = ct{394};
t1539 = ct{395};
t154 = ct{396};
t1540 = ct{397};
t1541 = ct{398};
t1542 = ct{399};
t1548 = ct{400};
t1549 = ct{401};
t1550 = ct{402};
t1551 = ct{403};
t1553 = ct{404};
t1557 = ct{405};
t1558 = ct{406};
t156 = ct{407};
t1560 = ct{408};
t1561 = ct{409};
t1562 = ct{410};
t1564 = ct{411};
t1566 = ct{412};
t1567 = ct{413};
t1568 = ct{414};
t157 = ct{415};
t1570 = ct{416};
t1571 = ct{417};
t1572 = ct{418};
t1574 = ct{419};
t1575 = ct{420};
t1576 = ct{421};
t1577 = ct{422};
t1578 = ct{423};
t1579 = ct{424};
t158 = ct{425};
t1580 = ct{426};
t1581 = ct{427};
t1582 = ct{428};
t1583 = ct{429};
t1584 = ct{430};
t1585 = ct{431};
t1586 = ct{432};
t1587 = ct{433};
t1589 = ct{434};
t1590 = ct{435};
t1591 = ct{436};
t1592 = ct{437};
t1593 = ct{438};
t1594 = ct{439};
t1595 = ct{440};
t1596 = ct{441};
t1597 = ct{442};
t1598 = ct{443};
t1599 = ct{444};
t16 = ct{445};
t1601 = ct{446};
t1602 = ct{447};
t1605 = ct{448};
t1606 = ct{449};
t1607 = ct{450};
t1609 = ct{451};
t161 = ct{452};
t1610 = ct{453};
t1611 = ct{454};
t1612 = ct{455};
t1613 = ct{456};
t1614 = ct{457};
t1615 = ct{458};
t1616 = ct{459};
t1617 = ct{460};
t1618 = ct{461};
t1619 = ct{462};
t1620 = ct{463};
t1621 = ct{464};
t1622 = ct{465};
t1624 = ct{466};
t1625 = ct{467};
t1626 = ct{468};
t1627 = ct{469};
t163 = ct{470};
t1630 = ct{471};
t1631 = ct{472};
t1632 = ct{473};
t1633 = ct{474};
t1635 = ct{475};
t1636 = ct{476};
t1637 = ct{477};
t1638 = ct{478};
t1639 = ct{479};
t1641 = ct{480};
t1642 = ct{481};
t1643 = ct{482};
t1644 = ct{483};
t1645 = ct{484};
t1646 = ct{485};
t1647 = ct{486};
t1648 = ct{487};
t1649 = ct{488};
t165 = ct{489};
t1651 = ct{490};
t1652 = ct{491};
t1653 = ct{492};
t1657 = ct{493};
t1658 = ct{494};
t1659 = ct{495};
t166 = ct{496};
t1660 = ct{497};
t1661 = ct{498};
t1662 = ct{499};
t1663 = ct{500};
t1665 = ct{501};
t1666 = ct{502};
t1667 = ct{503};
t1669 = ct{504};
t1670 = ct{505};
t1671 = ct{506};
t1672 = ct{507};
t1673 = ct{508};
t1674 = ct{509};
t1675 = ct{510};
t1676 = ct{511};
t1681 = ct{512};
t1682 = ct{513};
t1683 = ct{514};
t1686 = ct{515};
t1687 = ct{516};
t1689 = ct{517};
t1691 = ct{518};
t1692 = ct{519};
t1696 = ct{520};
t1697 = ct{521};
t1698 = ct{522};
t1699 = ct{523};
t17 = ct{524};
t170 = ct{525};
t1700 = ct{526};
t1701 = ct{527};
t1702 = ct{528};
t1703 = ct{529};
t1704 = ct{530};
t1705 = ct{531};
t1706 = ct{532};
t1709 = ct{533};
t171 = ct{534};
t1710 = ct{535};
t1711 = ct{536};
t1712 = ct{537};
t1713 = ct{538};
t1715 = ct{539};
t1716 = ct{540};
t1718 = ct{541};
t1719 = ct{542};
t1720 = ct{543};
t1721 = ct{544};
t1722 = ct{545};
t1724 = ct{546};
t1726 = ct{547};
t1728 = ct{548};
t1729 = ct{549};
t1731 = ct{550};
t1733 = ct{551};
t1734 = ct{552};
t1735 = ct{553};
t1736 = ct{554};
t1737 = ct{555};
t1738 = ct{556};
t1739 = ct{557};
t1740 = ct{558};
t1743 = ct{559};
t1745 = ct{560};
t1746 = ct{561};
t1748 = ct{562};
t1749 = ct{563};
t1752 = ct{564};
t1755 = ct{565};
t1756 = ct{566};
t1757 = ct{567};
t1758 = ct{568};
t1759 = ct{569};
t1760 = ct{570};
t1761 = ct{571};
t1763 = ct{572};
t1764 = ct{573};
t1767 = ct{574};
t1769 = ct{575};
t177 = ct{576};
t1770 = ct{577};
t1771 = ct{578};
t1772 = ct{579};
t1773 = ct{580};
t1774 = ct{581};
t1775 = ct{582};
t1776 = ct{583};
t1779 = ct{584};
t1780 = ct{585};
t1782 = ct{586};
t1783 = ct{587};
t1784 = ct{588};
t1785 = ct{589};
t1786 = ct{590};
t1787 = ct{591};
t1788 = ct{592};
t1789 = ct{593};
t1791 = ct{594};
t1792 = ct{595};
t1793 = ct{596};
t1795 = ct{597};
t1797 = ct{598};
t1798 = ct{599};
t1799 = ct{600};
t18 = ct{601};
t1800 = ct{602};
t1801 = ct{603};
t1802 = ct{604};
t1804 = ct{605};
t1806 = ct{606};
t1807 = ct{607};
t1808 = ct{608};
t1809 = ct{609};
t1810 = ct{610};
t1811 = ct{611};
t1812 = ct{612};
t1813 = ct{613};
t1814 = ct{614};
t1816 = ct{615};
t1817 = ct{616};
t1820 = ct{617};
t1822 = ct{618};
t1823 = ct{619};
t1824 = ct{620};
t1825 = ct{621};
t1827 = ct{622};
t1828 = ct{623};
t1829 = ct{624};
t183 = ct{625};
t1830 = ct{626};
t1831 = ct{627};
t1832 = ct{628};
t1833 = ct{629};
t1834 = ct{630};
t1835 = ct{631};
t1836 = ct{632};
t1837 = ct{633};
t1838 = ct{634};
t1839 = ct{635};
t1844 = ct{636};
t1847 = ct{637};
t1849 = ct{638};
t185 = ct{639};
t1850 = ct{640};
t1851 = ct{641};
t1854 = ct{642};
t1855 = ct{643};
t1857 = ct{644};
t1858 = ct{645};
t1859 = ct{646};
t1862 = ct{647};
t1864 = ct{648};
t1865 = ct{649};
t1866 = ct{650};
t1867 = ct{651};
t1871 = ct{652};
t1873 = ct{653};
t1877 = ct{654};
t1879 = ct{655};
t1880 = ct{656};
t1881 = ct{657};
t1882 = ct{658};
t1884 = ct{659};
t1887 = ct{660};
t1889 = ct{661};
t1892 = ct{662};
t1893 = ct{663};
t1896 = ct{664};
t19 = ct{665};
t190 = ct{666};
t1903 = ct{667};
t1904 = ct{668};
t1906 = ct{669};
t1907 = ct{670};
t1908 = ct{671};
t1909 = ct{672};
t191 = ct{673};
t1910 = ct{674};
t1911 = ct{675};
t1912 = ct{676};
t1913 = ct{677};
t1914 = ct{678};
t1915 = ct{679};
t1916 = ct{680};
t1919 = ct{681};
t1920 = ct{682};
t1921 = ct{683};
t1925 = ct{684};
t1926 = ct{685};
t1930 = ct{686};
t1935 = ct{687};
t1936 = ct{688};
t1937 = ct{689};
t1938 = ct{690};
t1939 = ct{691};
t1943 = ct{692};
t1944 = ct{693};
t1946 = ct{694};
t1950 = ct{695};
t1955 = ct{696};
t196 = ct{697};
t1961 = ct{698};
t1966 = ct{699};
t1967 = ct{700};
t1968 = ct{701};
t1969 = ct{702};
t197 = ct{703};
t1970 = ct{704};
t1971 = ct{705};
t1973 = ct{706};
t1976 = ct{707};
t1977 = ct{708};
t1978 = ct{709};
t1979 = ct{710};
t1980 = ct{711};
t1981 = ct{712};
t1984 = ct{713};
t1988 = ct{714};
t199 = ct{715};
t1992 = ct{716};
t1993 = ct{717};
t1994 = ct{718};
t1995 = ct{719};
t1996 = ct{720};
t1997 = ct{721};
t1998 = ct{722};
t1999 = ct{723};
t2 = ct{724};
t20 = ct{725};
t200 = ct{726};
t2000 = ct{727};
t2001 = ct{728};
t2002 = ct{729};
t2003 = ct{730};
t2004 = ct{731};
t2005 = ct{732};
t2006 = ct{733};
t2008 = ct{734};
t201 = ct{735};
t2014 = ct{736};
t2016 = ct{737};
t2017 = ct{738};
t2019 = ct{739};
t202 = ct{740};
t2020 = ct{741};
t2021 = ct{742};
t2023 = ct{743};
t2024 = ct{744};
t2028 = ct{745};
t2029 = ct{746};
t203 = ct{747};
t2033 = ct{748};
t2036 = ct{749};
t2037 = ct{750};
t2038 = ct{751};
t204 = ct{752};
t2040 = ct{753};
t2041 = ct{754};
t2042 = ct{755};
t2044 = ct{756};
t2047 = ct{757};
t205 = ct{758};
t2051 = ct{759};
t2052 = ct{760};
t2053 = ct{761};
t2054 = ct{762};
t2055 = ct{763};
t2056 = ct{764};
t2057 = ct{765};
t2058 = ct{766};
t2059 = ct{767};
t206 = ct{768};
t2060 = ct{769};
t2061 = ct{770};
t2062 = ct{771};
t2065 = ct{772};
t2066 = ct{773};
t2067 = ct{774};
t2068 = ct{775};
t2069 = ct{776};
t207 = ct{777};
t2070 = ct{778};
t2071 = ct{779};
t2072 = ct{780};
t2073 = ct{781};
t2074 = ct{782};
t2076 = ct{783};
t2077 = ct{784};
t2078 = ct{785};
t2079 = ct{786};
t208 = ct{787};
t2080 = ct{788};
t2081 = ct{789};
t2082 = ct{790};
t2083 = ct{791};
t2084 = ct{792};
t2085 = ct{793};
t2086 = ct{794};
t2087 = ct{795};
t2088 = ct{796};
t2089 = ct{797};
t209 = ct{798};
t2091 = ct{799};
t2092 = ct{800};
t2093 = ct{801};
t2094 = ct{802};
t2095 = ct{803};
t2096 = ct{804};
t2097 = ct{805};
t2098 = ct{806};
t2099 = ct{807};
t21 = ct{808};
t210 = ct{809};
t2100 = ct{810};
t2101 = ct{811};
t2104 = ct{812};
t2105 = ct{813};
t2106 = ct{814};
t2107 = ct{815};
t2108 = ct{816};
t2109 = ct{817};
t211 = ct{818};
t2110 = ct{819};
t2111 = ct{820};
t2113 = ct{821};
t2114 = ct{822};
t2115 = ct{823};
t2116 = ct{824};
t2117 = ct{825};
t2118 = ct{826};
t2119 = ct{827};
t212 = ct{828};
t2121 = ct{829};
t2125 = ct{830};
t2128 = ct{831};
t2129 = ct{832};
t213 = ct{833};
t2130 = ct{834};
t2131 = ct{835};
t2132 = ct{836};
t2133 = ct{837};
t2135 = ct{838};
t2136 = ct{839};
t2139 = ct{840};
t2140 = ct{841};
t2141 = ct{842};
t2142 = ct{843};
t2144 = ct{844};
t2147 = ct{845};
t2148 = ct{846};
t2149 = ct{847};
t2150 = ct{848};
t2151 = ct{849};
t2154 = ct{850};
t2155 = ct{851};
t2156 = ct{852};
t2157 = ct{853};
t2158 = ct{854};
t2159 = ct{855};
t2162 = ct{856};
t2163 = ct{857};
t2166 = ct{858};
t2167 = ct{859};
t2168 = ct{860};
t2169 = ct{861};
t2170 = ct{862};
t2171 = ct{863};
t2172 = ct{864};
t2174 = ct{865};
t2175 = ct{866};
t2176 = ct{867};
t2177 = ct{868};
t2178 = ct{869};
t2180 = ct{870};
t2182 = ct{871};
t2184 = ct{872};
t2185 = ct{873};
t2186 = ct{874};
t2187 = ct{875};
t2189 = ct{876};
t2190 = ct{877};
t2191 = ct{878};
t2192 = ct{879};
t2194 = ct{880};
t2195 = ct{881};
t2196 = ct{882};
t22 = ct{883};
t2200 = ct{884};
t2201 = ct{885};
t2203 = ct{886};
t2204 = ct{887};
t2208 = ct{888};
t2209 = ct{889};
t2210 = ct{890};
t2212 = ct{891};
t2214 = ct{892};
t2217 = ct{893};
t2218 = ct{894};
t2219 = ct{895};
t2220 = ct{896};
t2221 = ct{897};
t2223 = ct{898};
t2225 = ct{899};
t2227 = ct{900};
t2228 = ct{901};
t2229 = ct{902};
t2231 = ct{903};
t2232 = ct{904};
t2236 = ct{905};
t2237 = ct{906};
t2239 = ct{907};
t224 = ct{908};
t2240 = ct{909};
t2243 = ct{910};
t2246 = ct{911};
t2249 = ct{912};
t225 = ct{913};
t2250 = ct{914};
t2251 = ct{915};
t2252 = ct{916};
t2254 = ct{917};
t2255 = ct{918};
t2256 = ct{919};
t2257 = ct{920};
t2264 = ct{921};
t2265 = ct{922};
t2266 = ct{923};
t2267 = ct{924};
t2269 = ct{925};
t227 = ct{926};
t2270 = ct{927};
t2271 = ct{928};
t2272 = ct{929};
t2273 = ct{930};
t2274 = ct{931};
t2276 = ct{932};
t2277 = ct{933};
t2278 = ct{934};
t2279 = ct{935};
t228 = ct{936};
t2280 = ct{937};
t2281 = ct{938};
t2282 = ct{939};
t2283 = ct{940};
t2284 = ct{941};
t2285 = ct{942};
t2286 = ct{943};
t2287 = ct{944};
t2291 = ct{945};
t2292 = ct{946};
t2295 = ct{947};
t23 = ct{948};
t230 = ct{949};
t2302 = ct{950};
t2304 = ct{951};
t2305 = ct{952};
t2306 = ct{953};
t2307 = ct{954};
t2308 = ct{955};
t2309 = ct{956};
t231 = ct{957};
t2310 = ct{958};
t2311 = ct{959};
t2312 = ct{960};
t2314 = ct{961};
t2316 = ct{962};
t2317 = ct{963};
t2318 = ct{964};
t2321 = ct{965};
t2322 = ct{966};
t2323 = ct{967};
t2324 = ct{968};
t233 = ct{969};
t2331 = ct{970};
t2333 = ct{971};
t2334 = ct{972};
t2335 = ct{973};
t2336 = ct{974};
t2337 = ct{975};
t2338 = ct{976};
t2339 = ct{977};
t234 = ct{978};
t2340 = ct{979};
t2341 = ct{980};
t2342 = ct{981};
t2344 = ct{982};
t2347 = ct{983};
t2348 = ct{984};
t235 = ct{985};
t2350 = ct{986};
t2351 = ct{987};
t2355 = ct{988};
t2357 = ct{989};
t2358 = ct{990};
t2359 = ct{991};
t236 = ct{992};
t2361 = ct{993};
t2362 = ct{994};
t2363 = ct{995};
t2364 = ct{996};
t2365 = ct{997};
t2366 = ct{998};
t2368 = ct{999};
t2369 = ct{1000};
t2370 = ct{1001};
t2371 = ct{1002};
t2372 = ct{1003};
t2373 = ct{1004};
t2374 = ct{1005};
t2375 = ct{1006};
t2376 = ct{1007};
t2377 = ct{1008};
t2378 = ct{1009};
t2379 = ct{1010};
t2381 = ct{1011};
t2382 = ct{1012};
t2384 = ct{1013};
t2385 = ct{1014};
t2387 = ct{1015};
t2388 = ct{1016};
t2389 = ct{1017};
t2390 = ct{1018};
t2391 = ct{1019};
t2392 = ct{1020};
t2394 = ct{1021};
t2395 = ct{1022};
t2396 = ct{1023};
t2397 = ct{1024};
t24 = ct{1025};
t240 = ct{1026};
t2400 = ct{1027};
t2401 = ct{1028};
t2402 = ct{1029};
t2403 = ct{1030};
t2405 = ct{1031};
t2406 = ct{1032};
t2407 = ct{1033};
t2410 = ct{1034};
t2417 = ct{1035};
t2421 = ct{1036};
t2422 = ct{1037};
t2423 = ct{1038};
t2425 = ct{1039};
t2427 = ct{1040};
t2428 = ct{1041};
t2429 = ct{1042};
t243 = ct{1043};
t2430 = ct{1044};
t2431 = ct{1045};
t2434 = ct{1046};
t2435 = ct{1047};
t2437 = ct{1048};
t2438 = ct{1049};
t2439 = ct{1050};
t244 = ct{1051};
t2440 = ct{1052};
t2441 = ct{1053};
t2443 = ct{1054};
t2444 = ct{1055};
t2445 = ct{1056};
t2446 = ct{1057};
t2449 = ct{1058};
t2452 = ct{1059};
t2453 = ct{1060};
t2454 = ct{1061};
t2455 = ct{1062};
t2456 = ct{1063};
t2457 = ct{1064};
t2458 = ct{1065};
t2459 = ct{1066};
t2460 = ct{1067};
t2461 = ct{1068};
t2463 = ct{1069};
t2464 = ct{1070};
t2466 = ct{1071};
t2467 = ct{1072};
t2469 = ct{1073};
t2470 = ct{1074};
t2471 = ct{1075};
t2472 = ct{1076};
t2474 = ct{1077};
t2477 = ct{1078};
t2478 = ct{1079};
t2480 = ct{1080};
t2481 = ct{1081};
t2482 = ct{1082};
t2483 = ct{1083};
t2484 = ct{1084};
t2485 = ct{1085};
t2486 = ct{1086};
t2487 = ct{1087};
t2489 = ct{1088};
t249 = ct{1089};
t2495 = ct{1090};
t2497 = ct{1091};
t25 = ct{1092};
t2500 = ct{1093};
t2502 = ct{1094};
t2503 = ct{1095};
t2505 = ct{1096};
t2507 = ct{1097};
t2508 = ct{1098};
t2509 = ct{1099};
t2510 = ct{1100};
t2511 = ct{1101};
t2512 = ct{1102};
t2513 = ct{1103};
t2517 = ct{1104};
t2518 = ct{1105};
t2519 = ct{1106};
t2520 = ct{1107};
t2521 = ct{1108};
t2522 = ct{1109};
t2523 = ct{1110};
t2524 = ct{1111};
t2525 = ct{1112};
t2526 = ct{1113};
t2527 = ct{1114};
t2530 = ct{1115};
t2531 = ct{1116};
t2532 = ct{1117};
t2533 = ct{1118};
t2535 = ct{1119};
t2536 = ct{1120};
t2537 = ct{1121};
t2539 = ct{1122};
t2540 = ct{1123};
t2541 = ct{1124};
t2543 = ct{1125};
t2544 = ct{1126};
t2545 = ct{1127};
t2546 = ct{1128};
t2548 = ct{1129};
t2549 = ct{1130};
t2550 = ct{1131};
t2552 = ct{1132};
t2553 = ct{1133};
t2554 = ct{1134};
t2555 = ct{1135};
t2556 = ct{1136};
t2560 = ct{1137};
t2562 = ct{1138};
t2563 = ct{1139};
t2564 = ct{1140};
t2565 = ct{1141};
t2566 = ct{1142};
t2567 = ct{1143};
t2568 = ct{1144};
t2569 = ct{1145};
t257 = ct{1146};
t2570 = ct{1147};
t2571 = ct{1148};
t2574 = ct{1149};
t2575 = ct{1150};
t2576 = ct{1151};
t2577 = ct{1152};
t2578 = ct{1153};
t2579 = ct{1154};
t258 = ct{1155};
t2580 = ct{1156};
t2581 = ct{1157};
t2582 = ct{1158};
t2585 = ct{1159};
t2586 = ct{1160};
t2587 = ct{1161};
t2588 = ct{1162};
t2589 = ct{1163};
t2590 = ct{1164};
t2595 = ct{1165};
t2597 = ct{1166};
t2598 = ct{1167};
t2599 = ct{1168};
t26 = ct{1169};
t2600 = ct{1170};
t2601 = ct{1171};
t2602 = ct{1172};
t2603 = ct{1173};
t2604 = ct{1174};
t2606 = ct{1175};
t2607 = ct{1176};
t2608 = ct{1177};
t2611 = ct{1178};
t2612 = ct{1179};
t2615 = ct{1180};
t2616 = ct{1181};
t2617 = ct{1182};
t2627 = ct{1183};
t263 = ct{1184};
t2633 = ct{1185};
t2634 = ct{1186};
t2636 = ct{1187};
t2639 = ct{1188};
t2640 = ct{1189};
t2641 = ct{1190};
t2654 = ct{1191};
t2655 = ct{1192};
t2656 = ct{1193};
t2659 = ct{1194};
t266 = ct{1195};
t2666 = ct{1196};
t2668 = ct{1197};
t2669 = ct{1198};
t2671 = ct{1199};
t2673 = ct{1200};
t2675 = ct{1201};
t2676 = ct{1202};
t2677 = ct{1203};
t2678 = ct{1204};
t2680 = ct{1205};
t2681 = ct{1206};
t2682 = ct{1207};
t2684 = ct{1208};
t2685 = ct{1209};
t2686 = ct{1210};
t2688 = ct{1211};
t2692 = ct{1212};
t2693 = ct{1213};
t2694 = ct{1214};
t2695 = ct{1215};
t2699 = ct{1216};
t270 = ct{1217};
t2702 = ct{1218};
t2703 = ct{1219};
t2705 = ct{1220};
t2706 = ct{1221};
t2707 = ct{1222};
t2708 = ct{1223};
t2719 = ct{1224};
t2720 = ct{1225};
t2721 = ct{1226};
t2722 = ct{1227};
t2723 = ct{1228};
t2724 = ct{1229};
t2725 = ct{1230};
t2726 = ct{1231};
t273 = ct{1232};
t2733 = ct{1233};
t2734 = ct{1234};
t2739 = ct{1235};
t274 = ct{1236};
t2741 = ct{1237};
t2742 = ct{1238};
t2743 = ct{1239};
t2744 = ct{1240};
t2748 = ct{1241};
t2749 = ct{1242};
t275 = ct{1243};
t2752 = ct{1244};
t2759 = ct{1245};
t276 = ct{1246};
t2760 = ct{1247};
t2761 = ct{1248};
t2762 = ct{1249};
t2764 = ct{1250};
t2768 = ct{1251};
t2769 = ct{1252};
t277 = ct{1253};
t2770 = ct{1254};
t2771 = ct{1255};
t2773 = ct{1256};
t2774 = ct{1257};
t2775 = ct{1258};
t2776 = ct{1259};
t278 = ct{1260};
t2781 = ct{1261};
t2782 = ct{1262};
t2783 = ct{1263};
t2784 = ct{1264};
t2786 = ct{1265};
t2787 = ct{1266};
t2788 = ct{1267};
t2789 = ct{1268};
t2791 = ct{1269};
t2792 = ct{1270};
t280 = ct{1271};
t2806 = ct{1272};
t2808 = ct{1273};
t2815 = ct{1274};
t2820 = ct{1275};
t2821 = ct{1276};
t2829 = ct{1277};
t2830 = ct{1278};
t2831 = ct{1279};
t284 = ct{1280};
t2840 = ct{1281};
t2842 = ct{1282};
t2844 = ct{1283};
t2845 = ct{1284};
t2847 = ct{1285};
t2848 = ct{1286};
t2849 = ct{1287};
t2853 = ct{1288};
t2854 = ct{1289};
t2861 = ct{1290};
t2862 = ct{1291};
t2863 = ct{1292};
t2864 = ct{1293};
t2866 = ct{1294};
t2868 = ct{1295};
t2869 = ct{1296};
t287 = ct{1297};
t2879 = ct{1298};
t2884 = ct{1299};
t2886 = ct{1300};
t2888 = ct{1301};
t2892 = ct{1302};
t2898 = ct{1303};
t2899 = ct{1304};
t29 = ct{1305};
t290 = ct{1306};
t2900 = ct{1307};
t2901 = ct{1308};
t2902 = ct{1309};
t2903 = ct{1310};
t2908 = ct{1311};
t291 = ct{1312};
t292 = ct{1313};
t2920 = ct{1314};
t2923 = ct{1315};
t2925 = ct{1316};
t2926 = ct{1317};
t2928 = ct{1318};
t2929 = ct{1319};
t2930 = ct{1320};
t2937 = ct{1321};
t294 = ct{1322};
t2940 = ct{1323};
t2943 = ct{1324};
t2945 = ct{1325};
t2948 = ct{1326};
t2949 = ct{1327};
t2950 = ct{1328};
t2951 = ct{1329};
t2952 = ct{1330};
t2960 = ct{1331};
t2961 = ct{1332};
t2962 = ct{1333};
t2963 = ct{1334};
t2964 = ct{1335};
t2966 = ct{1336};
t2967 = ct{1337};
t2968 = ct{1338};
t2969 = ct{1339};
t297 = ct{1340};
t2970 = ct{1341};
t2971 = ct{1342};
t2975 = ct{1343};
t2976 = ct{1344};
t2980 = ct{1345};
t2982 = ct{1346};
t2983 = ct{1347};
t2984 = ct{1348};
t2985 = ct{1349};
t2986 = ct{1350};
t2988 = ct{1351};
t2989 = ct{1352};
t299 = ct{1353};
t2991 = ct{1354};
t2992 = ct{1355};
t2993 = ct{1356};
t2996 = ct{1357};
t2997 = ct{1358};
t3 = ct{1359};
t30 = ct{1360};
t300 = ct{1361};
t3003 = ct{1362};
t3004 = ct{1363};
t3007 = ct{1364};
t3010 = ct{1365};
t3011 = ct{1366};
t3013 = ct{1367};
t3014 = ct{1368};
t3019 = ct{1369};
t302 = ct{1370};
t3020 = ct{1371};
t3021 = ct{1372};
t3023 = ct{1373};
t3024 = ct{1374};
t3025 = ct{1375};
t3027 = ct{1376};
t3028 = ct{1377};
t3029 = ct{1378};
t303 = ct{1379};
t3030 = ct{1380};
t3031 = ct{1381};
t3032 = ct{1382};
t3033 = ct{1383};
t3034 = ct{1384};
t3035 = ct{1385};
t3036 = ct{1386};
t3038 = ct{1387};
t3039 = ct{1388};
t304 = ct{1389};
t3043 = ct{1390};
t3045 = ct{1391};
t3046 = ct{1392};
t3047 = ct{1393};
t305 = ct{1394};
t3051 = ct{1395};
t3052 = ct{1396};
t3053 = ct{1397};
t3055 = ct{1398};
t3056 = ct{1399};
t3057 = ct{1400};
t306 = ct{1401};
t3060 = ct{1402};
t3061 = ct{1403};
t3062 = ct{1404};
t3063 = ct{1405};
t3065 = ct{1406};
t3066 = ct{1407};
t3069 = ct{1408};
t3070 = ct{1409};
t3071 = ct{1410};
t3072 = ct{1411};
t3073 = ct{1412};
t3075 = ct{1413};
t3077 = ct{1414};
t3078 = ct{1415};
t3079 = ct{1416};
t3080 = ct{1417};
t3082 = ct{1418};
t3083 = ct{1419};
t3085 = ct{1420};
t3087 = ct{1421};
t309 = ct{1422};
t3090 = ct{1423};
t3091 = ct{1424};
t3092 = ct{1425};
t3093 = ct{1426};
t3094 = ct{1427};
t3095 = ct{1428};
t3098 = ct{1429};
t3099 = ct{1430};
t310 = ct{1431};
t3103 = ct{1432};
t3104 = ct{1433};
t3105 = ct{1434};
t3108 = ct{1435};
t3109 = ct{1436};
t311 = ct{1437};
t3112 = ct{1438};
t3113 = ct{1439};
t3119 = ct{1440};
t3120 = ct{1441};
t3123 = ct{1442};
t3124 = ct{1443};
t3126 = ct{1444};
t3127 = ct{1445};
t313 = ct{1446};
t3130 = ct{1447};
t3131 = ct{1448};
t3132 = ct{1449};
t3133 = ct{1450};
t3139 = ct{1451};
t314 = ct{1452};
t3140 = ct{1453};
t3142 = ct{1454};
t3143 = ct{1455};
t3145 = ct{1456};
t3146 = ct{1457};
t3148 = ct{1458};
t3149 = ct{1459};
t315 = ct{1460};
t3150 = ct{1461};
t3151 = ct{1462};
t3152 = ct{1463};
t3156 = ct{1464};
t3157 = ct{1465};
t3158 = ct{1466};
t316 = ct{1467};
t3160 = ct{1468};
t3163 = ct{1469};
t3165 = ct{1470};
t3167 = ct{1471};
t3170 = ct{1472};
t3171 = ct{1473};
t3172 = ct{1474};
t3173 = ct{1475};
t3174 = ct{1476};
t3177 = ct{1477};
t3178 = ct{1478};
t318 = ct{1479};
t3180 = ct{1480};
t3182 = ct{1481};
t3183 = ct{1482};
t3184 = ct{1483};
t3186 = ct{1484};
t3187 = ct{1485};
t319 = ct{1486};
t3190 = ct{1487};
t3191 = ct{1488};
t3194 = ct{1489};
t3197 = ct{1490};
t3199 = ct{1491};
t320 = ct{1492};
t3206 = ct{1493};
t3207 = ct{1494};
t3208 = ct{1495};
t3219 = ct{1496};
t322 = ct{1497};
t3228 = ct{1498};
t3230 = ct{1499};
t3234 = ct{1500};
t3236 = ct{1501};
t324 = ct{1502};
t3240 = ct{1503};
t3241 = ct{1504};
t3242 = ct{1505};
t3243 = ct{1506};
t3245 = ct{1507};
t325 = ct{1508};
t3250 = ct{1509};
t3251 = ct{1510};
t3252 = ct{1511};
t3253 = ct{1512};
t3254 = ct{1513};
t3256 = ct{1514};
t3257 = ct{1515};
t3260 = ct{1516};
t3265 = ct{1517};
t3272 = ct{1518};
t3273 = ct{1519};
t3274 = ct{1520};
t3275 = ct{1521};
t3276 = ct{1522};
t3277 = ct{1523};
t3278 = ct{1524};
t3279 = ct{1525};
t328 = ct{1526};
t3280 = ct{1527};
t3282 = ct{1528};
t3283 = ct{1529};
t3284 = ct{1530};
t3285 = ct{1531};
t3286 = ct{1532};
t3287 = ct{1533};
t3288 = ct{1534};
t3289 = ct{1535};
t3290 = ct{1536};
t3291 = ct{1537};
t3292 = ct{1538};
t3293 = ct{1539};
t3295 = ct{1540};
t3296 = ct{1541};
t3297 = ct{1542};
t3298 = ct{1543};
t3299 = ct{1544};
t3301 = ct{1545};
t3302 = ct{1546};
t3303 = ct{1547};
t3304 = ct{1548};
t3306 = ct{1549};
t3307 = ct{1550};
t3308 = ct{1551};
t3309 = ct{1552};
t3310 = ct{1553};
t3312 = ct{1554};
t3313 = ct{1555};
t3314 = ct{1556};
t3315 = ct{1557};
t3317 = ct{1558};
t3318 = ct{1559};
t3320 = ct{1560};
t3321 = ct{1561};
t3324 = ct{1562};
t3325 = ct{1563};
t3326 = ct{1564};
t3327 = ct{1565};
t3328 = ct{1566};
t3329 = ct{1567};
t333 = ct{1568};
t3331 = ct{1569};
t3333 = ct{1570};
t3334 = ct{1571};
t3335 = ct{1572};
t3338 = ct{1573};
t3339 = ct{1574};
t3342 = ct{1575};
t3343 = ct{1576};
t3346 = ct{1577};
t3347 = ct{1578};
t3350 = ct{1579};
t336 = ct{1580};
t3362 = ct{1581};
t3363 = ct{1582};
t3364 = ct{1583};
t3365 = ct{1584};
t3366 = ct{1585};
t3367 = ct{1586};
t3368 = ct{1587};
t3369 = ct{1588};
t337 = ct{1589};
t3371 = ct{1590};
t3372 = ct{1591};
t3373 = ct{1592};
t3374 = ct{1593};
t3375 = ct{1594};
t3376 = ct{1595};
t3377 = ct{1596};
t3378 = ct{1597};
t3380 = ct{1598};
t3381 = ct{1599};
t3382 = ct{1600};
t3383 = ct{1601};
t3384 = ct{1602};
t3387 = ct{1603};
t3390 = ct{1604};
t3391 = ct{1605};
t3392 = ct{1606};
t3393 = ct{1607};
t3394 = ct{1608};
t3395 = ct{1609};
t3396 = ct{1610};
t3397 = ct{1611};
t3398 = ct{1612};
t3399 = ct{1613};
t34 = ct{1614};
t340 = ct{1615};
t3400 = ct{1616};
t3402 = ct{1617};
t3403 = ct{1618};
t3404 = ct{1619};
t3405 = ct{1620};
t3406 = ct{1621};
t3407 = ct{1622};
t3408 = ct{1623};
t3409 = ct{1624};
t3410 = ct{1625};
t3411 = ct{1626};
t3412 = ct{1627};
t3413 = ct{1628};
t3416 = ct{1629};
t3417 = ct{1630};
t3418 = ct{1631};
t3420 = ct{1632};
t3421 = ct{1633};
t3422 = ct{1634};
t3423 = ct{1635};
t3424 = ct{1636};
t3425 = ct{1637};
t3426 = ct{1638};
t3427 = ct{1639};
t3430 = ct{1640};
t3431 = ct{1641};
t3432 = ct{1642};
t3433 = ct{1643};
t3434 = ct{1644};
t3435 = ct{1645};
t3436 = ct{1646};
t3437 = ct{1647};
t3439 = ct{1648};
t344 = ct{1649};
t3440 = ct{1650};
t3441 = ct{1651};
t3442 = ct{1652};
t3443 = ct{1653};
t3444 = ct{1654};
t3445 = ct{1655};
t3446 = ct{1656};
t3447 = ct{1657};
t3449 = ct{1658};
t3450 = ct{1659};
t3453 = ct{1660};
t3454 = ct{1661};
t3455 = ct{1662};
t3456 = ct{1663};
t3457 = ct{1664};
t3458 = ct{1665};
t346 = ct{1666};
t3462 = ct{1667};
t3463 = ct{1668};
t3464 = ct{1669};
t3465 = ct{1670};
t3466 = ct{1671};
t3467 = ct{1672};
t3468 = ct{1673};
t3469 = ct{1674};
t347 = ct{1675};
t3470 = ct{1676};
t3471 = ct{1677};
t3472 = ct{1678};
t3473 = ct{1679};
t3474 = ct{1680};
t3475 = ct{1681};
t3476 = ct{1682};
t3479 = ct{1683};
t348 = ct{1684};
t3480 = ct{1685};
t3481 = ct{1686};
t3483 = ct{1687};
t3485 = ct{1688};
t3487 = ct{1689};
t3488 = ct{1690};
t3489 = ct{1691};
t349 = ct{1692};
t3490 = ct{1693};
t3491 = ct{1694};
t3492 = ct{1695};
t3493 = ct{1696};
t3494 = ct{1697};
t3496 = ct{1698};
t3497 = ct{1699};
t3498 = ct{1700};
t3499 = ct{1701};
t350 = ct{1702};
t3500 = ct{1703};
t3501 = ct{1704};
t3502 = ct{1705};
t3503 = ct{1706};
t3504 = ct{1707};
t3505 = ct{1708};
t3506 = ct{1709};
t3507 = ct{1710};
t3509 = ct{1711};
t3510 = ct{1712};
t3511 = ct{1713};
t3513 = ct{1714};
t3514 = ct{1715};
t3515 = ct{1716};
t3516 = ct{1717};
t3517 = ct{1718};
t3518 = ct{1719};
t352 = ct{1720};
t3521 = ct{1721};
t3522 = ct{1722};
t3523 = ct{1723};
t3527 = ct{1724};
t3528 = ct{1725};
t3529 = ct{1726};
t353 = ct{1727};
t3530 = ct{1728};
t3531 = ct{1729};
t3532 = ct{1730};
t3533 = ct{1731};
t3535 = ct{1732};
t3536 = ct{1733};
t3538 = ct{1734};
t3539 = ct{1735};
t3542 = ct{1736};
t3543 = ct{1737};
t3544 = ct{1738};
t3545 = ct{1739};
t3546 = ct{1740};
t3547 = ct{1741};
t3549 = ct{1742};
t3550 = ct{1743};
t3551 = ct{1744};
t3552 = ct{1745};
t3554 = ct{1746};
t3556 = ct{1747};
t3557 = ct{1748};
t3559 = ct{1749};
t356 = ct{1750};
t3560 = ct{1751};
t3562 = ct{1752};
t3563 = ct{1753};
t3564 = ct{1754};
t3567 = ct{1755};
t3568 = ct{1756};
t3569 = ct{1757};
t357 = ct{1758};
t3571 = ct{1759};
t3572 = ct{1760};
t3573 = ct{1761};
t3574 = ct{1762};
t3577 = ct{1763};
t3578 = ct{1764};
t358 = ct{1765};
t3582 = ct{1766};
t3583 = ct{1767};
t3584 = ct{1768};
t3585 = ct{1769};
t3586 = ct{1770};
t3587 = ct{1771};
t3589 = ct{1772};
t359 = ct{1773};
t3590 = ct{1774};
t3592 = ct{1775};
t3593 = ct{1776};
t3596 = ct{1777};
t3597 = ct{1778};
t3599 = ct{1779};
t3602 = ct{1780};
t3603 = ct{1781};
t3604 = ct{1782};
t3605 = ct{1783};
t3606 = ct{1784};
t3607 = ct{1785};
t3608 = ct{1786};
t3609 = ct{1787};
t361 = ct{1788};
t3610 = ct{1789};
t3611 = ct{1790};
t3612 = ct{1791};
t3614 = ct{1792};
t3615 = ct{1793};
t3616 = ct{1794};
t3617 = ct{1795};
t3618 = ct{1796};
t3619 = ct{1797};
t362 = ct{1798};
t3620 = ct{1799};
t3625 = ct{1800};
t3630 = ct{1801};
t3631 = ct{1802};
t3633 = ct{1803};
t3634 = ct{1804};
t3635 = ct{1805};
t3636 = ct{1806};
t3637 = ct{1807};
t3638 = ct{1808};
t3642 = ct{1809};
t3644 = ct{1810};
t3648 = ct{1811};
t365 = ct{1812};
t3652 = ct{1813};
t3653 = ct{1814};
t3654 = ct{1815};
t3655 = ct{1816};
t3656 = ct{1817};
t3657 = ct{1818};
t3658 = ct{1819};
t3659 = ct{1820};
t3660 = ct{1821};
t3662 = ct{1822};
t3663 = ct{1823};
t3666 = ct{1824};
t3667 = ct{1825};
t3668 = ct{1826};
t3676 = ct{1827};
t368 = ct{1828};
t3681 = ct{1829};
t3682 = ct{1830};
t3687 = ct{1831};
t3688 = ct{1832};
t369 = ct{1833};
t3690 = ct{1834};
t3691 = ct{1835};
t3693 = ct{1836};
t3694 = ct{1837};
t3695 = ct{1838};
t3696 = ct{1839};
t3697 = ct{1840};
t3699 = ct{1841};
t3700 = ct{1842};
t3701 = ct{1843};
t3702 = ct{1844};
t3704 = ct{1845};
t3705 = ct{1846};
t3706 = ct{1847};
t3707 = ct{1848};
t3708 = ct{1849};
